simulink model "IPC4M"  (R2015a)
settings: Solver=ode3  SolverMode=SingleTasking  StartTime=0.0  StopTime=10.0  FixedStep=1e-2  RelTol=1e-7
values from neighbouring files (symbols this model uses):
  d1 = 70    [IPC4Minit.m]
  d2 = 70    [IPC4Minit.m]
  d3 = 70    [IPC4Minit.m]
  d4 = 70    [IPC4Minit.m]
  delta1 = 9    [IPC4Minit.m]
  delta2 = 9    [IPC4Minit.m]
  delta3 = 9    [IPC4Minit.m]
  delta4 = 9    [IPC4Minit.m]
  g = [0;0;-9.81]    [IPC4Minit.m]
  j0 = 10    [IPC4Minit.m]
  j1 = 10    [IPC4Minit.m]
  j1d = 1.00*j1    (= 10)    [IPC4Minit.m]
  j2 = 10    [IPC4Minit.m]
  j2d = 1.00*j2    (= 10)    [IPC4Minit.m]
  j3 = 10    [IPC4Minit.m]
  j3d = 1.00*j3    (= 10)    [IPC4Minit.m]
  j4 = 10    [IPC4Minit.m]
  j4d = 1.00*j4    (= 10)    [IPC4Minit.m]
  k1 = 2000    [IPC4Minit.m]
  k2 = 2000    [IPC4Minit.m]
  k3 = 2000    [IPC4Minit.m]
  k4 = 2000    [IPC4Minit.m]
  kappa1 = 10    [IPC4Minit.m]
  kappa2 = 10    [IPC4Minit.m]
  kappa3 = 10    [IPC4Minit.m]
  kappa4 = 10    [IPC4Minit.m]
  Kc = 150    [IPC4Minit.m]
  l = [1 1 1 1]    [IPC4Minit.m]
  m0 = 10    [IPC4Minit.m]
  m1 = 10    [IPC4Minit.m]
  m1d = 0.00*m1    (= 0)    [IPC4Minit.m]
  m2 = 10    [IPC4Minit.m]
  m2d = 0.00*m2    (= 0)    [IPC4Minit.m]
  m3 = 10    [IPC4Minit.m]
  m3d = 0.00*m3    (= 0)    [IPC4Minit.m]
  m4 = 10    [IPC4Minit.m]
  m4d = 0.00*m4    (= 0)    [IPC4Minit.m]
libraries: aerolibutil x11, dspinverses x3
(part 2 of 3)

== matlab function IPC4M/Inverse Dynamics/Weighted Generalized Inverse2 ==
  data: x input; Ginv output; r parameter
function Ginv = GraspInverse(x,r)
r1 = quatrot(x(4:7),r(1:3));
r2 = quatrot(x(4:7),r(4:6));
r3 = quatrot(x(4:7),r(7:9));
r4 = quatrot(x(4:7),r(10:12));
x1 = r1(1);
y1 = r1(2);
z1 = r1(3);
x2 = r2(1);
y2 = r2(2);
z2 = r2(3);
x3 = r3(1);
y3 = r3(2);
z3 = r3(3);
x4 = r4(1);
y4 = r4(2);
z4 = r4(3);

J4inv = [(4*(2*x1^2*x2^2 + 2*x1^2*x3^2 + 2*x1^2*x4^2 + 2*x2^2*x3^2 + 2*x2^2*x4^2 + 2*x3^2*x4^2 + x1^2*y1^2 + x1^2*y2^2 + x2^2*y1^2 + x1^2*y3^2 + x2^2*y2^2 + x3^2*y1^2 + x1^2*y4^2 + x2^2*y3^2 + x3^2*y2^2 + x4^2*y1^2 + x2^2*y4^2 + x3^2*y3^2 + x4^2*y2^2 + x3^2*y4^2 + x4^2*y3^2 + x4^2*y4^2 + x1^2*z1^2 + x1^2*z2^2 + x2^2*z1^2 + x1^2*z3^2 + x2^2*z2^2 + x3^2*z1^2 + x1^2*z4^2 + x2^2*z3^2 + x3^2*z2^2 + x4^2*z1^2 + x2^2*z4^2 + x3^2*z3^2 + x4^2*z2^2 + x3^2*z4^2 + x4^2*z3^2 + x4^2*z4^2 + y1^2*z2^2 + y2^2*z1^2 + y1^2*z3^2 + y3^2*z1^2 + y1^2*z4^2 + y2^2*z3^2 + y3^2*z2^2 + y4^2*z1^2 + y2^2*z4^2 + y4^2*z2^2 + y3^2*z4^2 + y4^2*z3^2 + 8*x1^2 + 8*x2^2 + x1^4 + 8*x3^2 + x2^4 + 8*x4^2 + x3^4 + x4^4 + 4*y1^2 + 4*y2^2 + 4*y3^2 + 4*y4^2 + 4*z1^2 + 4*z2^2 + 4*z3^2 + 4*z4^2 - 2*y1*y2*z1*z2 - 2*y1*y3*z1*z3 - 2*y1*y4*z1*z4 - 2*y2*y3*z2*z3 - 2*y2*y4*z2*z4 - 2*y3*y4*z3*z4 + 16))/(8*x1^2*x2^2 + 8*x1^2*x3^2 + 8*x1^2*x4^2 + 8*x2^2*x3^2 + 8*x2^2*x4^2 + 8*x3^2*x4^2 + 8*x1^2*y1^2 + 12*x1^2*y2^2 + 12*x2^2*y1^2 + 12*x1^2*y3^2 + 8*x2^2*y2^2 + 12*x3^2*y1^2 + x1^2*y2^4 + 12*x1^2*y4^2 + x2^2*y1^4 + 12*x2^2*y3^2 + x1^4*y2^2 + 12*x3^2*y2^2 + x2^4*y1^2 + 12*x4^2*y1^2 + x1^2*y3^4 + 12*x2^2*y4^2 + x1^4*y3^2 + x3^2*y1^4 + 8*x3^2*y3^2 + 12*x4^2*y2^2 + x3^4*y1^2 + x1^2*y4^4 + x2^2*y3^4 + x1^4*y4^2 + x3^2*y2^4 + 12*x3^2*y4^2 + x2^4*y3^2 + x4^2*y1^4 + 12*x4^2*y3^2 + x3^4*y2^2 + x4^4*y1^2 + x2^2*y4^4 + x2^4*y4^2 + x4^2*y2^4 + 8*x4^2*y4^2 + x4^4*y2^2 + x3^2*y4^4 + x4^2*y3^4 + x3^4*y4^2 + x4^4*y3^2 + 8*x1^2*z1^2 + 12*x1^2*z2^2 + 12*x2^2*z1^2 + 8*y1^2*y2^2 + 12*x1^2*z3^2 + 8*x2^2*z2^2 + 12*x3^2*z1^2 + 8*y1^2*y3^2 + x1^2*z2^4 + 12*x1^2*z4^2 + x2^2*z1^4 + 12*x2^2*z3^2 + x1^4*z2^2 + 12*x3^2*z2^2 + x2^4*z1^2 + 12*x4^2*z1^2 + 8*y1^2*y4^2 + 8*y2^2*y3^2 + x1^2*z3^4 + 12*x2^2*z4^2 + x1^4*z3^2 + x3^2*z1^4 + 8*x3^2*z3^2 + 12*x4^2*z2^2 + x3^4*z1^2 + 8*y2^2*y4^2 + x1^2*z4^4 + x2^2*z3^4 + x1^4*z4^2 + x3^2*z2^4 + 12*x3^2*z4^2 + x2^4*z3^2 + x4^2*z1^4 + 12*x4^2*z3^2 + x3^4*z2^2 + x4^4*z1^2 + 8*y3^2*y4^2 + x2^2*z4^4 + x2^4*z4^2 + x4^2*z2^4 + 8*x4^2*z4^2 + x4^4*z2^2 + x3^2*z4^4 + x4^2*z3^4 + x3^4*z4^2 + x4^4*z3^2 + 8*y1^2*z1^2 + 12*y1^2*z2^2 + 12*y2^2*z1^2 + 12*y1^2*z3^2 + 8*y2^2*z2^2 + 12*y3^2*z1^2 + y1^2*z2^4 + 12*y1^2*z4^2 + y2^2*z1^4 + 12*y2^2*z3^2 + y1^4*z2^2 + 12*y3^2*z2^2 + y2^4*z1^2 + 12*y4^2*z1^2 + y1^2*z3^4 + 12*y2^2*z4^2 + y1^4*z3^2 + y3^2*z1^4 + 8*y3^2*z3^2 + 12*y4^2*z2^2 + y3^4*z1^2 + y1^2*z4^4 + y2^2*z3^4 + y1^4*z4^2 + y3^2*z2^4 + 12*y3^2*z4^2 + y2^4*z3^2 + y4^2*z1^4 + 12*y4^2*z3^2 + y3^4*z2^2 + y4^4*z1^2 + y2^2*z4^4 + y2^4*z4^2 + y4^2*z2^4 + 8*y4^2*z4^2 + y4^4*z2^2 + y3^2*z4^4 + y4^2*z3^4 + y3^4*z4^2 + y4^4*z3^2 + 8*z1^2*z2^2 + 8*z1^2*z3^2 + 8*z1^2*z4^2 + 8*z2^2*z3^2 + 8*z2^2*z4^2 + 8*z3^2*z4^2 + 32*x1^2 + 32*x2^2 + 4*x1^4 + 32*x3^2 + 4*x2^4 + 32*x4^2 + 4*x3^4 + 4*x4^4 + 32*y1^2 + 32*y2^2 + 4*y1^4 + 32*y3^2 + 4*y2^4 + 32*y4^2 + 4*y3^4 + 4*y4^4 + 32*z1^2 + 32*z2^2 + 4*z1^4 + 32*z3^2 + 4*z2^4 + 32*z4^2 + 4*z3^4 + 4*z4^4 + x1^2*x2^2*y1^2 + x1^2*x2^2*y2^2 + x1^2*x3^2*y1^2 + 2*x1^2*x2^2*y3^2 + 2*x1^2*x3^2*y2^2 + x1^2*x4^2*y1^2 + 2*x2^2*x3^2*y1^2 + 2*x1^2*x2^2*y4^2 + x1^2*x3^2*y3^2 + 2*x1^2*x4^2*y2^2 + x2^2*x3^2*y2^2 + 2*x2^2*x4^2*y1^2 + 2*x1^2*x3^2*y4^2 + 2*x1^2*x4^2*y3^2 + x2^2*x3^2*y3^2 + x2^2*x4^2*y2^2 + 2*x3^2*x4^2*y1^2 + x1^2*x4^2*y4^2 + 2*x2^2*x3^2*y4^2 + 2*x2^2*x4^2*y3^2 + 2*x3^2*x4^2*y2^2 + x2^2*x4^2*y4^2 + x3^2*x4^2*y3^2 + x3^2*x4^2*y4^2 + x1^2*x2^2*z1^2 + x1^2*y1^2*y2^2 + x1^2*x2^2*z2^2 + x1^2*x3^2*z1^2 + x1^2*y1^2*y3^2 + x2^2*y1^2*y2^2 + 2*x1^2*x2^2*z3^2 + 2*x1^2*x3^2*z2^2 + x1^2*x4^2*z1^2 + x1^2*y1^2*y4^2 + 2*x1^2*y2^2*y3^2 + 2*x2^2*x3^2*z1^2 + 2*x2^2*y1^2*y3^2 + 2*x3^2*y1^2*y2^2 + 2*x1^2*x2^2*z4^2 + x1^2*x3^2*z3^2 + 2*x1^2*x4^2*z2^2 + 2*x1^2*y2^2*y4^2 + x2^2*x3^2*z2^2 + 2*x2^2*x4^2*z1^2 + 2*x2^2*y1^2*y4^2 + x2^2*y2^2*y3^2 + x3^2*y1^2*y3^2 + 2*x4^2*y1^2*y2^2 + 2*x1^2*x3^2*z4^2 + 2*x1^2*x4^2*z3^2 + 2*x1^2*y3^2*y4^2 + x2^2*x3^2*z3^2 + x2^2*x4^2*z2^2 + x2^2*y2^2*y4^2 + 2*x3^2*x4^2*z1^2 + 2*x3^2*y1^2*y4^2 + x3^2*y2^2*y3^2 + 2*x4^2*y1^2*y3^2 + x1^2*x4^2*z4^2 + 2*x2^2*x3^2*z4^2 + 2*x2^2*x4^2*z3^2 + 2*x2^2*y3^2*y4^2 + 2*x3^2*x4^2*z2^2 + 2*x3^2*y2^2*y4^2 + x4^2*y1^2*y4^2 + 2*x4^2*y2^2*y3^2 + x2^2*x4^2*z4^2 + x3^2*x4^2*z3^2 + x3^2*y3^2*y4^2 + x4^2*y2^2*y4^2 + x3^2*x4^2*z4^2 + x4^2*y3^2*y4^2 + 2*x1^2*y1^2*z2^2 + 2*x1^2*y2^2*z1^2 + 2*x2^2*y1^2*z1^2 + 2*x1^2*y1^2*z3^2 + 2*x1^2*y2^2*z2^2 + 2*x1^2*y3^2*z1^2 + 2*x2^2*y1^2*z2^2 + 2*x2^2*y2^2*z1^2 + 2*x3^2*y1^2*z1^2 + 2*x1^2*y1^2*z4^2 + 2*x1^2*y2^2*z3^2 + 2*x1^2*y3^2*z2^2 + 2*x1^2*y4^2*z1^2 + 2*x2^2*y1^2*z3^2 + 2*x2^2*y3^2*z1^2 + 2*x3^2*y1^2*z2^2 + 2*x3^2*y2^2*z1^2 + 2*x4^2*y1^2*z1^2 + 2*x1^2*y2^2*z4^2 + 2*x1^2*y3^2*z3^2 + 2*x1^2*y4^2*z2^2 + 2*x2^2*y1^2*z4^2 + 2*x2^2*y2^2*z3^2 + 2*x2^2*y3^2*z2^2 + 2*x2^2*y4^2*z1^2 + 2*x3^2*y1^2*z3^2 + 2*x3^2*y2^2*z2^2 + 2*x3^2*y3^2*z1^2 + 2*x4^2*y1^2*z2^2 + 2*x4^2*y2^2*z1^2 + 2*x1^2*y3^2*z4^2 + 2*x1^2*y4^2*z3^2 + 2*x2^2*y2^2*z4^2 + 2*x2^2*y3^2*z3^2 + 2*x2^2*y4^2*z2^2 + 2*x3^2*y1^2*z4^2 + 2*x3^2*y2^2*z3^2 + 2*x3^2*y3^2*z2^2 + 2*x3^2*y4^2*z1^2 + 2*x4^2*y1^2*z3^2 + 2*x4^2*y2^2*z2^2 + 2*x4^2*y3^2*z1^2 + 2*x1^2*y4^2*z4^2 + 2*x2^2*y3^2*z4^2 + 2*x2^2*y4^2*z3^2 + 2*x3^2*y2^2*z4^2 + 2*x3^2*y4^2*z2^2 + 2*x4^2*y1^2*z4^2 + 2*x4^2*y2^2*z3^2 + 2*x4^2*y3^2*z2^2 + 2*x4^2*y4^2*z1^2 + 2*x2^2*y4^2*z4^2 + 2*x3^2*y3^2*z4^2 + 2*x3^2*y4^2*z3^2 + 2*x4^2*y2^2*z4^2 + 2*x4^2*y3^2*z3^2 + 2*x4^2*y4^2*z2^2 + 2*x3^2*y4^2*z4^2 + 2*x4^2*y3^2*z4^2 + 2*x4^2*y4^2*z3^2 + x1^2*z1^2*z2^2 + y1^2*y2^2*z1^2 + x1^2*z1^2*z3^2 + x2^2*z1^2*z2^2 + y1^2*y2^2*z2^2 + y1^2*y3^2*z1^2 + x1^2*z1^2*z4^2 + 2*x1^2*z2^2*z3^2 + 2*x2^2*z1^2*z3^2 + 2*x3^2*z1^2*z2^2 + 2*y1^2*y2^2*z3^2 + 2*y1^2*y3^2*z2^2 + y1^2*y4^2*z1^2 + 2*y2^2*y3^2*z1^2 + 2*x1^2*z2^2*z4^2 + 2*x2^2*z1^2*z4^2 + x2^2*z2^2*z3^2 + x3^2*z1^2*z3^2 + 2*x4^2*z1^2*z2^2 + 2*y1^2*y2^2*z4^2 + y1^2*y3^2*z3^2 + 2*y1^2*y4^2*z2^2 + y2^2*y3^2*z2^2 + 2*y2^2*y4^2*z1^2 + 2*x1^2*z3^2*z4^2 + x2^2*z2^2*z4^2 + 2*x3^2*z1^2*z4^2 + x3^2*z2^2*z3^2 + 2*x4^2*z1^2*z3^2 + 2*y1^2*y3^2*z4^2 + 2*y1^2*y4^2*z3^2 + y2^2*y3^2*z3^2 + y2^2*y4^2*z2^2 + 2*y3^2*y4^2*z1^2 + 2*x2^2*z3^2*z4^2 + 2*x3^2*z2^2*z4^2 + x4^2*z1^2*z4^2 + 2*x4^2*z2^2*z3^2 + y1^2*y4^2*z4^2 + 2*y2^2*y3^2*z4^2 + 2*y2^2*y4^2*z3^2 + 2*y3^2*y4^2*z2^2 + x3^2*z3^2*z4^2 + x4^2*z2^2*z4^2 + y2^2*y4^2*z4^2 + y3^2*y4^2*z3^2 + x4^2*z3^2*z4^2 + y3^2*y4^2*z4^2 + y1^2*z1^2*z2^2 + y1^2*z1^2*z3^2 + y2^2*z1^2*z2^2 + y1^2*z1^2*z4^2 + 2*y1^2*z2^2*z3^2 + 2*y2^2*z1^2*z3^2 + 2*y3^2*z1^2*z2^2 + 2*y1^2*z2^2*z4^2 + 2*y2^2*z1^2*z4^2 + y2^2*z2^2*z3^2 + y3^2*z1^2*z3^2 + 2*y4^2*z1^2*z2^2 + 2*y1^2*z3^2*z4^2 + y2^2*z2^2*z4^2 + 2*y3^2*z1^2*z4^2 + y3^2*z2^2*z3^2 + 2*y4^2*z1^2*z3^2 + 2*y2^2*z3^2*z4^2 + 2*y3^2*z2^2*z4^2 + y4^2*z1^2*z4^2 + 2*y4^2*z2^2*z3^2 + y3^2*z3^2*z4^2 + y4^2*z2^2*z4^2 + y4^2*z3^2*z4^2 - 8*x1*x2*y1*y2 - 8*x1*x3*y1*y3 - 8*x1*x4*y1*y4 - 8*x2*x3*y2*y3 - 8*x2*x4*y2*y4 - 8*x3*x4*y3*y4 - 8*x1*x2*z1*z2 - 8*x1*x3*z1*z3 - 8*x1*x4*z1*z4 - 8*x2*x3*z2*z3 - 8*x2*x4*z2*z4 - 8*x3*x4*z3*z4 - 8*y1*y2*z1*z2 - 8*y1*y3*z1*z3 - 8*y1*y4*z1*z4 - 8*y2*y3*z2*z3 - 8*y2*y4*z2*z4 - 8*y3*y4*z3*z4 - 2*x1*x2*y1*y2^3 - 2*x1*x2*y1^3*y2 - 2*x1*x2^3*y1*y2 - 2*x1^3*x2*y1*y2 - 2*x1*x3*y1*y3^3 - 2*x1*x3*y1^3*y3 - 2*x1*x3^3*y1*y3 - 2*x1^3*x3*y1*y3 - 2*x1*x4*y1*y4^3 - 2*x1*x4*y1^3*y4 - 2*x1*x4^3*y1*y4 - 2*x2*x3*y2*y3^3 - 2*x2*x3*y2^3*y3 - 2*x2*x3^3*y2*y3 - 2*x1^3*x4*y1*y4 - 2*x2^3*x3*y2*y3 - 2*x2*x4*y2*y4^3 - 2*x2*x4*y2^3*y4 - 2*x2*x4^3*y2*y4 - 2*x2^3*x4*y2*y4 - 2*x3*x4*y3*y4^3 - 2*x3*x4*y3^3*y4 - 2*x3*x4^3*y3*y4 - 2*x3^3*x4*y3*y4 - 2*x1*x2*z1*z2^3 - 2*x1*x2*z1^3*z2 - 2*x1*x2^3*z1*z2 - 2*x1^3*x2*z1*z2 - 2*x1*x3*z1*z3^3 - 2*x1*x3*z1^3*z3 - 2*x1*x3^3*z1*z3 - 2*x1^3*x3*z1*z3 - 2*x1*x4*z1*z4^3 - 2*x1*x4*z1^3*z4 - 2*x1*x4^3*z1*z4 - 2*x2*x3*z2*z3^3 - 2*x2*x3*z2^3*z3 - 2*x2*x3^3*z2*z3 - 2*x1^3*x4*z1*z4 - 2*x2^3*x3*z2*z3 - 2*x2*x4*z2*z4^3 - 2*x2*x4*z2^3*z4 - 2*x2*x4^3*z2*z4 - 2*x2^3*x4*z2*z4 - 2*x3*x4*z3*z4^3 - 2*x3*x4*z3^3*z4 - 2*x3*x4^3*z3*z4 - 2*x3^3*x4*z3*z4 - 2*y1*y2*z1*z2^3 - 2*y1*y2*z1^3*z2 - 2*y1*y2^3*z1*z2 - 2*y1^3*y2*z1*z2 - 2*y1*y3*z1*z3^3 - 2*y1*y3*z1^3*z3 - 2*y1*y3^3*z1*z3 - 2*y1^3*y3*z1*z3 - 2*y1*y4*z1*z4^3 - 2*y1*y4*z1^3*z4 - 2*y1*y4^3*z1*z4 - 2*y2*y3*z2*z3^3 - 2*y2*y3*z2^3*z3 - 2*y2*y3^3*z2*z3 - 2*y1^3*y4*z1*z4 - 2*y2^3*y3*z2*z3 - 2*y2*y4*z2*z4^3 - 2*y2*y4*z2^3*z4 - 2*y2*y4^3*z2*z4 - 2*y2^3*y4*z2*z4 - 2*y3*y4*z3*z4^3 - 2*y3*y4*z3^3*z4 - 2*y3*y4^3*z3*z4 - 2*y3^3*y4*z3*z4 - 2*x1*x2*x3^2*y1*y2 - 2*x1*x2*x4^2*y1*y2 - 2*x1*x2^2*x3*y1*y3 - 2*x1^2*x2*x3*y2*y3 - 2*x1*x3*x4^2*y1*y3 - 2*x1*x2^2*x4*y1*y4 - 2*x1*x3^2*x4*y1*y4 - 2*x1^2*x2*x4*y2*y4 - 2*x2*x3*x4^2*y2*y3 - 2*x2*x3^2*x4*y2*y4 - 2*x1^2*x3*x4*y3*y4 - 2*x2^2*x3*x4*y3*y4 - 2*x1*x2*y1*y2*y3^2 - 2*x1*x2*y1*y2*y4^2 - 2*x1*x3*y1*y2^2*y3 - 2*x2*x3*y1^2*y2*y3 - 2*x1*x3*y1*y3*y4^2 - 2*x1*x4*y1*y2^2*y4 - 2*x1*x4*y1*y3^2*y4 - 2*x2*x4*y1^2*y2*y4 - 2*x2*x3*y2*y3*y4^2 - 2*x2*x4*y2*y3^2*y4 - 2*x3*x4*y1^2*y3*y4 - 2*x3*x4*y2^2*y3*y4 - 2*x1*x2*y1*y2*z1^2 - 2*x1*x2*y1*y2*z2^2 - 2*x1*x2*x3^2*z1*z2 - 2*x1*x3*y1*y3*z1^2 - 2*x1*x2*x4^2*z1*z2 - 2*x1*x2^2*x3*z1*z3 - 2*x1*x3*y1*y3*z3^2 - 2*x1*x4*y1*y4*z1^2 - 2*x1^2*x2*x3*z2*z3 - 2*x1*x3*x4^2*z1*z3 - 2*x1*x2^2*x4*z1*z4 - 2*x2*x3*y2*y3*z2^2 - 2*x1*x3^2*x4*z1*z4 - 2*x2*x3*y2*y3*z3^2 - 2*x1^2*x2*x4*z2*z4 - 2*x1*x4*y1*y4*z4^2 - 2*x2*x3*x4^2*z2*z3 - 2*x2*x4*y2*y4*z2^2 - 2*x2*x3^2*x4*z2*z4 - 2*x1^2*x3*x4*z3*z4 - 2*x2*x4*y2*y4*z4^2 - 2*x2^2*x3*x4*z3*z4 - 2*x3*x4*y3*y4*z3^2 - 2*x3*x4*y3*y4*z4^2 - 2*x1*x2*y1^2*z1*z2 - 2*x1*x2*y2^2*z1*z2 - 2*x1*x3*y1^2*z1*z3 - 2*x1*x3*y3^2*z1*z3 - 2*x1*x4*y1^2*z1*z4 - 2*x2*x3*y2^2*z2*z3 - 2*x2*x3*y3^2*z2*z3 - 2*x1*x4*y4^2*z1*z4 - 2*x2*x4*y2^2*z2*z4 - 2*x2*x4*y4^2*z2*z4 - 2*x3*x4*y3^2*z3*z4 - 2*x3*x4*y4^2*z3*z4 - 2*x1^2*y1*y2*z1*z2 - 2*x2^2*y1*y2*z1*z2 - 2*x1*x2*z1*z2*z3^2 - 2*x1^2*y1*y3*z1*z3 - 2*x1*x2*z1*z2*z4^2 - 2*x1*x3*z1*z2^2*z3 - 2*x2*x3*z1^2*z2*z3 - 2*x1^2*y1*y4*z1*z4 - 2*x3^2*y1*y3*z1*z3 - 2*x1*x3*z1*z3*z4^2 - 2*x1*x4*z1*z2^2*z4 - 2*x2^2*y2*y3*z2*z3 - 2*x1*x4*z1*z3^2*z4 - 2*x2*x4*z1^2*z2*z4 - 2*x3^2*y2*y3*z2*z3 - 2*x2*x3*z2*z3*z4^2 - 2*x2^2*y2*y4*z2*z4 - 2*x4^2*y1*y4*z1*z4 - 2*x2*x4*z2*z3^2*z4 - 2*x3*x4*z1^2*z3*z4 - 2*x3*x4*z2^2*z3*z4 - 2*x4^2*y2*y4*z2*z4 - 2*x3^2*y3*y4*z3*z4 - 2*x4^2*y3*y4*z3*z4 - 2*y1*y2*y3^2*z1*z2 - 2*y1*y2*y4^2*z1*z2 - 2*y1*y2^2*y3*z1*z3 - 2*y1^2*y2*y3*z2*z3 - 2*y1*y3*y4^2*z1*z3 - 2*y1*y2^2*y4*z1*z4 - 2*y1*y3^2*y4*z1*z4 - 2*y1^2*y2*y4*z2*z4 - 2*y2*y3*y4^2*z2*z3 - 2*y2*y3^2*y4*z2*z4 - 2*y1^2*y3*y4*z3*z4 - 2*y2^2*y3*y4*z3*z4 - 2*y1*y2*z1*z2*z3^2 - 2*y1*y2*z1*z2*z4^2 - 2*y1*y3*z1*z2^2*z3 - 2*y2*y3*z1^2*z2*z3 - 2*y1*y3*z1*z3*z4^2 - 2*y1*y4*z1*z2^2*z4 - 2*y1*y4*z1*z3^2*z4 - 2*y2*y4*z1^2*z2*z4 - 2*y2*y3*z2*z3*z4^2 - 2*y2*y4*z2*z3^2*z4 - 2*y3*y4*z1^2*z3*z4 - 2*y3*y4*z2^2*z3*z4 - 2*x1*x2*y1*y3*z2*z3 - 2*x1*x2*y2*y3*z1*z3 - 2*x1*x3*y1*y2*z2*z3 - 2*x1*x3*y2*y3*z1*z2 - 2*x2*x3*y1*y2*z1*z3 - 2*x2*x3*y1*y3*z1*z2 - 2*x1*x2*y1*y4*z2*z4 - 2*x1*x2*y2*y4*z1*z4 - 2*x1*x4*y1*y2*z2*z4 - 2*x1*x4*y2*y4*z1*z2 - 2*x2*x4*y1*y2*z1*z4 - 2*x2*x4*y1*y4*z1*z2 - 2*x1*x3*y1*y4*z3*z4 - 2*x1*x3*y3*y4*z1*z4 - 2*x1*x4*y1*y3*z3*z4 - 2*x1*x4*y3*y4*z1*z3 - 2*x3*x4*y1*y3*z1*z4 - 2*x3*x4*y1*y4*z1*z3 - 2*x2*x3*y2*y4*z3*z4 - 2*x2*x3*y3*y4*z2*z4 - 2*x2*x4*y2*y3*z3*z4 - 2*x2*x4*y3*y4*z2*z3 - 2*x3*x4*y2*y3*z2*z4 - 2*x3*x4*y2*y4*z2*z3 + 64),...
        (4*(4*x1*y1 + 4*x2*y2 + 4*x3*y3 + 4*x4*y4 + x1*y1^3 + x1^3*y1 + x2*y2^3 + x2^3*y2 + x3*y3^3 + x3^3*y3 + x4*y4^3 + x4^3*y4 + x1*x2^2*y1 + x1*x3^2*y1 + x1^2*x2*y2 + x1*x4^2*y1 + x2*x3^2*y2 + x1^2*x3*y3 + x2*x4^2*y2 + x2^2*x3*y3 + x1^2*x4*y4 + x3*x4^2*y3 + x2^2*x4*y4 + x3^2*x4*y4 + x1*y1*y2^2 + x1*y1*y3^2 + x2*y1^2*y2 + x1*y1*y4^2 + x2*y2*y3^2 + x3*y1^2*y3 + x2*y2*y4^2 + x3*y2^2*y3 + x4*y1^2*y4 + x3*y3*y4^2 + x4*y2^2*y4 + x4*y3^2*y4 + x1*y1*z1^2 + x2*y2*z2^2 + x3*y3*z3^2 + x4*y4*z4^2 + x1*y2*z1*z2 + x2*y1*z1*z2 + x1*y3*z1*z3 + x3*y1*z1*z3 + x1*y4*z1*z4 + x2*y3*z2*z3 + x3*y2*z2*z3 + x4*y1*z1*z4 + x2*y4*z2*z4 + x4*y2*z2*z4 + x3*y4*z3*z4 + x4*y3*z3*z4))/(8*x1^2*x2^2 + 8*x1^2*x3^2 + 8*x1^2*x4^2 + 8*x2^2*x3^2 + 8*x2^2*x4^2 + 8*x3^2*x4^2 + 8*x1^2*y1^2 + 12*x1^2*y2^2 + 12*x2^2*y1^2 + 12*x1^2*y3^2 + 8*x2^2*y2^2 + 12*x3^2*y1^2 + x1^2*y2^4 + 12*x1^2*y4^2 + x2^2*y1^4 + 12*x2^2*y3^2 + x1^4*y2^2 + 12*x3^2*y2^2 + x2^4*y1^2 + 12*x4^2*y1^2 + x1^2*y3^4 + 12*x2^2*y4^2 + x1^4*y3^2 + x3^2*y1^4 + 8*x3^2*y3^2 + 12*x4^2*y2^2 + x3^4*y1^2 + x1^2*y4^4 + x2^2*y3^4 + x1^4*y4^2 + x3^2*y2^4 + 12*x3^2*y4^2 + x2^4*y3^2 + x4^2*y1^4 + 12*x4^2*y3^2 + x3^4*y2^2 + x4^4*y1^2 + x2^2*y4^4 + x2^4*y4^2 + x4^2*y2^4 + 8*x4^2*y4^2 + x4^4*y2^2 + x3^2*y4^4 + x4^2*y3^4 + x3^4*y4^2 + x4^4*y3^2 + 8*x1^2*z1^2 + 12*x1^2*z2^2 + 12*x2^2*z1^2 + 8*y1^2*y2^2 + 12*x1^2*z3^2 + 8*x2^2*z2^2 + 12*x3^2*z1^2 + 8*y1^2*y3^2 + x1^2*z2^4 + 12*x1^2*z4^2 + x2^2*z1^4 + 12*x2^2*z3^2 + x1^4*z2^2 + 12*x3^2*z2^2 + x2^4*z1^2 + 12*x4^2*z1^2 + 8*y1^2*y4^2 + 8*y2^2*y3^2 + x1^2*z3^4 + 12*x2^2*z4^2 + x1^4*z3^2 + x3^2*z1^4 + 8*x3^2*z3^2 + 12*x4^2*z2^2 + x3^4*z1^2 + 8*y2^2*y4^2 + x1^2*z4^4 + x2^2*z3^4 + x1^4*z4^2 + x3^2*z2^4 + 12*x3^2*z4^2 + x2^4*z3^2 + x4^2*z1^4 + 12*x4^2*z3^2 + x3^4*z2^2 + x4^4*z1^2 + 8*y3^2*y4^2 + x2^2*z4^4 + x2^4*z4^2 + x4^2*z2^4 + 8*x4^2*z4^2 + x4^4*z2^2 + x3^2*z4^4 + x4^2*z3^4 + x3^4*z4^2 + x4^4*z3^2 + 8*y1^2*z1^2 + 12*y1^2*z2^2 + 12*y2^2*z1^2 + 12*y1^2*z3^2 + 8*y2^2*z2^2 + 12*y3^2*z1^2 + y1^2*z2^4 + 12*y1^2*z4^2 + y2^2*z1^4 + 12*y2^2*z3^2 + y1^4*z2^2 + 12*y3^2*z2^2 + y2^4*z1^2 + 12*y4^2*z1^2 + y1^2*z3^4 + 12*y2^2*z4^2 + y1^4*z3^2 + y3^2*z1^4 + 8*y3^2*z3^2 + 12*y4^2*z2^2 + y3^4*z1^2 + y1^2*z4^4 + y2^2*z3^4 + y1^4*z4^2 + y3^2*z2^4 + 12*y3^2*z4^2 + y2^4*z3^2 + y4^2*z1^4 + 12*y4^2*z3^2 + y3^4*z2^2 + y4^4*z1^2 + y2^2*z4^4 + y2^4*z4^2 + y4^2*z2^4 + 8*y4^2*z4^2 + y4^4*z2^2 + y3^2*z4^4 + y4^2*z3^4 + y3^4*z4^2 + y4^4*z3^2 + 8*z1^2*z2^2 + 8*z1^2*z3^2 + 8*z1^2*z4^2 + 8*z2^2*z3^2 + 8*z2^2*z4^2 + 8*z3^2*z4^2 + 32*x1^2 + 32*x2^2 + 4*x1^4 + 32*x3^2 + 4*x2^4 + 32*x4^2 + 4*x3^4 + 4*x4^4 + 32*y1^2 + 32*y2^2 + 4*y1^4 + 32*y3^2 + 4*y2^4 + 32*y4^2 + 4*y3^4 + 4*y4^4 + 32*z1^2 + 32*z2^2 + 4*z1^4 + 32*z3^2 + 4*z2^4 + 32*z4^2 + 4*z3^4 + 4*z4^4 + x1^2*x2^2*y1^2 + x1^2*x2^2*y2^2 + x1^2*x3^2*y1^2 + 2*x1^2*x2^2*y3^2 + 2*x1^2*x3^2*y2^2 + x1^2*x4^2*y1^2 + 2*x2^2*x3^2*y1^2 + 2*x1^2*x2^2*y4^2 + x1^2*x3^2*y3^2 + 2*x1^2*x4^2*y2^2 + x2^2*x3^2*y2^2 + 2*x2^2*x4^2*y1^2 + 2*x1^2*x3^2*y4^2 + 2*x1^2*x4^2*y3^2 + x2^2*x3^2*y3^2 + x2^2*x4^2*y2^2 + 2*x3^2*x4^2*y1^2 + x1^2*x4^2*y4^2 + 2*x2^2*x3^2*y4^2 + 2*x2^2*x4^2*y3^2 + 2*x3^2*x4^2*y2^2 + x2^2*x4^2*y4^2 + x3^2*x4^2*y3^2 + x3^2*x4^2*y4^2 + x1^2*x2^2*z1^2 + x1^2*y1^2*y2^2 + x1^2*x2^2*z2^2 + x1^2*x3^2*z1^2 + x1^2*y1^2*y3^2 + x2^2*y1^2*y2^2 + 2*x1^2*x2^2*z3^2 + 2*x1^2*x3^2*z2^2 + x1^2*x4^2*z1^2 + x1^2*y1^2*y4^2 + 2*x1^2*y2^2*y3^2 + 2*x2^2*x3^2*z1^2 + 2*x2^2*y1^2*y3^2 + 2*x3^2*y1^2*y2^2 + 2*x1^2*x2^2*z4^2 + x1^2*x3^2*z3^2 + 2*x1^2*x4^2*z2^2 + 2*x1^2*y2^2*y4^2 + x2^2*x3^2*z2^2 + 2*x2^2*x4^2*z1^2 + 2*x2^2*y1^2*y4^2 + x2^2*y2^2*y3^2 + x3^2*y1^2*y3^2 + 2*x4^2*y1^2*y2^2 + 2*x1^2*x3^2*z4^2 + 2*x1^2*x4^2*z3^2 + 2*x1^2*y3^2*y4^2 + x2^2*x3^2*z3^2 + x2^2*x4^2*z2^2 + x2^2*y2^2*y4^2 + 2*x3^2*x4^2*z1^2 + 2*x3^2*y1^2*y4^2 + x3^2*y2^2*y3^2 + 2*x4^2*y1^2*y3^2 + x1^2*x4^2*z4^2 + 2*x2^2*x3^2*z4^2 + 2*x2^2*x4^2*z3^2 + 2*x2^2*y3^2*y4^2 + 2*x3^2*x4^2*z2^2 + 2*x3^2*y2^2*y4^2 + x4^2*y1^2*y4^2 + 2*x4^2*y2^2*y3^2 + x2^2*x4^2*z4^2 + x3^2*x4^2*z3^2 + x3^2*y3^2*y4^2 + x4^2*y2^2*y4^2 + x3^2*x4^2*z4^2 + x4^2*y3^2*y4^2 + 2*x1^2*y1^2*z2^2 + 2*x1^2*y2^2*z1^2 + 2*x2^2*y1^2*z1^2 + 2*x1^2*y1^2*z3^2 + 2*x1^2*y2^2*z2^2 + 2*x1^2*y3^2*z1^2 + 2*x2^2*y1^2*z2^2 + 2*x2^2*y2^2*z1^2 + 2*x3^2*y1^2*z1^2 + 2*x1^2*y1^2*z4^2 + 2*x1^2*y2^2*z3^2 + 2*x1^2*y3^2*z2^2 + 2*x1^2*y4^2*z1^2 + 2*x2^2*y1^2*z3^2 + 2*x2^2*y3^2*z1^2 + 2*x3^2*y1^2*z2^2 + 2*x3^2*y2^2*z1^2 + 2*x4^2*y1^2*z1^2 + 2*x1^2*y2^2*z4^2 + 2*x1^2*y3^2*z3^2 + 2*x1^2*y4^2*z2^2 + 2*x2^2*y1^2*z4^2 + 2*x2^2*y2^2*z3^2 + 2*x2^2*y3^2*z2^2 + 2*x2^2*y4^2*z1^2 + 2*x3^2*y1^2*z3^2 + 2*x3^2*y2^2*z2^2 + 2*x3^2*y3^2*z1^2 + 2*x4^2*y1^2*z2^2 + 2*x4^2*y2^2*z1^2 + 2*x1^2*y3^2*z4^2 + 2*x1^2*y4^2*z3^2 + 2*x2^2*y2^2*z4^2 + 2*x2^2*y3^2*z3^2 + 2*x2^2*y4^2*z2^2 + 2*x3^2*y1^2*z4^2 + 2*x3^2*y2^2*z3^2 + 2*x3^2*y3^2*z2^2 + 2*x3^2*y4^2*z1^2 + 2*x4^2*y1^2*z3^2 + 2*x4^2*y2^2*z2^2 + 2*x4^2*y3^2*z1^2 + 2*x1^2*y4^2*z4^2 + 2*x2^2*y3^2*z4^2 + 2*x2^2*y4^2*z3^2 + 2*x3^2*y2^2*z4^2 + 2*x3^2*y4^2*z2^2 + 2*x4^2*y1^2*z4^2 + 2*x4^2*y2^2*z3^2 + 2*x4^2*y3^2*z2^2 + 2*x4^2*y4^2*z1^2 + 2*x2^2*y4^2*z4^2 + 2*x3^2*y3^2*z4^2 + 2*x3^2*y4^2*z3^2 + 2*x4^2*y2^2*z4^2 + 2*x4^2*y3^2*z3^2 + 2*x4^2*y4^2*z2^2 + 2*x3^2*y4^2*z4^2 + 2*x4^2*y3^2*z4^2 + 2*x4^2*y4^2*z3^2 + x1^2*z1^2*z2^2 + y1^2*y2^2*z1^2 + x1^2*z1^2*z3^2 + x2^2*z1^2*z2^2 + y1^2*y2^2*z2^2 + y1^2*y3^2*z1^2 + x1^2*z1^2*z4^2 + 2*x1^2*z2^2*z3^2 + 2*x2^2*z1^2*z3^2 + 2*x3^2*z1^2*z2^2 + 2*y1^2*y2^2*z3^2 + 2*y1^2*y3^2*z2^2 + y1^2*y4^2*z1^2 + 2*y2^2*y3^2*z1^2 + 2*x1^2*z2^2*z4^2 + 2*x2^2*z1^2*z4^2 + x2^2*z2^2*z3^2 + x3^2*z1^2*z3^2 + 2*x4^2*z1^2*z2^2 + 2*y1^2*y2^2*z4^2 + y1^2*y3^2*z3^2 + 2*y1^2*y4^2*z2^2 + y2^2*y3^2*z2^2 + 2*y2^2*y4^2*z1^2 + 2*x1^2*z3^2*z4^2 + x2^2*z2^2*z4^2 + 2*x3^2*z1^2*z4^2 + x3^2*z2^2*z3^2 + 2*x4^2*z1^2*z3^2 + 2*y1^2*y3^2*z4^2 + 2*y1^2*y4^2*z3^2 + y2^2*y3^2*z3^2 + y2^2*y4^2*z2^2 + 2*y3^2*y4^2*z1^2 + 2*x2^2*z3^2*z4^2 + 2*x3^2*z2^2*z4^2 + x4^2*z1^2*z4^2 + 2*x4^2*z2^2*z3^2 + y1^2*y4^2*z4^2 + 2*y2^2*y3^2*z4^2 + 2*y2^2*y4^2*z3^2 + 2*y3^2*y4^2*z2^2 + x3^2*z3^2*z4^2 + x4^2*z2^2*z4^2 + y2^2*y4^2*z4^2 + y3^2*y4^2*z3^2 + x4^2*z3^2*z4^2 + y3^2*y4^2*z4^2 + y1^2*z1^2*z2^2 + y1^2*z1^2*z3^2 + y2^2*z1^2*z2^2 + y1^2*z1^2*z4^2 + 2*y1^2*z2^2*z3^2 + 2*y2^2*z1^2*z3^2 + 2*y3^2*z1^2*z2^2 + 2*y1^2*z2^2*z4^2 + 2*y2^2*z1^2*z4^2 + y2^2*z2^2*z3^2 + y3^2*z1^2*z3^2 + 2*y4^2*z1^2*z2^2 + 2*y1^2*z3^2*z4^2 + y2^2*z2^2*z4^2 + 2*y3^2*z1^2*z4^2 + y3^2*z2^2*z3^2 + 2*y4^2*z1^2*z3^2 + 2*y2^2*z3^2*z4^2 + 2*y3^2*z2^2*z4^2 + y4^2*z1^2*z4^2 + 2*y4^2*z2^2*z3^2 + y3^2*z3^2*z4^2 + y4^2*z2^2*z4^2 + y4^2*z3^2*z4^2 - 8*x1*x2*y1*y2 - 8*x1*x3*y1*y3 - 8*x1*x4*y1*y4 - 8*x2*x3*y2*y3 - 8*x2*x4*y2*y4 - 8*x3*x4*y3*y4 - 8*x1*x2*z1*z2 - 8*x1*x3*z1*z3 - 8*x1*x4*z1*z4 - 8*x2*x3*z2*z3 - 8*x2*x4*z2*z4 - 8*x3*x4*z3*z4 - 8*y1*y2*z1*z2 - 8*y1*y3*z1*z3 - 8*y1*y4*z1*z4 - 8*y2*y3*z2*z3 - 8*y2*y4*z2*z4 - 8*y3*y4*z3*z4 - 2*x1*x2*y1*y2^3 - 2*x1*x2*y1^3*y2 - 2*x1*x2^3*y1*y2 - 2*x1^3*x2*y1*y2 - 2*x1*x3*y1*y3^3 - 2*x1*x3*y1^3*y3 - 2*x1*x3^3*y1*y3 - 2*x1^3*x3*y1*y3 - 2*x1*x4*y1*y4^3 - 2*x1*x4*y1^3*y4 - 2*x1*x4^3*y1*y4 - 2*x2*x3*y2*y3^3 - 2*x2*x3*y2^3*y3 - 2*x2*x3^3*y2*y3 - 2*x1^3*x4*y1*y4 - 2*x2^3*x3*y2*y3 - 2*x2*x4*y2*y4^3 - 2*x2*x4*y2^3*y4 - 2*x2*x4^3*y2*y4 - 2*x2^3*x4*y2*y4 - 2*x3*x4*y3*y4^3 - 2*x3*x4*y3^3*y4 - 2*x3*x4^3*y3*y4 - 2*x3^3*x4*y3*y4 - 2*x1*x2*z1*z2^3 - 2*x1*x2*z1^3*z2 - 2*x1*x2^3*z1*z2 - 2*x1^3*x2*z1*z2 - 2*x1*x3*z1*z3^3 - 2*x1*x3*z1^3*z3 - 2*x1*x3^3*z1*z3 - 2*x1^3*x3*z1*z3 - 2*x1*x4*z1*z4^3 - 2*x1*x4*z1^3*z4 - 2*x1*x4^3*z1*z4 - 2*x2*x3*z2*z3^3 - 2*x2*x3*z2^3*z3 - 2*x2*x3^3*z2*z3 - 2*x1^3*x4*z1*z4 - 2*x2^3*x3*z2*z3 - 2*x2*x4*z2*z4^3 - 2*x2*x4*z2^3*z4 - 2*x2*x4^3*z2*z4 - 2*x2^3*x4*z2*z4 - 2*x3*x4*z3*z4^3 - 2*x3*x4*z3^3*z4 - 2*x3*x4^3*z3*z4 - 2*x3^3*x4*z3*z4 - 2*y1*y2*z1*z2^3 - 2*y1*y2*z1^3*z2 - 2*y1*y2^3*z1*z2 - 2*y1^3*y2*z1*z2 - 2*y1*y3*z1*z3^3 - 2*y1*y3*z1^3*z3 - 2*y1*y3^3*z1*z3 - 2*y1^3*y3*z1*z3 - 2*y1*y4*z1*z4^3 - 2*y1*y4*z1^3*z4 - 2*y1*y4^3*z1*z4 - 2*y2*y3*z2*z3^3 - 2*y2*y3*z2^3*z3 - 2*y2*y3^3*z2*z3 - 2*y1^3*y4*z1*z4 - 2*y2^3*y3*z2*z3 - 2*y2*y4*z2*z4^3 - 2*y2*y4*z2^3*z4 - 2*y2*y4^3*z2*z4 - 2*y2^3*y4*z2*z4 - 2*y3*y4*z3*z4^3 - 2*y3*y4*z3^3*z4 - 2*y3*y4^3*z3*z4 - 2*y3^3*y4*z3*z4 - 2*x1*x2*x3^2*y1*y2 - 2*x1*x2*x4^2*y1*y2 - 2*x1*x2^2*x3*y1*y3 - 2*x1^2*x2*x3*y2*y3 - 2*x1*x3*x4^2*y1*y3 - 2*x1*x2^2*x4*y1*y4 - 2*x1*x3^2*x4*y1*y4 - 2*x1^2*x2*x4*y2*y4 - 2*x2*x3*x4^2*y2*y3 - 2*x2*x3^2*x4*y2*y4 - 2*x1^2*x3*x4*y3*y4 - 2*x2^2*x3*x4*y3*y4 - 2*x1*x2*y1*y2*y3^2 - 2*x1*x2*y1*y2*y4^2 - 2*x1*x3*y1*y2^2*y3 - 2*x2*x3*y1^2*y2*y3 - 2*x1*x3*y1*y3*y4^2 - 2*x1*x4*y1*y2^2*y4 - 2*x1*x4*y1*y3^2*y4 - 2*x2*x4*y1^2*y2*y4 - 2*x2*x3*y2*y3*y4^2 - 2*x2*x4*y2*y3^2*y4 - 2*x3*x4*y1^2*y3*y4 - 2*x3*x4*y2^2*y3*y4 - 2*x1*x2*y1*y2*z1^2 - 2*x1*x2*y1*y2*z2^2 - 2*x1*x2*x3^2*z1*z2 - 2*x1*x3*y1*y3*z1^2 - 2*x1*x2*x4^2*z1*z2 - 2*x1*x2^2*x3*z1*z3 - 2*x1*x3*y1*y3*z3^2 - 2*x1*x4*y1*y4*z1^2 - 2*x1^2*x2*x3*z2*z3 - 2*x1*x3*x4^2*z1*z3 - 2*x1*x2^2*x4*z1*z4 - 2*x2*x3*y2*y3*z2^2 - 2*x1*x3^2*x4*z1*z4 - 2*x2*x3*y2*y3*z3^2 - 2*x1^2*x2*x4*z2*z4 - 2*x1*x4*y1*y4*z4^2 - 2*x2*x3*x4^2*z2*z3 - 2*x2*x4*y2*y4*z2^2 - 2*x2*x3^2*x4*z2*z4 - 2*x1^2*x3*x4*z3*z4 - 2*x2*x4*y2*y4*z4^2 - 2*x2^2*x3*x4*z3*z4 - 2*x3*x4*y3*y4*z3^2 - 2*x3*x4*y3*y4*z4^2 - 2*x1*x2*y1^2*z1*z2 - 2*x1*x2*y2^2*z1*z2 - 2*x1*x3*y1^2*z1*z3 - 2*x1*x3*y3^2*z1*z3 - 2*x1*x4*y1^2*z1*z4 - 2*x2*x3*y2^2*z2*z3 - 2*x2*x3*y3^2*z2*z3 - 2*x1*x4*y4^2*z1*z4 - 2*x2*x4*y2^2*z2*z4 - 2*x2*x4*y4^2*z2*z4 - 2*x3*x4*y3^2*z3*z4 - 2*x3*x4*y4^2*z3*z4 - 2*x1^2*y1*y2*z1*z2 - 2*x2^2*y1*y2*z1*z2 - 2*x1*x2*z1*z2*z3^2 - 2*x1^2*y1*y3*z1*z3 - 2*x1*x2*z1*z2*z4^2 - 2*x1*x3*z1*z2^2*z3 - 2*x2*x3*z1^2*z2*z3 - 2*x1^2*y1*y4*z1*z4 - 2*x3^2*y1*y3*z1*z3 - 2*x1*x3*z1*z3*z4^2 - 2*x1*x4*z1*z2^2*z4 - 2*x2^2*y2*y3*z2*z3 - 2*x1*x4*z1*z3^2*z4 - 2*x2*x4*z1^2*z2*z4 - 2*x3^2*y2*y3*z2*z3 - 2*x2*x3*z2*z3*z4^2 - 2*x2^2*y2*y4*z2*z4 - 2*x4^2*y1*y4*z1*z4 - 2*x2*x4*z2*z3^2*z4 - 2*x3*x4*z1^2*z3*z4 - 2*x3*x4*z2^2*z3*z4 - 2*x4^2*y2*y4*z2*z4 - 2*x3^2*y3*y4*z3*z4 - 2*x4^2*y3*y4*z3*z4 - 2*y1*y2*y3^2*z1*z2 - 2*y1*y2*y4^2*z1*z2 - 2*y1*y2^2*y3*z1*z3 - 2*y1^2*y2*y3*z2*z3 - 2*y1*y3*y4^2*z1*z3 - 2*y1*y2^2*y4*z1*z4 - 2*y1*y3^2*y4*z1*z4 - 2*y1^2*y2*y4*z2*z4 - 2*y2*y3*y4^2*z2*z3 - 2*y2*y3^2*y4*z2*z4 - 2*y1^2*y3*y4*z3*z4 - 2*y2^2*y3*y4*z3*z4 - 2*y1*y2*z1*z2*z3^2 - 2*y1*y2*z1*z2*z4^2 - 2*y1*y3*z1*z2^2*z3 - 2*y2*y3*z1^2*z2*z3 - 2*y1*y3*z1*z3*z4^2 - 2*y1*y4*z1*z2^2*z4 - 2*y1*y4*z1*z3^2*z4 - 2*y2*y4*z1^2*z2*z4 - 2*y2*y3*z2*z3*z4^2 - 2*y2*y4*z2*z3^2*z4 - 2*y3*y4*z1^2*z3*z4 - 2*y3*y4*z2^2*z3*z4 - 2*x1*x2*y1*y3*z2*z3 - 2*x1*x2*y2*y3*z1*z3 - 2*x1*x3*y1*y2*z2*z3 - 2*x1*x3*y2*y3*z1*z2 - 2*x2*x3*y1*y2*z1*z3 - 2*x2*x3*y1*y3*z1*z2 - 2*x1*x2*y1*y4*z2*z4 - 2*x1*x2*y2*y4*z1*z4 - 2*x1*x4*y1*y2*z2*z4 - 2*x1*x4*y2*y4*z1*z2 - 2*x2*x4*y1*y2*z1*z4 - 2*x2*x4*y1*y4*z1*z2 - 2*x1*x3*y1*y4*z3*z4 - 2*x1*x3*y3*y4*z1*z4 - 2*x1*x4*y1*y3*z3*z4 - 2*x1*x4*y3*y4*z1*z3 - 2*x3*x4*y1*y3*z1*z4 - 2*x3*x4*y1*y4*z1*z3 - 2*x2*x3*y2*y4*z3*z4 - 2*x2*x3*y3*y4*z2*z4 - 2*x2*x4*y2*y3*z3*z4 - 2*x2*x4*y3*y4*z2*z3 - 2*x3*x4*y2*y3*z2*z4 - 2*x3*x4*y2*y4*z2*z3 + 64),...
        (4*(4*x1*z1 + 4*x2*z2 + 4*x3*z3 + 4*x4*z4 + x1*z1^3 + x1^3*z1 + x2*z2^3 + x2^3*z2 + x3*z3^3 + x3^3*z3 + x4*z4^3 + x4^3*z4 + x1*x2^2*z1 + x1*x3^2*z1 + x1^2*x2*z2 + x1*x4^2*z1 + x2*x3^2*z2 + x1^2*x3*z3 + x2*x4^2*z2 + x2^2*x3*z3 + x1^2*x4*z4 + x3*x4^2*z3 + x2^2*x4*z4 + x3^2*x4*z4 + x1*y1^2*z1 + x2*y2^2*z2 + x3*y3^2*z3 + x4*y4^2*z4 + x1*z1*z2^2 + x1*z1*z3^2 + x2*z1^2*z2 + x1*z1*z4^2 + x2*z2*z3^2 + x3*z1^2*z3 + x2*z2*z4^2 + x3*z2^2*z3 + x4*z1^2*z4 + x3*z3*z4^2 + x4*z2^2*z4 + x4*z3^2*z4 + x1*y1*y2*z2 + x2*y1*y2*z1 + x1*y1*y3*z3 + x3*y1*y3*z1 + x1*y1*y4*z4 + x2*y2*y3*z3 + x3*y2*y3*z2 + x4*y1*y4*z1 + x2*y2*y4*z4 + x4*y2*y4*z2 + x3*y3*y4*z4 + x4*y3*y4*z3))/(8*x1^2*x2^2 + 8*x1^2*x3^2 + 8*x1^2*x4^2 + 8*x2^2*x3^2 + 8*x2^2*x4^2 + 8*x3^2*x4^2 + 8*x1^2*y1^2 + 12*x1^2*y2^2 + 12*x2^2*y1^2 + 12*x1^2*y3^2 + 8*x2^2*y2^2 + 12*x3^2*y1^2 + x1^2*y2^4 + 12*x1^2*y4^2 + x2^2*y1^4 + 12*x2^2*y3^2 + x1^4*y2^2 + 12*x3^2*y2^2 + x2^4*y1^2 + 12*x4^2*y1^2 + x1^2*y3^4 + 12*x2^2*y4^2 + x1^4*y3^2 + x3^2*y1^4 + 8*x3^2*y3^2 + 12*x4^2*y2^2 + x3^4*y1^2 + x1^2*y4^4 + x2^2*y3^4 + x1^4*y4^2 + x3^2*y2^4 + 12*x3^2*y4^2 + x2^4*y3^2 + x4^2*y1^4 + 12*x4^2*y3^2 + x3^4*y2^2 + x4^4*y1^2 + x2^2*y4^4 + x2^4*y4^2 + x4^2*y2^4 + 8*x4^2*y4^2 + x4^4*y2^2 + x3^2*y4^4 + x4^2*y3^4 + x3^4*y4^2 + x4^4*y3^2 + 8*x1^2*z1^2 + 12*x1^2*z2^2 + 12*x2^2*z1^2 + 8*y1^2*y2^2 + 12*x1^2*z3^2 + 8*x2^2*z2^2 + 12*x3^2*z1^2 + 8*y1^2*y3^2 + x1^2*z2^4 + 12*x1^2*z4^2 + x2^2*z1^4 + 12*x2^2*z3^2 + x1^4*z2^2 + 12*x3^2*z2^2 + x2^4*z1^2 + 12*x4^2*z1^2 + 8*y1^2*y4^2 + 8*y2^2*y3^2 + x1^2*z3^4 + 12*x2^2*z4^2 + x1^4*z3^2 + x3^2*z1^4 + 8*x3^2*z3^2 + 12*x4^2*z2^2 + x3^4*z1^2 + 8*y2^2*y4^2 + x1^2*z4^4 + x2^2*z3^4 + x1^4*z4^2 + x3^2*z2^4 + 12*x3^2*z4^2 + x2^4*z3^2 + x4^2*z1^4 + 12*x4^2*z3^2 + x3^4*z2^2 + x4^4*z1^2 + 8*y3^2*y4^2 + x2^2*z4^4 + x2^4*z4^2 + x4^2*z2^4 + 8*x4^2*z4^2 + x4^4*z2^2 + x3^2*z4^4 + x4^2*z3^4 + x3^4*z4^2 + x4^4*z3^2 + 8*y1^2*z1^2 + 12*y1^2*z2^2 + 12*y2^2*z1^2 + 12*y1^2*z3^2 + 8*y2^2*z2^2 + 12*y3^2*z1^2 + y1^2*z2^4 + 12*y1^2*z4^2 + y2^2*z1^4 + 12*y2^2*z3^2 + y1^4*z2^2 + 12*y3^2*z2^2 + y2^4*z1^2 + 12*y4^2*z1^2 + y1^2*z3^4 + 12*y2^2*z4^2 + y1^4*z3^2 + y3^2*z1^4 + 8*y3^2*z3^2 + 12*y4^2*z2^2 + y3^4*z1^2 + y1^2*z4^4 + y2^2*z3^4 + y1^4*z4^2 + y3^2*z2^4 + 12*y3^2*z4^2 + y2^4*z3^2 + y4^2*z1^4 + 12*y4^2*z3^2 + y3^4*z2^2 + y4^4*z1^2 + y2^2*z4^4 + y2^4*z4^2 + y4^2*z2^4 + 8*y4^2*z4^2 + y4^4*z2^2 + y3^2*z4^4 + y4^2*z3^4 + y3^4*z4^2 + y4^4*z3^2 + 8*z1^2*z2^2 + 8*z1^2*z3^2 + 8*z1^2*z4^2 + 8*z2^2*z3^2 + 8*z2^2*z4^2 + 8*z3^2*z4^2 + 32*x1^2 + 32*x2^2 + 4*x1^4 + 32*x3^2 + 4*x2^4 + 32*x4^2 + 4*x3^4 + 4*x4^4 + 32*y1^2 + 32*y2^2 + 4*y1^4 + 32*y3^2 + 4*y2^4 + 32*y4^2 + 4*y3^4 + 4*y4^4 + 32*z1^2 + 32*z2^2 + 4*z1^4 + 32*z3^2 + 4*z2^4 + 32*z4^2 + 4*z3^4 + 4*z4^4 + x1^2*x2^2*y1^2 + x1^2*x2^2*y2^2 + x1^2*x3^2*y1^2 + 2*x1^2*x2^2*y3^2 + 2*x1^2*x3^2*y2^2 + x1^2*x4^2*y1^2 + 2*x2^2*x3^2*y1^2 + 2*x1^2*x2^2*y4^2 + x1^2*x3^2*y3^2 + 2*x1^2*x4^2*y2^2 + x2^2*x3^2*y2^2 + 2*x2^2*x4^2*y1^2 + 2*x1^2*x3^2*y4^2 + 2*x1^2*x4^2*y3^2 + x2^2*x3^2*y3^2 + x2^2*x4^2*y2^2 + 2*x3^2*x4^2*y1^2 + x1^2*x4^2*y4^2 + 2*x2^2*x3^2*y4^2 + 2*x2^2*x4^2*y3^2 + 2*x3^2*x4^2*y2^2 + x2^2*x4^2*y4^2 + x3^2*x4^2*y3^2 + x3^2*x4^2*y4^2 + x1^2*x2^2*z1^2 + x1^2*y1^2*y2^2 + x1^2*x2^2*z2^2 + x1^2*x3^2*z1^2 + x1^2*y1^2*y3^2 + x2^2*y1^2*y2^2 + 2*x1^2*x2^2*z3^2 + 2*x1^2*x3^2*z2^2 + x1^2*x4^2*z1^2 + x1^2*y1^2*y4^2 + 2*x1^2*y2^2*y3^2 + 2*x2^2*x3^2*z1^2 + 2*x2^2*y1^2*y3^2 + 2*x3^2*y1^2*y2^2 + 2*x1^2*x2^2*z4^2 + x1^2*x3^2*z3^2 + 2*x1^2*x4^2*z2^2 + 2*x1^2*y2^2*y4^2 + x2^2*x3^2*z2^2 + 2*x2^2*x4^2*z1^2 + 2*x2^2*y1^2*y4^2 + x2^2*y2^2*y3^2 + x3^2*y1^2*y3^2 + 2*x4^2*y1^2*y2^2 + 2*x1^2*x3^2*z4^2 + 2*x1^2*x4^2*z3^2 + 2*x1^2*y3^2*y4^2 + x2^2*x3^2*z3^2 + x2^2*x4^2*z2^2 + x2^2*y2^2*y4^2 + 2*x3^2*x4^2*z1^2 + 2*x3^2*y1^2*y4^2 + x3^2*y2^2*y3^2 + 2*x4^2*y1^2*y3^2 + x1^2*x4^2*z4^2 + 2*x2^2*x3^2*z4^2 + 2*x2^2*x4^2*z3^2 + 2*x2^2*y3^2*y4^2 + 2*x3^2*x4^2*z2^2 + 2*x3^2*y2^2*y4^2 + x4^2*y1^2*y4^2 + 2*x4^2*y2^2*y3^2 + x2^2*x4^2*z4^2 + x3^2*x4^2*z3^2 + x3^2*y3^2*y4^2 + x4^2*y2^2*y4^2 + x3^2*x4^2*z4^2 + x4^2*y3^2*y4^2 + 2*x1^2*y1^2*z2^2 + 2*x1^2*y2^2*z1^2 + 2*x2^2*y1^2*z1^2 + 2*x1^2*y1^2*z3^2 + 2*x1^2*y2^2*z2^2 + 2*x1^2*y3^2*z1^2 + 2*x2^2*y1^2*z2^2 + 2*x2^2*y2^2*z1^2 + 2*x3^2*y1^2*z1^2 + 2*x1^2*y1^2*z4^2 + 2*x1^2*y2^2*z3^2 + 2*x1^2*y3^2*z2^2 + 2*x1^2*y4^2*z1^2 + 2*x2^2*y1^2*z3^2 + 2*x2^2*y3^2*z1^2 + 2*x3^2*y1^2*z2^2 + 2*x3^2*y2^2*z1^2 + 2*x4^2*y1^2*z1^2 + 2*x1^2*y2^2*z4^2 + 2*x1^2*y3^2*z3^2 + 2*x1^2*y4^2*z2^2 + 2*x2^2*y1^2*z4^2 + 2*x2^2*y2^2*z3^2 + 2*x2^2*y3^2*z2^2 + 2*x2^2*y4^2*z1^2 + 2*x3^2*y1^2*z3^2 + 2*x3^2*y2^2*z2^2 + 2*x3^2*y3^2*z1^2 + 2*x4^2*y1^2*z2^2 + 2*x4^2*y2^2*z1^2 + 2*x1^2*y3^2*z4^2 + 2*x1^2*y4^2*z3^2 + 2*x2^2*y2^2*z4^2 + 2*x2^2*y3^2*z3^2 + 2*x2^2*y4^2*z2^2 + 2*x3^2*y1^2*z4^2 + 2*x3^2*y2^2*z3^2 + 2*x3^2*y3^2*z2^2 + 2*x3^2*y4^2*z1^2 + 2*x4^2*y1^2*z3^2 + 2*x4^2*y2^2*z2^2 + 2*x4^2*y3^2*z1^2 + 2*x1^2*y4^2*z4^2 + 2*x2^2*y3^2*z4^2 + 2*x2^2*y4^2*z3^2 + 2*x3^2*y2^2*z4^2 + 2*x3^2*y4^2*z2^2 + 2*x4^2*y1^2*z4^2 + 2*x4^2*y2^2*z3^2 + 2*x4^2*y3^2*z2^2 + 2*x4^2*y4^2*z1^2 + 2*x2^2*y4^2*z4^2 + 2*x3^2*y3^2*z4^2 + 2*x3^2*y4^2*z3^2 + 2*x4^2*y2^2*z4^2 + 2*x4^2*y3^2*z3^2 + 2*x4^2*y4^2*z2^2 + 2*x3^2*y4^2*z4^2 + 2*x4^2*y3^2*z4^2 + 2*x4^2*y4^2*z3^2 + x1^2*z1^2*z2^2 + y1^2*y2^2*z1^2 + x1^2*z1^2*z3^2 + x2^2*z1^2*z2^2 + y1^2*y2^2*z2^2 + y1^2*y3^2*z1^2 + x1^2*z1^2*z4^2 + 2*x1^2*z2^2*z3^2 + 2*x2^2*z1^2*z3^2 + 2*x3^2*z1^2*z2^2 + 2*y1^2*y2^2*z3^2 + 2*y1^2*y3^2*z2^2 + y1^2*y4^2*z1^2 + 2*y2^2*y3^2*z1^2 + 2*x1^2*z2^2*z4^2 + 2*x2^2*z1^2*z4^2 + x2^2*z2^2*z3^2 + x3^2*z1^2*z3^2 + 2*x4^2*z1^2*z2^2 + 2*y1^2*y2^2*z4^2 + y1^2*y3^2*z3^2 + 2*y1^2*y4^2*z2^2 + y2^2*y3^2*z2^2 + 2*y2^2*y4^2*z1^2 + 2*x1^2*z3^2*z4^2 + x2^2*z2^2*z4^2 + 2*x3^2*z1^2*z4^2 + x3^2*z2^2*z3^2 + 2*x4^2*z1^2*z3^2 + 2*y1^2*y3^2*z4^2 + 2*y1^2*y4^2*z3^2 + y2^2*y3^2*z3^2 + y2^2*y4^2*z2^2 + 2*y3^2*y4^2*z1^2 + 2*x2^2*z3^2*z4^2 + 2*x3^2*z2^2*z4^2 + x4^2*z1^2*z4^2 + 2*x4^2*z2^2*z3^2 + y1^2*y4^2*z4^2 + 2*y2^2*y3^2*z4^2 + 2*y2^2*y4^2*z3^2 + 2*y3^2*y4^2*z2^2 + x3^2*z3^2*z4^2 + x4^2*z2^2*z4^2 + y2^2*y4^2*z4^2 + y3^2*y4^2*z3^2 + x4^2*z3^2*z4^2 + y3^2*y4^2*z4^2 + y1^2*z1^2*z2^2 + y1^2*z1^2*z3^2 + y2^2*z1^2*z2^2 + y1^2*z1^2*z4^2 + 2*y1^2*z2^2*z3^2 + 2*y2^2*z1^2*z3^2 + 2*y3^2*z1^2*z2^2 + 2*y1^2*z2^2*z4^2 + 2*y2^2*z1^2*z4^2 + y2^2*z2^2*z3^2 + y3^2*z1^2*z3^2 + 2*y4^2*z1^2*z2^2 + 2*y1^2*z3^2*z4^2 + y2^2*z2^2*z4^2 + 2*y3^2*z1^2*z4^2 + y3^2*z2^2*z3^2 + 2*y4^2*z1^2*z3^2 + 2*y2^2*z3^2*z4^2 + 2*y3^2*z2^2*z4^2 + y4^2*z1^2*z4^2 + 2*y4^2*z2^2*z3^2 + y3^2*z3^2*z4^2 + y4^2*z2^2*z4^2 + y4^2*z3^2*z4^2 - 8*x1*x2*y1*y2 - 8*x1*x3*y1*y3 - 8*x1*x4*y1*y4 - 8*x2*x3*y2*y3 - 8*x2*x4*y2*y4 - 8*x3*x4*y3*y4 - 8*x1*x2*z1*z2 - 8*x1*x3*z1*z3 - 8*x1*x4*z1*z4 - 8*x2*x3*z2*z3 - 8*x2*x4*z2*z4 - 8*x3*x4*z3*z4 - 8*y1*y2*z1*z2 - 8*y1*y3*z1*z3 - 8*y1*y4*z1*z4 - 8*y2*y3*z2*z3 - 8*y2*y4*z2*z4 - 8*y3*y4*z3*z4 - 2*x1*x2*y1*y2^3 - 2*x1*x2*y1^3*y2 - 2*x1*x2^3*y1*y2 - 2*x1^3*x2*y1*y2 - 2*x1*x3*y1*y3^3 - 2*x1*x3*y1^3*y3 - 2*x1*x3^3*y1*y3 - 2*x1^3*x3*y1*y3 - 2*x1*x4*y1*y4^3 - 2*x1*x4*y1^3*y4 - 2*x1*x4^3*y1*y4 - 2*x2*x3*y2*y3^3 - 2*x2*x3*y2^3*y3 - 2*x2*x3^3*y2*y3 - 2*x1^3*x4*y1*y4 - 2*x2^3*x3*y2*y3 - 2*x2*x4*y2*y4^3 - 2*x2*x4*y2^3*y4 - 2*x2*x4^3*y2*y4 - 2*x2^3*x4*y2*y4 - 2*x3*x4*y3*y4^3 - 2*x3*x4*y3^3*y4 - 2*x3*x4^3*y3*y4 - 2*x3^3*x4*y3*y4 - 2*x1*x2*z1*z2^3 - 2*x1*x2*z1^3*z2 - 2*x1*x2^3*z1*z2 - 2*x1^3*x2*z1*z2 - 2*x1*x3*z1*z3^3 - 2*x1*x3*z1^3*z3 - 2*x1*x3^3*z1*z3 - 2*x1^3*x3*z1*z3 - 2*x1*x4*z1*z4^3 - 2*x1*x4*z1^3*z4 - 2*x1*x4^3*z1*z4 - 2*x2*x3*z2*z3^3 - 2*x2*x3*z2^3*z3 - 2*x2*x3^3*z2*z3 - 2*x1^3*x4*z1*z4 - 2*x2^3*x3*z2*z3 - 2*x2*x4*z2*z4^3 - 2*x2*x4*z2^3*z4 - 2*x2*x4^3*z2*z4 - 2*x2^3*x4*z2*z4 - 2*x3*x4*z3*z4^3 - 2*x3*x4*z3^3*z4 - 2*x3*x4^3*z3*z4 - 2*x3^3*x4*z3*z4 - 2*y1*y2*z1*z2^3 - 2*y1*y2*z1^3*z2 - 2*y1*y2^3*z1*z2 - 2*y1^3*y2*z1*z2 - 2*y1*y3*z1*z3^3 - 2*y1*y3*z1^3*z3 - 2*y1*y3^3*z1*z3 - 2*y1^3*y3*z1*z3 - 2*y1*y4*z1*z4^3 - 2*y1*y4*z1^3*z4 - 2*y1*y4^3*z1*z4 - 2*y2*y3*z2*z3^3 - 2*y2*y3*z2^3*z3 - 2*y2*y3^3*z2*z3 - 2*y1^3*y4*z1*z4 - 2*y2^3*y3*z2*z3 - 2*y2*y4*z2*z4^3 - 2*y2*y4*z2^3*z4 - 2*y2*y4^3*z2*z4 - 2*y2^3*y4*z2*z4 - 2*y3*y4*z3*z4^3 - 2*y3*y4*z3^3*z4 - 2*y3*y4^3*z3*z4 - 2*y3^3*y4*z3*z4 - 2*x1*x2*x3^2*y1*y2 - 2*x1*x2*x4^2*y1*y2 - 2*x1*x2^2*x3*y1*y3 - 2*x1^2*x2*x3*y2*y3 - 2*x1*x3*x4^2*y1*y3 - 2*x1*x2^2*x4*y1*y4 - 2*x1*x3^2*x4*y1*y4 - 2*x1^2*x2*x4*y2*y4 - 2*x2*x3*x4^2*y2*y3 - 2*x2*x3^2*x4*y2*y4 - 2*x1^2*x3*x4*y3*y4 - 2*x2^2*x3*x4*y3*y4 - 2*x1*x2*y1*y2*y3^2 - 2*x1*x2*y1*y2*y4^2 - 2*x1*x3*y1*y2^2*y3 - 2*x2*x3*y1^2*y2*y3 - 2*x1*x3*y1*y3*y4^2 - 2*x1*x4*y1*y2^2*y4 - 2*x1*x4*y1*y3^2*y4 - 2*x2*x4*y1^2*y2*y4 - 2*x2*x3*y2*y3*y4^2 - 2*x2*x4*y2*y3^2*y4 - 2*x3*x4*y1^2*y3*y4 - 2*x3*x4*y2^2*y3*y4 - 2*x1*x2*y1*y2*z1^2 - 2*x1*x2*y1*y2*z2^2 - 2*x1*x2*x3^2*z1*z2 - 2*x1*x3*y1*y3*z1^2 - 2*x1*x2*x4^2*z1*z2 - 2*x1*x2^2*x3*z1*z3 - 2*x1*x3*y1*y3*z3^2 - 2*x1*x4*y1*y4*z1^2 - 2*x1^2*x2*x3*z2*z3 - 2*x1*x3*x4^2*z1*z3 - 2*x1*x2^2*x4*z1*z4 - 2*x2*x3*y2*y3*z2^2 - 2*x1*x3^2*x4*z1*z4 - 2*x2*x3*y2*y3*z3^2 - 2*x1^2*x2*x4*z2*z4 - 2*x1*x4*y1*y4*z4^2 - 2*x2*x3*x4^2*z2*z3 - 2*x2*x4*y2*y4*z2^2 - 2*x2*x3^2*x4*z2*z4 - 2*x1^2*x3*x4*z3*z4 - 2*x2*x4*y2*y4*z4^2 - 2*x2^2*x3*x4*z3*z4 - 2*x3*x4*y3*y4*z3^2 - 2*x3*x4*y3*y4*z4^2 - 2*x1*x2*y1^2*z1*z2 - 2*x1*x2*y2^2*z1*z2 - 2*x1*x3*y1^2*z1*z3 - 2*x1*x3*y3^2*z1*z3 - 2*x1*x4*y1^2*z1*z4 - 2*x2*x3*y2^2*z2*z3 - 2*x2*x3*y3^2*z2*z3 - 2*x1*x4*y4^2*z1*z4 - 2*x2*x4*y2^2*z2*z4 - 2*x2*x4*y4^2*z2*z4 - 2*x3*x4*y3^2*z3*z4 - 2*x3*x4*y4^2*z3*z4 - 2*x1^2*y1*y2*z1*z2 - 2*x2^2*y1*y2*z1*z2 - 2*x1*x2*z1*z2*z3^2 - 2*x1^2*y1*y3*z1*z3 - 2*x1*x2*z1*z2*z4^2 - 2*x1*x3*z1*z2^2*z3 - 2*x2*x3*z1^2*z2*z3 - 2*x1^2*y1*y4*z1*z4 - 2*x3^2*y1*y3*z1*z3 - 2*x1*x3*z1*z3*z4^2 - 2*x1*x4*z1*z2^2*z4 - 2*x2^2*y2*y3*z2*z3 - 2*x1*x4*z1*z3^2*z4 - 2*x2*x4*z1^2*z2*z4 - 2*x3^2*y2*y3*z2*z3 - 2*x2*x3*z2*z3*z4^2 - 2*x2^2*y2*y4*z2*z4 - 2*x4^2*y1*y4*z1*z4 - 2*x2*x4*z2*z3^2*z4 - 2*x3*x4*z1^2*z3*z4 - 2*x3*x4*z2^2*z3*z4 - 2*x4^2*y2*y4*z2*z4 - 2*x3^2*y3*y4*z3*z4 - 2*x4^2*y3*y4*z3*z4 - 2*y1*y2*y3^2*z1*z2 - 2*y1*y2*y4^2*z1*z2 - 2*y1*y2^2*y3*z1*z3 - 2*y1^2*y2*y3*z2*z3 - 2*y1*y3*y4^2*z1*z3 - 2*y1*y2^2*y4*z1*z4 - 2*y1*y3^2*y4*z1*z4 - 2*y1^2*y2*y4*z2*z4 - 2*y2*y3*y4^2*z2*z3 - 2*y2*y3^2*y4*z2*z4 - 2*y1^2*y3*y4*z3*z4 - 2*y2^2*y3*y4*z3*z4 - 2*y1*y2*z1*z2*z3^2 - 2*y1*y2*z1*z2*z4^2 - 2*y1*y3*z1*z2^2*z3 - 2*y2*y3*z1^2*z2*z3 - 2*y1*y3*z1*z3*z4^2 - 2*y1*y4*z1*z2^2*z4 - 2*y1*y4*z1*z3^2*z4 - 2*y2*y4*z1^2*z2*z4 - 2*y2*y3*z2*z3*z4^2 - 2*y2*y4*z2*z3^2*z4 - 2*y3*y4*z1^2*z3*z4 - 2*y3*y4*z2^2*z3*z4 - 2*x1*x2*y1*y3*z2*z3 - 2*x1*x2*y2*y3*z1*z3 - 2*x1*x3*y1*y2*z2*z3 - 2*x1*x3*y2*y3*z1*z2 - 2*x2*x3*y1*y2*z1*z3 - 2*x2*x3*y1*y3*z1*z2 - 2*x1*x2*y1*y4*z2*z4 - 2*x1*x2*y2*y4*z1*z4 - 2*x1*x4*y1*y2*z2*z4 - 2*x1*x4*y2*y4*z1*z2 - 2*x2*x4*y1*y2*z1*z4 - 2*x2*x4*y1*y4*z1*z2 - 2*x1*x3*y1*y4*z3*z4 - 2*x1*x3*y3*y4*z1*z4 - 2*x1*x4*y1*y3*z3*z4 - 2*x1*x4*y3*y4*z1*z3 - 2*x3*x4*y1*y3*z1*z4 - 2*x3*x4*y1*y4*z1*z3 - 2*x2*x3*y2*y4*z3*z4 - 2*x2*x3*y3*y4*z2*z4 - 2*x2*x4*y2*y3*z3*z4 - 2*x2*x4*y3*y4*z2*z3 - 2*x3*x4*y2*y3*z2*z4 - 2*x3*x4*y2*y4*z2*z3 + 64);
        (4*(4*x1*y1 + 4*x2*y2 + 4*x3*y3 + 4*x4*y4 + x1*y1^3 + x1^3*y1 + x2*y2^3 + x2^3*y2 + x3*y3^3 + x3^3*y3 + x4*y4^3 + x4^3*y4 + x1*x2^2*y1 + x1*x3^2*y1 + x1^2*x2*y2 + x1*x4^2*y1 + x2*x3^2*y2 + x1^2*x3*y3 + x2*x4^2*y2 + x2^2*x3*y3 + x1^2*x4*y4 + x3*x4^2*y3 + x2^2*x4*y4 + x3^2*x4*y4 + x1*y1*y2^2 + x1*y1*y3^2 + x2*y1^2*y2 + x1*y1*y4^2 + x2*y2*y3^2 + x3*y1^2*y3 + x2*y2*y4^2 + x3*y2^2*y3 + x4*y1^2*y4 + x3*y3*y4^2 + x4*y2^2*y4 + x4*y3^2*y4 + x1*y1*z1^2 + x2*y2*z2^2 + x3*y3*z3^2 + x4*y4*z4^2 + x1*y2*z1*z2 + x2*y1*z1*z2 + x1*y3*z1*z3 + x3*y1*z1*z3 + x1*y4*z1*z4 + x2*y3*z2*z3 + x3*y2*z2*z3 + x4*y1*z1*z4 + x2*y4*z2*z4 + x4*y2*z2*z4 + x3*y4*z3*z4 + x4*y3*z3*z4))/(8*x1^2*x2^2 + 8*x1^2*x3^2 + 8*x1^2*x4^2 + 8*x2^2*x3^2 + 8*x2^2*x4^2 + 8*x3^2*x4^2 + 8*x1^2*y1^2 + 12*x1^2*y2^2 + 12*x2^2*y1^2 + 12*x1^2*y3^2 + 8*x2^2*y2^2 + 12*x3^2*y1^2 + x1^2*y2^4 + 12*x1^2*y4^2 + x2^2*y1^4 + 12*x2^2*y3^2 + x1^4*y2^2 + 12*x3^2*y2^2 + x2^4*y1^2 + 12*x4^2*y1^2 + x1^2*y3^4 + 12*x2^2*y4^2 + x1^4*y3^2 + x3^2*y1^4 + 8*x3^2*y3^2 + 12*x4^2*y2^2 + x3^4*y1^2 + x1^2*y4^4 + x2^2*y3^4 + x1^4*y4^2 + x3^2*y2^4 + 12*x3^2*y4^2 + x2^4*y3^2 + x4^2*y1^4 + 12*x4^2*y3^2 + x3^4*y2^2 + x4^4*y1^2 + x2^2*y4^4 + x2^4*y4^2 + x4^2*y2^4 + 8*x4^2*y4^2 + x4^4*y2^2 + x3^2*y4^4 + x4^2*y3^4 + x3^4*y4^2 + x4^4*y3^2 + 8*x1^2*z1^2 + 12*x1^2*z2^2 + 12*x2^2*z1^2 + 8*y1^2*y2^2 + 12*x1^2*z3^2 + 8*x2^2*z2^2 + 12*x3^2*z1^2 + 8*y1^2*y3^2 + x1^2*z2^4 + 12*x1^2*z4^2 + x2^2*z1^4 + 12*x2^2*z3^2 + x1^4*z2^2 + 12*x3^2*z2^2 + x2^4*z1^2 + 12*x4^2*z1^2 + 8*y1^2*y4^2 + 8*y2^2*y3^2 + x1^2*z3^4 + 12*x2^2*z4^2 + x1^4*z3^2 + x3^2*z1^4 + 8*x3^2*z3^2 + 12*x4^2*z2^2 + x3^4*z1^2 + 8*y2^2*y4^2 + x1^2*z4^4 + x2^2*z3^4 + x1^4*z4^2 + x3^2*z2^4 + 12*x3^2*z4^2 + x2^4*z3^2 + x4^2*z1^4 + 12*x4^2*z3^2 + x3^4*z2^2 + x4^4*z1^2 + 8*y3^2*y4^2 + x2^2*z4^4 + x2^4*z4^2 + x4^2*z2^4 + 8*x4^2*z4^2 + x4^4*z2^2 + x3^2*z4^4 + x4^2*z3^4 + x3^4*z4^2 + x4^4*z3^2 + 8*y1^2*z1^2 + 12*y1^2*z2^2 + 12*y2^2*z1^2 + 12*y1^2*z3^2 + 8*y2^2*z2^2 + 12*y3^2*z1^2 + y1^2*z2^4 + 12*y1^2*z4^2 + y2^2*z1^4 + 12*y2^2*z3^2 + y1^4*z2^2 + 12*y3^2*z2^2 + y2^4*z1^2 + 12*y4^2*z1^2 + y1^2*z3^4 + 12*y2^2*z4^2 + y1^4*z3^2 + y3^2*z1^4 + 8*y3^2*z3^2 + 12*y4^2*z2^2 + y3^4*z1^2 + y1^2*z4^4 + y2^2*z3^4 + y1^4*z4^2 + y3^2*z2^4 + 12*y3^2*z4^2 + y2^4*z3^2 + y4^2*z1^4 + 12*y4^2*z3^2 + y3^4*z2^2 + y4^4*z1^2 + y2^2*z4^4 + y2^4*z4^2 + y4^2*z2^4 + 8*y4^2*z4^2 + y4^4*z2^2 + y3^2*z4^4 + y4^2*z3^4 + y3^4*z4^2 + y4^4*z3^2 + 8*z1^2*z2^2 + 8*z1^2*z3^2 + 8*z1^2*z4^2 + 8*z2^2*z3^2 + 8*z2^2*z4^2 + 8*z3^2*z4^2 + 32*x1^2 + 32*x2^2 + 4*x1^4 + 32*x3^2 + 4*x2^4 + 32*x4^2 + 4*x3^4 + 4*x4^4 + 32*y1^2 + 32*y2^2 + 4*y1^4 + 32*y3^2 + 4*y2^4 + 32*y4^2 + 4*y3^4 + 4*y4^4 + 32*z1^2 + 32*z2^2 + 4*z1^4 + 32*z3^2 + 4*z2^4 + 32*z4^2 + 4*z3^4 + 4*z4^4 + x1^2*x2^2*y1^2 + x1^2*x2^2*y2^2 + x1^2*x3^2*y1^2 + 2*x1^2*x2^2*y3^2 + 2*x1^2*x3^2*y2^2 + x1^2*x4^2*y1^2 + 2*x2^2*x3^2*y1^2 + 2*x1^2*x2^2*y4^2 + x1^2*x3^2*y3^2 + 2*x1^2*x4^2*y2^2 + x2^2*x3^2*y2^2 + 2*x2^2*x4^2*y1^2 + 2*x1^2*x3^2*y4^2 + 2*x1^2*x4^2*y3^2 + x2^2*x3^2*y3^2 + x2^2*x4^2*y2^2 + 2*x3^2*x4^2*y1^2 + x1^2*x4^2*y4^2 + 2*x2^2*x3^2*y4^2 + 2*x2^2*x4^2*y3^2 + 2*x3^2*x4^2*y2^2 + x2^2*x4^2*y4^2 + x3^2*x4^2*y3^2 + x3^2*x4^2*y4^2 + x1^2*x2^2*z1^2 + x1^2*y1^2*y2^2 + x1^2*x2^2*z2^2 + x1^2*x3^2*z1^2 + x1^2*y1^2*y3^2 + x2^2*y1^2*y2^2 + 2*x1^2*x2^2*z3^2 + 2*x1^2*x3^2*z2^2 + x1^2*x4^2*z1^2 + x1^2*y1^2*y4^2 + 2*x1^2*y2^2*y3^2 + 2*x2^2*x3^2*z1^2 + 2*x2^2*y1^2*y3^2 + 2*x3^2*y1^2*y2^2 + 2*x1^2*x2^2*z4^2 + x1^2*x3^2*z3^2 + 2*x1^2*x4^2*z2^2 + 2*x1^2*y2^2*y4^2 + x2^2*x3^2*z2^2 + 2*x2^2*x4^2*z1^2 + 2*x2^2*y1^2*y4^2 + x2^2*y2^2*y3^2 + x3^2*y1^2*y3^2 + 2*x4^2*y1^2*y2^2 + 2*x1^2*x3^2*z4^2 + 2*x1^2*x4^2*z3^2 + 2*x1^2*y3^2*y4^2 + x2^2*x3^2*z3^2 + x2^2*x4^2*z2^2 + x2^2*y2^2*y4^2 + 2*x3^2*x4^2*z1^2 + 2*x3^2*y1^2*y4^2 + x3^2*y2^2*y3^2 + 2*x4^2*y1^2*y3^2 + x1^2*x4^2*z4^2 + 2*x2^2*x3^2*z4^2 + 2*x2^2*x4^2*z3^2 + 2*x2^2*y3^2*y4^2 + 2*x3^2*x4^2*z2^2 + 2*x3^2*y2^2*y4^2 + x4^2*y1^2*y4^2 + 2*x4^2*y2^2*y3^2 + x2^2*x4^2*z4^2 + x3^2*x4^2*z3^2 + x3^2*y3^2*y4^2 + x4^2*y2^2*y4^2 + x3^2*x4^2*z4^2 + x4^2*y3^2*y4^2 + 2*x1^2*y1^2*z2^2 + 2*x1^2*y2^2*z1^2 + 2*x2^2*y1^2*z1^2 + 2*x1^2*y1^2*z3^2 + 2*x1^2*y2^2*z2^2 + 2*x1^2*y3^2*z1^2 + 2*x2^2*y1^2*z2^2 + 2*x2^2*y2^2*z1^2 + 2*x3^2*y1^2*z1^2 + 2*x1^2*y1^2*z4^2 + 2*x1^2*y2^2*z3^2 + 2*x1^2*y3^2*z2^2 + 2*x1^2*y4^2*z1^2 + 2*x2^2*y1^2*z3^2 + 2*x2^2*y3^2*z1^2 + 2*x3^2*y1^2*z2^2 + 2*x3^2*y2^2*z1^2 + 2*x4^2*y1^2*z1^2 + 2*x1^2*y2^2*z4^2 + 2*x1^2*y3^2*z3^2 + 2*x1^2*y4^2*z2^2 + 2*x2^2*y1^2*z4^2 + 2*x2^2*y2^2*z3^2 + 2*x2^2*y3^2*z2^2 + 2*x2^2*y4^2*z1^2 + 2*x3^2*y1^2*z3^2 + 2*x3^2*y2^2*z2^2 + 2*x3^2*y3^2*z1^2 + 2*x4^2*y1^2*z2^2 + 2*x4^2*y2^2*z1^2 + 2*x1^2*y3^2*z4^2 + 2*x1^2*y4^2*z3^2 + 2*x2^2*y2^2*z4^2 + 2*x2^2*y3^2*z3^2 + 2*x2^2*y4^2*z2^2 + 2*x3^2*y1^2*z4^2 + 2*x3^2*y2^2*z3^2 + 2*x3^2*y3^2*z2^2 + 2*x3^2*y4^2*z1^2 + 2*x4^2*y1^2*z3^2 + 2*x4^2*y2^2*z2^2 + 2*x4^2*y3^2*z1^2 + 2*x1^2*y4^2*z4^2 + 2*x2^2*y3^2*z4^2 + 2*x2^2*y4^2*z3^2 + 2*x3^2*y2^2*z4^2 + 2*x3^2*y4^2*z2^2 + 2*x4^2*y1^2*z4^2 + 2*x4^2*y2^2*z3^2 + 2*x4^2*y3^2*z2^2 + 2*x4^2*y4^2*z1^2 + 2*x2^2*y4^2*z4^2 + 2*x3^2*y3^2*z4^2 + 2*x3^2*y4^2*z3^2 + 2*x4^2*y2^2*z4^2 + 2*x4^2*y3^2*z3^2 + 2*x4^2*y4^2*z2^2 + 2*x3^2*y4^2*z4^2 + 2*x4^2*y3^2*z4^2 + 2*x4^2*y4^2*z3^2 + x1^2*z1^2*z2^2 + y1^2*y2^2*z1^2 + x1^2*z1^2*z3^2 + x2^2*z1^2*z2^2 + y1^2*y2^2*z2^2 + y1^2*y3^2*z1^2 + x1^2*z1^2*z4^2 + 2*x1^2*z2^2*z3^2 + 2*x2^2*z1^2*z3^2 + 2*x3^2*z1^2*z2^2 + 2*y1^2*y2^2*z3^2 + 2*y1^2*y3^2*z2^2 + y1^2*y4^2*z1^2 + 2*y2^2*y3^2*z1^2 + 2*x1^2*z2^2*z4^2 + 2*x2^2*z1^2*z4^2 + x2^2*z2^2*z3^2 + x3^2*z1^2*z3^2 + 2*x4^2*z1^2*z2^2 + 2*y1^2*y2^2*z4^2 + y1^2*y3^2*z3^2 + 2*y1^2*y4^2*z2^2 + y2^2*y3^2*z2^2 + 2*y2^2*y4^2*z1^2 + 2*x1^2*z3^2*z4^2 + x2^2*z2^2*z4^2 + 2*x3^2*z1^2*z4^2 + x3^2*z2^2*z3^2 + 2*x4^2*z1^2*z3^2 + 2*y1^2*y3^2*z4^2 + 2*y1^2*y4^2*z3^2 + y2^2*y3^2*z3^2 + y2^2*y4^2*z2^2 + 2*y3^2*y4^2*z1^2 + 2*x2^2*z3^2*z4^2 + 2*x3^2*z2^2*z4^2 + x4^2*z1^2*z4^2 + 2*x4^2*z2^2*z3^2 + y1^2*y4^2*z4^2 + 2*y2^2*y3^2*z4^2 + 2*y2^2*y4^2*z3^2 + 2*y3^2*y4^2*z2^2 + x3^2*z3^2*z4^2 + x4^2*z2^2*z4^2 + y2^2*y4^2*z4^2 + y3^2*y4^2*z3^2 + x4^2*z3^2*z4^2 + y3^2*y4^2*z4^2 + y1^2*z1^2*z2^2 + y1^2*z1^2*z3^2 + y2^2*z1^2*z2^2 + y1^2*z1^2*z4^2 + 2*y1^2*z2^2*z3^2 + 2*y2^2*z1^2*z3^2 + 2*y3^2*z1^2*z2^2 + 2*y1^2*z2^2*z4^2 + 2*y2^2*z1^2*z4^2 + y2^2*z2^2*z3^2 + y3^2*z1^2*z3^2 + 2*y4^2*z1^2*z2^2 + 2*y1^2*z3^2*z4^2 + y2^2*z2^2*z4^2 + 2*y3^2*z1^2*z4^2 + y3^2*z2^2*z3^2 + 2*y4^2*z1^2*z3^2 + 2*y2^2*z3^2*z4^2 + 2*y3^2*z2^2*z4^2 + y4^2*z1^2*z4^2 + 2*y4^2*z2^2*z3^2 + y3^2*z3^2*z4^2 + y4^2*z2^2*z4^2 + y4^2*z3^2*z4^2 - 8*x1*x2*y1*y2 - 8*x1*x3*y1*y3 - 8*x1*x4*y1*y4 - 8*x2*x3*y2*y3 - 8*x2*x4*y2*y4 - 8*x3*x4*y3*y4 - 8*x1*x2*z1*z2 - 8*x1*x3*z1*z3 - 8*x1*x4*z1*z4 - 8*x2*x3*z2*z3 - 8*x2*x4*z2*z4 - 8*x3*x4*z3*z4 - 8*y1*y2*z1*z2 - 8*y1*y3*z1*z3 - 8*y1*y4*z1*z4 - 8*y2*y3*z2*z3 - 8*y2*y4*z2*z4 - 8*y3*y4*z3*z4 - 2*x1*x2*y1*y2^3 - 2*x1*x2*y1^3*y2 - 2*x1*x2^3*y1*y2 - 2*x1^3*x2*y1*y2 - 2*x1*x3*y1*y3^3 - 2*x1*x3*y1^3*y3 - 2*x1*x3^3*y1*y3 - 2*x1^3*x3*y1*y3 - 2*x1*x4*y1*y4^3 - 2*x1*x4*y1^3*y4 - 2*x1*x4^3*y1*y4 - 2*x2*x3*y2*y3^3 - 2*x2*x3*y2^3*y3 - 2*x2*x3^3*y2*y3 - 2*x1^3*x4*y1*y4 - 2*x2^3*x3*y2*y3 - 2*x2*x4*y2*y4^3 - 2*x2*x4*y2^3*y4 - 2*x2*x4^3*y2*y4 - 2*x2^3*x4*y2*y4 - 2*x3*x4*y3*y4^3 - 2*x3*x4*y3^3*y4 - 2*x3*x4^3*y3*y4 - 2*x3^3*x4*y3*y4 - 2*x1*x2*z1*z2^3 - 2*x1*x2*z1^3*z2 - 2*x1*x2^3*z1*z2 - 2*x1^3*x2*z1*z2 - 2*x1*x3*z1*z3^3 - 2*x1*x3*z1^3*z3 - 2*x1*x3^3*z1*z3 - 2*x1^3*x3*z1*z3 - 2*x1*x4*z1*z4^3 - 2*x1*x4*z1^3*z4 - 2*x1*x4^3*z1*z4 - 2*x2*x3*z2*z3^3 - 2*x2*x3*z2^3*z3 - 2*x2*x3^3*z2*z3 - 2*x1^3*x4*z1*z4 - 2*x2^3*x3*z2*z3 - 2*x2*x4*z2*z4^3 - 2*x2*x4*z2^3*z4 - 2*x2*x4^3*z2*z4 - 2*x2^3*x4*z2*z4 - 2*x3*x4*z3*z4^3 - 2*x3*x4*z3^3*z4 - 2*x3*x4^3*z3*z4 - 2*x3^3*x4*z3*z4 - 2*y1*y2*z1*z2^3 - 2*y1*y2*z1^3*z2 - 2*y1*y2^3*z1*z2 - 2*y1^3*y2*z1*z2 - 2*y1*y3*z1*z3^3 - 2*y1*y3*z1^3*z3 - 2*y1*y3^3*z1*z3 - 2*y1^3*y3*z1*z3 - 2*y1*y4*z1*z4^3 - 2*y1*y4*z1^3*z4 - 2*y1*y4^3*z1*z4 - 2*y2*y3*z2*z3^3 - 2*y2*y3*z2^3*z3 - 2*y2*y3^3*z2*z3 - 2*y1^3*y4*z1*z4 - 2*y2^3*y3*z2*z3 - 2*y2*y4*z2*z4^3 - 2*y2*y4*z2^3*z4 - 2*y2*y4^3*z2*z4 - 2*y2^3*y4*z2*z4 - 2*y3*y4*z3*z4^3 - 2*y3*y4*z3^3*z4 - 2*y3*y4^3*z3*z4 - 2*y3^3*y4*z3*z4 - 2*x1*x2*x3^2*y1*y2 - 2*x1*x2*x4^2*y1*y2 - 2*x1*x2^2*x3*y1*y3 - 2*x1^2*x2*x3*y2*y3 - 2*x1*x3*x4^2*y1*y3 - 2*x1*x2^2*x4*y1*y4 - 2*x1*x3^2*x4*y1*y4 - 2*x1^2*x2*x4*y2*y4 - 2*x2*x3*x4^2*y2*y3 - 2*x2*x3^2*x4*y2*y4 - 2*x1^2*x3*x4*y3*y4 - 2*x2^2*x3*x4*y3*y4 - 2*x1*x2*y1*y2*y3^2 - 2*x1*x2*y1*y2*y4^2 - 2*x1*x3*y1*y2^2*y3 - 2*x2*x3*y1^2*y2*y3 - 2*x1*x3*y1*y3*y4^2 - 2*x1*x4*y1*y2^2*y4 - 2*x1*x4*y1*y3^2*y4 - 2*x2*x4*y1^2*y2*y4 - 2*x2*x3*y2*y3*y4^2 - 2*x2*x4*y2*y3^2*y4 - 2*x3*x4*y1^2*y3*y4 - 2*x3*x4*y2^2*y3*y4 - 2*x1*x2*y1*y2*z1^2 - 2*x1*x2*y1*y2*z2^2 - 2*x1*x2*x3^2*z1*z2 - 2*x1*x3*y1*y3*z1^2 - 2*x1*x2*x4^2*z1*z2 - 2*x1*x2^2*x3*z1*z3 - 2*x1*x3*y1*y3*z3^2 - 2*x1*x4*y1*y4*z1^2 - 2*x1^2*x2*x3*z2*z3 - 2*x1*x3*x4^2*z1*z3 - 2*x1*x2^2*x4*z1*z4 - 2*x2*x3*y2*y3*z2^2 - 2*x1*x3^2*x4*z1*z4 - 2*x2*x3*y2*y3*z3^2 - 2*x1^2*x2*x4*z2*z4 - 2*x1*x4*y1*y4*z4^2 - 2*x2*x3*x4^2*z2*z3 - 2*x2*x4*y2*y4*z2^2 - 2*x2*x3^2*x4*z2*z4 - 2*x1^2*x3*x4*z3*z4 - 2*x2*x4*y2*y4*z4^2 - 2*x2^2*x3*x4*z3*z4 - 2*x3*x4*y3*y4*z3^2 - 2*x3*x4*y3*y4*z4^2 - 2*x1*x2*y1^2*z1*z2 - 2*x1*x2*y2^2*z1*z2 - 2*x1*x3*y1^2*z1*z3 - 2*x1*x3*y3^2*z1*z3 - 2*x1*x4*y1^2*z1*z4 - 2*x2*x3*y2^2*z2*z3 - 2*x2*x3*y3^2*z2*z3 - 2*x1*x4*y4^2*z1*z4 - 2*x2*x4*y2^2*z2*z4 - 2*x2*x4*y4^2*z2*z4 - 2*x3*x4*y3^2*z3*z4 - 2*x3*x4*y4^2*z3*z4 - 2*x1^2*y1*y2*z1*z2 - 2*x2^2*y1*y2*z1*z2 - 2*x1*x2*z1*z2*z3^2 - 2*x1^2*y1*y3*z1*z3 - 2*x1*x2*z1*z2*z4^2 - 2*x1*x3*z1*z2^2*z3 - 2*x2*x3*z1^2*z2*z3 - 2*x1^2*y1*y4*z1*z4 - 2*x3^2*y1*y3*z1*z3 - 2*x1*x3*z1*z3*z4^2 - 2*x1*x4*z1*z2^2*z4 - 2*x2^2*y2*y3*z2*z3 - 2*x1*x4*z1*z3^2*z4 - 2*x2*x4*z1^2*z2*z4 - 2*x3^2*y2*y3*z2*z3 - 2*x2*x3*z2*z3*z4^2 - 2*x2^2*y2*y4*z2*z4 - 2*x4^2*y1*y4*z1*z4 - 2*x2*x4*z2*z3^2*z4 - 2*x3*x4*z1^2*z3*z4 - 2*x3*x4*z2^2*z3*z4 - 2*x4^2*y2*y4*z2*z4 - 2*x3^2*y3*y4*z3*z4 - 2*x4^2*y3*y4*z3*z4 - 2*y1*y2*y3^2*z1*z2 - 2*y1*y2*y4^2*z1*z2 - 2*y1*y2^2*y3*z1*z3 - 2*y1^2*y2*y3*z2*z3 - 2*y1*y3*y4^2*z1*z3 - 2*y1*y2^2*y4*z1*z4 - 2*y1*y3^2*y4*z1*z4 - 2*y1^2*y2*y4*z2*z4 - 2*y2*y3*y4^2*z2*z3 - 2*y2*y3^2*y4*z2*z4 - 2*y1^2*y3*y4*z3*z4 - 2*y2^2*y3*y4*z3*z4 - 2*y1*y2*z1*z2*z3^2 - 2*y1*y2*z1*z2*z4^2 - 2*y1*y3*z1*z2^2*z3 - 2*y2*y3*z1^2*z2*z3 - 2*y1*y3*z1*z3*z4^2 - 2*y1*y4*z1*z2^2*z4 - 2*y1*y4*z1*z3^2*z4 - 2*y2*y4*z1^2*z2*z4 - 2*y2*y3*z2*z3*z4^2 - 2*y2*y4*z2*z3^2*z4 - 2*y3*y4*z1^2*z3*z4 - 2*y3*y4*z2^2*z3*z4 - 2*x1*x2*y1*y3*z2*z3 - 2*x1*x2*y2*y3*z1*z3 - 2*x1*x3*y1*y2*z2*z3 - 2*x1*x3*y2*y3*z1*z2 - 2*x2*x3*y1*y2*z1*z3 - 2*x2*x3*y1*y3*z1*z2 - 2*x1*x2*y1*y4*z2*z4 - 2*x1*x2*y2*y4*z1*z4 - 2*x1*x4*y1*y2*z2*z4 - 2*x1*x4*y2*y4*z1*z2 - 2*x2*x4*y1*y2*z1*z4 - 2*x2*x4*y1*y4*z1*z2 - 2*x1*x3*y1*y4*z3*z4 - 2*x1*x3*y3*y4*z1*z4 - 2*x1*x4*y1*y3*z3*z4 - 2*x1*x4*y3*y4*z1*z3 - 2*x3*x4*y1*y3*z1*z4 - 2*x3*x4*y1*y4*z1*z3 - 2*x2*x3*y2*y4*z3*z4 - 2*x2*x3*y3*y4*z2*z4 - 2*x2*x4*y2*y3*z3*z4 - 2*x2*x4*y3*y4*z2*z3 - 2*x3*x4*y2*y3*z2*z4 - 2*x3*x4*y2*y4*z2*z3 + 64),...
        (4*(x1^2*y1^2 + x1^2*y2^2 + x2^2*y1^2 + x1^2*y3^2 + x2^2*y2^2 + x3^2*y1^2 + x1^2*y4^2 + x2^2*y3^2 + x3^2*y2^2 + x4^2*y1^2 + x2^2*y4^2 + x3^2*y3^2 + x4^2*y2^2 + x3^2*y4^2 + x4^2*y3^2 + x4^2*y4^2 + x1^2*z2^2 + x2^2*z1^2 + 2*y1^2*y2^2 + x1^2*z3^2 + x3^2*z1^2 + 2*y1^2*y3^2 + x1^2*z4^2 + x2^2*z3^2 + x3^2*z2^2 + x4^2*z1^2 + 2*y1^2*y4^2 + 2*y2^2*y3^2 + x2^2*z4^2 + x4^2*z2^2 + 2*y2^2*y4^2 + x3^2*z4^2 + x4^2*z3^2 + 2*y3^2*y4^2 + y1^2*z1^2 + y1^2*z2^2 + y2^2*z1^2 + y1^2*z3^2 + y2^2*z2^2 + y3^2*z1^2 + y1^2*z4^2 + y2^2*z3^2 + y3^2*z2^2 + y4^2*z1^2 + y2^2*z4^2 + y3^2*z3^2 + y4^2*z2^2 + y3^2*z4^2 + y4^2*z3^2 + y4^2*z4^2 + 4*x1^2 + 4*x2^2 + 4*x3^2 + 4*x4^2 + 8*y1^2 + 8*y2^2 + y1^4 + 8*y3^2 + y2^4 + 8*y4^2 + y3^4 + y4^4 + 4*z1^2 + 4*z2^2 + 4*z3^2 + 4*z4^2 - 2*x1*x2*z1*z2 - 2*x1*x3*z1*z3 - 2*x1*x4*z1*z4 - 2*x2*x3*z2*z3 - 2*x2*x4*z2*z4 - 2*x3*x4*z3*z4 + 16))/(8*x1^2*x2^2 + 8*x1^2*x3^2 + 8*x1^2*x4^2 + 8*x2^2*x3^2 + 8*x2^2*x4^2 + 8*x3^2*x4^2 + 8*x1^2*y1^2 + 12*x1^2*y2^2 + 12*x2^2*y1^2 + 12*x1^2*y3^2 + 8*x2^2*y2^2 + 12*x3^2*y1^2 + x1^2*y2^4 + 12*x1^2*y4^2 + x2^2*y1^4 + 12*x2^2*y3^2 + x1^4*y2^2 + 12*x3^2*y2^2 + x2^4*y1^2 + 12*x4^2*y1^2 + x1^2*y3^4 + 12*x2^2*y4^2 + x1^4*y3^2 + x3^2*y1^4 + 8*x3^2*y3^2 + 12*x4^2*y2^2 + x3^4*y1^2 + x1^2*y4^4 + x2^2*y3^4 + x1^4*y4^2 + x3^2*y2^4 + 12*x3^2*y4^2 + x2^4*y3^2 + x4^2*y1^4 + 12*x4^2*y3^2 + x3^4*y2^2 + x4^4*y1^2 + x2^2*y4^4 + x2^4*y4^2 + x4^2*y2^4 + 8*x4^2*y4^2 + x4^4*y2^2 + x3^2*y4^4 + x4^2*y3^4 + x3^4*y4^2 + x4^4*y3^2 + 8*x1^2*z1^2 + 12*x1^2*z2^2 + 12*x2^2*z1^2 + 8*y1^2*y2^2 + 12*x1^2*z3^2 + 8*x2^2*z2^2 + 12*x3^2*z1^2 + 8*y1^2*y3^2 + x1^2*z2^4 + 12*x1^2*z4^2 + x2^2*z1^4 + 12*x2^2*z3^2 + x1^4*z2^2 + 12*x3^2*z2^2 + x2^4*z1^2 + 12*x4^2*z1^2 + 8*y1^2*y4^2 + 8*y2^2*y3^2 + x1^2*z3^4 + 12*x2^2*z4^2 + x1^4*z3^2 + x3^2*z1^4 + 8*x3^2*z3^2 + 12*x4^2*z2^2 + x3^4*z1^2 + 8*y2^2*y4^2 + x1^2*z4^4 + x2^2*z3^4 + x1^4*z4^2 + x3^2*z2^4 + 12*x3^2*z4^2 + x2^4*z3^2 + x4^2*z1^4 + 12*x4^2*z3^2 + x3^4*z2^2 + x4^4*z1^2 + 8*y3^2*y4^2 + x2^2*z4^4 + x2^4*z4^2 + x4^2*z2^4 + 8*x4^2*z4^2 + x4^4*z2^2 + x3^2*z4^4 + x4^2*z3^4 + x3^4*z4^2 + x4^4*z3^2 + 8*y1^2*z1^2 + 12*y1^2*z2^2 + 12*y2^2*z1^2 + 12*y1^2*z3^2 + 8*y2^2*z2^2 + 12*y3^2*z1^2 + y1^2*z2^4 + 12*y1^2*z4^2 + y2^2*z1^4 + 12*y2^2*z3^2 + y1^4*z2^2 + 12*y3^2*z2^2 + y2^4*z1^2 + 12*y4^2*z1^2 + y1^2*z3^4 + 12*y2^2*z4^2 + y1^4*z3^2 + y3^2*z1^4 + 8*y3^2*z3^2 + 12*y4^2*z2^2 + y3^4*z1^2 + y1^2*z4^4 + y2^2*z3^4 + y1^4*z4^2 + y3^2*z2^4 + 12*y3^2*z4^2 + y2^4*z3^2 + y4^2*z1^4 + 12*y4^2*z3^2 + y3^4*z2^2 + y4^4*z1^2 + y2^2*z4^4 + y2^4*z4^2 + y4^2*z2^4 + 8*y4^2*z4^2 + y4^4*z2^2 + y3^2*z4^4 + y4^2*z3^4 + y3^4*z4^2 + y4^4*z3^2 + 8*z1^2*z2^2 + 8*z1^2*z3^2 + 8*z1^2*z4^2 + 8*z2^2*z3^2 + 8*z2^2*z4^2 + 8*z3^2*z4^2 + 32*x1^2 + 32*x2^2 + 4*x1^4 + 32*x3^2 + 4*x2^4 + 32*x4^2 + 4*x3^4 + 4*x4^4 + 32*y1^2 + 32*y2^2 + 4*y1^4 + 32*y3^2 + 4*y2^4 + 32*y4^2 + 4*y3^4 + 4*y4^4 + 32*z1^2 + 32*z2^2 + 4*z1^4 + 32*z3^2 + 4*z2^4 + 32*z4^2 + 4*z3^4 + 4*z4^4 + x1^2*x2^2*y1^2 + x1^2*x2^2*y2^2 + x1^2*x3^2*y1^2 + 2*x1^2*x2^2*y3^2 + 2*x1^2*x3^2*y2^2 + x1^2*x4^2*y1^2 + 2*x2^2*x3^2*y1^2 + 2*x1^2*x2^2*y4^2 + x1^2*x3^2*y3^2 + 2*x1^2*x4^2*y2^2 + x2^2*x3^2*y2^2 + 2*x2^2*x4^2*y1^2 + 2*x1^2*x3^2*y4^2 + 2*x1^2*x4^2*y3^2 + x2^2*x3^2*y3^2 + x2^2*x4^2*y2^2 + 2*x3^2*x4^2*y1^2 + x1^2*x4^2*y4^2 + 2*x2^2*x3^2*y4^2 + 2*x2^2*x4^2*y3^2 + 2*x3^2*x4^2*y2^2 + x2^2*x4^2*y4^2 + x3^2*x4^2*y3^2 + x3^2*x4^2*y4^2 + x1^2*x2^2*z1^2 + x1^2*y1^2*y2^2 + x1^2*x2^2*z2^2 + x1^2*x3^2*z1^2 + x1^2*y1^2*y3^2 + x2^2*y1^2*y2^2 + 2*x1^2*x2^2*z3^2 + 2*x1^2*x3^2*z2^2 + x1^2*x4^2*z1^2 + x1^2*y1^2*y4^2 + 2*x1^2*y2^2*y3^2 + 2*x2^2*x3^2*z1^2 + 2*x2^2*y1^2*y3^2 + 2*x3^2*y1^2*y2^2 + 2*x1^2*x2^2*z4^2 + x1^2*x3^2*z3^2 + 2*x1^2*x4^2*z2^2 + 2*x1^2*y2^2*y4^2 + x2^2*x3^2*z2^2 + 2*x2^2*x4^2*z1^2 + 2*x2^2*y1^2*y4^2 + x2^2*y2^2*y3^2 + x3^2*y1^2*y3^2 + 2*x4^2*y1^2*y2^2 + 2*x1^2*x3^2*z4^2 + 2*x1^2*x4^2*z3^2 + 2*x1^2*y3^2*y4^2 + x2^2*x3^2*z3^2 + x2^2*x4^2*z2^2 + x2^2*y2^2*y4^2 + 2*x3^2*x4^2*z1^2 + 2*x3^2*y1^2*y4^2 + x3^2*y2^2*y3^2 + 2*x4^2*y1^2*y3^2 + x1^2*x4^2*z4^2 + 2*x2^2*x3^2*z4^2 + 2*x2^2*x4^2*z3^2 + 2*x2^2*y3^2*y4^2 + 2*x3^2*x4^2*z2^2 + 2*x3^2*y2^2*y4^2 + x4^2*y1^2*y4^2 + 2*x4^2*y2^2*y3^2 + x2^2*x4^2*z4^2 + x3^2*x4^2*z3^2 + x3^2*y3^2*y4^2 + x4^2*y2^2*y4^2 + x3^2*x4^2*z4^2 + x4^2*y3^2*y4^2 + 2*x1^2*y1^2*z2^2 + 2*x1^2*y2^2*z1^2 + 2*x2^2*y1^2*z1^2 + 2*x1^2*y1^2*z3^2 + 2*x1^2*y2^2*z2^2 + 2*x1^2*y3^2*z1^2 + 2*x2^2*y1^2*z2^2 + 2*x2^2*y2^2*z1^2 + 2*x3^2*y1^2*z1^2 + 2*x1^2*y1^2*z4^2 + 2*x1^2*y2^2*z3^2 + 2*x1^2*y3^2*z2^2 + 2*x1^2*y4^2*z1^2 + 2*x2^2*y1^2*z3^2 + 2*x2^2*y3^2*z1^2 + 2*x3^2*y1^2*z2^2 + 2*x3^2*y2^2*z1^2 + 2*x4^2*y1^2*z1^2 + 2*x1^2*y2^2*z4^2 + 2*x1^2*y3^2*z3^2 + 2*x1^2*y4^2*z2^2 + 2*x2^2*y1^2*z4^2 + 2*x2^2*y2^2*z3^2 + 2*x2^2*y3^2*z2^2 + 2*x2^2*y4^2*z1^2 + 2*x3^2*y1^2*z3^2 + 2*x3^2*y2^2*z2^2 + 2*x3^2*y3^2*z1^2 + 2*x4^2*y1^2*z2^2 + 2*x4^2*y2^2*z1^2 + 2*x1^2*y3^2*z4^2 + 2*x1^2*y4^2*z3^2 + 2*x2^2*y2^2*z4^2 + 2*x2^2*y3^2*z3^2 + 2*x2^2*y4^2*z2^2 + 2*x3^2*y1^2*z4^2 + 2*x3^2*y2^2*z3^2 + 2*x3^2*y3^2*z2^2 + 2*x3^2*y4^2*z1^2 + 2*x4^2*y1^2*z3^2 + 2*x4^2*y2^2*z2^2 + 2*x4^2*y3^2*z1^2 + 2*x1^2*y4^2*z4^2 + 2*x2^2*y3^2*z4^2 + 2*x2^2*y4^2*z3^2 + 2*x3^2*y2^2*z4^2 + 2*x3^2*y4^2*z2^2 + 2*x4^2*y1^2*z4^2 + 2*x4^2*y2^2*z3^2 + 2*x4^2*y3^2*z2^2 + 2*x4^2*y4^2*z1^2 + 2*x2^2*y4^2*z4^2 + 2*x3^2*y3^2*z4^2 + 2*x3^2*y4^2*z3^2 + 2*x4^2*y2^2*z4^2 + 2*x4^2*y3^2*z3^2 + 2*x4^2*y4^2*z2^2 + 2*x3^2*y4^2*z4^2 + 2*x4^2*y3^2*z4^2 + 2*x4^2*y4^2*z3^2 + x1^2*z1^2*z2^2 + y1^2*y2^2*z1^2 + x1^2*z1^2*z3^2 + x2^2*z1^2*z2^2 + y1^2*y2^2*z2^2 + y1^2*y3^2*z1^2 + x1^2*z1^2*z4^2 + 2*x1^2*z2^2*z3^2 + 2*x2^2*z1^2*z3^2 + 2*x3^2*z1^2*z2^2 + 2*y1^2*y2^2*z3^2 + 2*y1^2*y3^2*z2^2 + y1^2*y4^2*z1^2 + 2*y2^2*y3^2*z1^2 + 2*x1^2*z2^2*z4^2 + 2*x2^2*z1^2*z4^2 + x2^2*z2^2*z3^2 + x3^2*z1^2*z3^2 + 2*x4^2*z1^2*z2^2 + 2*y1^2*y2^2*z4^2 + y1^2*y3^2*z3^2 + 2*y1^2*y4^2*z2^2 + y2^2*y3^2*z2^2 + 2*y2^2*y4^2*z1^2 + 2*x1^2*z3^2*z4^2 + x2^2*z2^2*z4^2 + 2*x3^2*z1^2*z4^2 + x3^2*z2^2*z3^2 + 2*x4^2*z1^2*z3^2 + 2*y1^2*y3^2*z4^2 + 2*y1^2*y4^2*z3^2 + y2^2*y3^2*z3^2 + y2^2*y4^2*z2^2 + 2*y3^2*y4^2*z1^2 + 2*x2^2*z3^2*z4^2 + 2*x3^2*z2^2*z4^2 + x4^2*z1^2*z4^2 + 2*x4^2*z2^2*z3^2 + y1^2*y4^2*z4^2 + 2*y2^2*y3^2*z4^2 + 2*y2^2*y4^2*z3^2 + 2*y3^2*y4^2*z2^2 + x3^2*z3^2*z4^2 + x4^2*z2^2*z4^2 + y2^2*y4^2*z4^2 + y3^2*y4^2*z3^2 + x4^2*z3^2*z4^2 + y3^2*y4^2*z4^2 + y1^2*z1^2*z2^2 + y1^2*z1^2*z3^2 + y2^2*z1^2*z2^2 + y1^2*z1^2*z4^2 + 2*y1^2*z2^2*z3^2 + 2*y2^2*z1^2*z3^2 + 2*y3^2*z1^2*z2^2 + 2*y1^2*z2^2*z4^2 + 2*y2^2*z1^2*z4^2 + y2^2*z2^2*z3^2 + y3^2*z1^2*z3^2 + 2*y4^2*z1^2*z2^2 + 2*y1^2*z3^2*z4^2 + y2^2*z2^2*z4^2 + 2*y3^2*z1^2*z4^2 + y3^2*z2^2*z3^2 + 2*y4^2*z1^2*z3^2 + 2*y2^2*z3^2*z4^2 + 2*y3^2*z2^2*z4^2 + y4^2*z1^2*z4^2 + 2*y4^2*z2^2*z3^2 + y3^2*z3^2*z4^2 + y4^2*z2^2*z4^2 + y4^2*z3^2*z4^2 - 8*x1*x2*y1*y2 - 8*x1*x3*y1*y3 - 8*x1*x4*y1*y4 - 8*x2*x3*y2*y3 - 8*x2*x4*y2*y4 - 8*x3*x4*y3*y4 - 8*x1*x2*z1*z2 - 8*x1*x3*z1*z3 - 8*x1*x4*z1*z4 - 8*x2*x3*z2*z3 - 8*x2*x4*z2*z4 - 8*x3*x4*z3*z4 - 8*y1*y2*z1*z2 - 8*y1*y3*z1*z3 - 8*y1*y4*z1*z4 - 8*y2*y3*z2*z3 - 8*y2*y4*z2*z4 - 8*y3*y4*z3*z4 - 2*x1*x2*y1*y2^3 - 2*x1*x2*y1^3*y2 - 2*x1*x2^3*y1*y2 - 2*x1^3*x2*y1*y2 - 2*x1*x3*y1*y3^3 - 2*x1*x3*y1^3*y3 - 2*x1*x3^3*y1*y3 - 2*x1^3*x3*y1*y3 - 2*x1*x4*y1*y4^3 - 2*x1*x4*y1^3*y4 - 2*x1*x4^3*y1*y4 - 2*x2*x3*y2*y3^3 - 2*x2*x3*y2^3*y3 - 2*x2*x3^3*y2*y3 - 2*x1^3*x4*y1*y4 - 2*x2^3*x3*y2*y3 - 2*x2*x4*y2*y4^3 - 2*x2*x4*y2^3*y4 - 2*x2*x4^3*y2*y4 - 2*x2^3*x4*y2*y4 - 2*x3*x4*y3*y4^3 - 2*x3*x4*y3^3*y4 - 2*x3*x4^3*y3*y4 - 2*x3^3*x4*y3*y4 - 2*x1*x2*z1*z2^3 - 2*x1*x2*z1^3*z2 - 2*x1*x2^3*z1*z2 - 2*x1^3*x2*z1*z2 - 2*x1*x3*z1*z3^3 - 2*x1*x3*z1^3*z3 - 2*x1*x3^3*z1*z3 - 2*x1^3*x3*z1*z3 - 2*x1*x4*z1*z4^3 - 2*x1*x4*z1^3*z4 - 2*x1*x4^3*z1*z4 - 2*x2*x3*z2*z3^3 - 2*x2*x3*z2^3*z3 - 2*x2*x3^3*z2*z3 - 2*x1^3*x4*z1*z4 - 2*x2^3*x3*z2*z3 - 2*x2*x4*z2*z4^3 - 2*x2*x4*z2^3*z4 - 2*x2*x4^3*z2*z4 - 2*x2^3*x4*z2*z4 - 2*x3*x4*z3*z4^3 - 2*x3*x4*z3^3*z4 - 2*x3*x4^3*z3*z4 - 2*x3^3*x4*z3*z4 - 2*y1*y2*z1*z2^3 - 2*y1*y2*z1^3*z2 - 2*y1*y2^3*z1*z2 - 2*y1^3*y2*z1*z2 - 2*y1*y3*z1*z3^3 - 2*y1*y3*z1^3*z3 - 2*y1*y3^3*z1*z3 - 2*y1^3*y3*z1*z3 - 2*y1*y4*z1*z4^3 - 2*y1*y4*z1^3*z4 - 2*y1*y4^3*z1*z4 - 2*y2*y3*z2*z3^3 - 2*y2*y3*z2^3*z3 - 2*y2*y3^3*z2*z3 - 2*y1^3*y4*z1*z4 - 2*y2^3*y3*z2*z3 - 2*y2*y4*z2*z4^3 - 2*y2*y4*z2^3*z4 - 2*y2*y4^3*z2*z4 - 2*y2^3*y4*z2*z4 - 2*y3*y4*z3*z4^3 - 2*y3*y4*z3^3*z4 - 2*y3*y4^3*z3*z4 - 2*y3^3*y4*z3*z4 - 2*x1*x2*x3^2*y1*y2 - 2*x1*x2*x4^2*y1*y2 - 2*x1*x2^2*x3*y1*y3 - 2*x1^2*x2*x3*y2*y3 - 2*x1*x3*x4^2*y1*y3 - 2*x1*x2^2*x4*y1*y4 - 2*x1*x3^2*x4*y1*y4 - 2*x1^2*x2*x4*y2*y4 - 2*x2*x3*x4^2*y2*y3 - 2*x2*x3^2*x4*y2*y4 - 2*x1^2*x3*x4*y3*y4 - 2*x2^2*x3*x4*y3*y4 - 2*x1*x2*y1*y2*y3^2 - 2*x1*x2*y1*y2*y4^2 - 2*x1*x3*y1*y2^2*y3 - 2*x2*x3*y1^2*y2*y3 - 2*x1*x3*y1*y3*y4^2 - 2*x1*x4*y1*y2^2*y4 - 2*x1*x4*y1*y3^2*y4 - 2*x2*x4*y1^2*y2*y4 - 2*x2*x3*y2*y3*y4^2 - 2*x2*x4*y2*y3^2*y4 - 2*x3*x4*y1^2*y3*y4 - 2*x3*x4*y2^2*y3*y4 - 2*x1*x2*y1*y2*z1^2 - 2*x1*x2*y1*y2*z2^2 - 2*x1*x2*x3^2*z1*z2 - 2*x1*x3*y1*y3*z1^2 - 2*x1*x2*x4^2*z1*z2 - 2*x1*x2^2*x3*z1*z3 - 2*x1*x3*y1*y3*z3^2 - 2*x1*x4*y1*y4*z1^2 - 2*x1^2*x2*x3*z2*z3 - 2*x1*x3*x4^2*z1*z3 - 2*x1*x2^2*x4*z1*z4 - 2*x2*x3*y2*y3*z2^2 - 2*x1*x3^2*x4*z1*z4 - 2*x2*x3*y2*y3*z3^2 - 2*x1^2*x2*x4*z2*z4 - 2*x1*x4*y1*y4*z4^2 - 2*x2*x3*x4^2*z2*z3 - 2*x2*x4*y2*y4*z2^2 - 2*x2*x3^2*x4*z2*z4 - 2*x1^2*x3*x4*z3*z4 - 2*x2*x4*y2*y4*z4^2 - 2*x2^2*x3*x4*z3*z4 - 2*x3*x4*y3*y4*z3^2 - 2*x3*x4*y3*y4*z4^2 - 2*x1*x2*y1^2*z1*z2 - 2*x1*x2*y2^2*z1*z2 - 2*x1*x3*y1^2*z1*z3 - 2*x1*x3*y3^2*z1*z3 - 2*x1*x4*y1^2*z1*z4 - 2*x2*x3*y2^2*z2*z3 - 2*x2*x3*y3^2*z2*z3 - 2*x1*x4*y4^2*z1*z4 - 2*x2*x4*y2^2*z2*z4 - 2*x2*x4*y4^2*z2*z4 - 2*x3*x4*y3^2*z3*z4 - 2*x3*x4*y4^2*z3*z4 - 2*x1^2*y1*y2*z1*z2 - 2*x2^2*y1*y2*z1*z2 - 2*x1*x2*z1*z2*z3^2 - 2*x1^2*y1*y3*z1*z3 - 2*x1*x2*z1*z2*z4^2 - 2*x1*x3*z1*z2^2*z3 - 2*x2*x3*z1^2*z2*z3 - 2*x1^2*y1*y4*z1*z4 - 2*x3^2*y1*y3*z1*z3 - 2*x1*x3*z1*z3*z4^2 - 2*x1*x4*z1*z2^2*z4 - 2*x2^2*y2*y3*z2*z3 - 2*x1*x4*z1*z3^2*z4 - 2*x2*x4*z1^2*z2*z4 - 2*x3^2*y2*y3*z2*z3 - 2*x2*x3*z2*z3*z4^2 - 2*x2^2*y2*y4*z2*z4 - 2*x4^2*y1*y4*z1*z4 - 2*x2*x4*z2*z3^2*z4 - 2*x3*x4*z1^2*z3*z4 - 2*x3*x4*z2^2*z3*z4 - 2*x4^2*y2*y4*z2*z4 - 2*x3^2*y3*y4*z3*z4 - 2*x4^2*y3*y4*z3*z4 - 2*y1*y2*y3^2*z1*z2 - 2*y1*y2*y4^2*z1*z2 - 2*y1*y2^2*y3*z1*z3 - 2*y1^2*y2*y3*z2*z3 - 2*y1*y3*y4^2*z1*z3 - 2*y1*y2^2*y4*z1*z4 - 2*y1*y3^2*y4*z1*z4 - 2*y1^2*y2*y4*z2*z4 - 2*y2*y3*y4^2*z2*z3 - 2*y2*y3^2*y4*z2*z4 - 2*y1^2*y3*y4*z3*z4 - 2*y2^2*y3*y4*z3*z4 - 2*y1*y2*z1*z2*z3^2 - 2*y1*y2*z1*z2*z4^2 - 2*y1*y3*z1*z2^2*z3 - 2*y2*y3*z1^2*z2*z3 - 2*y1*y3*z1*z3*z4^2 - 2*y1*y4*z1*z2^2*z4 - 2*y1*y4*z1*z3^2*z4 - 2*y2*y4*z1^2*z2*z4 - 2*y2*y3*z2*z3*z4^2 - 2*y2*y4*z2*z3^2*z4 - 2*y3*y4*z1^2*z3*z4 - 2*y3*y4*z2^2*z3*z4 - 2*x1*x2*y1*y3*z2*z3 - 2*x1*x2*y2*y3*z1*z3 - 2*x1*x3*y1*y2*z2*z3 - 2*x1*x3*y2*y3*z1*z2 - 2*x2*x3*y1*y2*z1*z3 - 2*x2*x3*y1*y3*z1*z2 - 2*x1*x2*y1*y4*z2*z4 - 2*x1*x2*y2*y4*z1*z4 - 2*x1*x4*y1*y2*z2*z4 - 2*x1*x4*y2*y4*z1*z2 - 2*x2*x4*y1*y2*z1*z4 - 2*x2*x4*y1*y4*z1*z2 - 2*x1*x3*y1*y4*z3*z4 - 2*x1*x3*y3*y4*z1*z4 - 2*x1*x4*y1*y3*z3*z4 - 2*x1*x4*y3*y4*z1*z3 - 2*x3*x4*y1*y3*z1*z4 - 2*x3*x4*y1*y4*z1*z3 - 2*x2*x3*y2*y4*z3*z4 - 2*x2*x3*y3*y4*z2*z4 - 2*x2*x4*y2*y3*z3*z4 - 2*x2*x4*y3*y4*z2*z3 - 2*x3*x4*y2*y3*z2*z4 - 2*x3*x4*y2*y4*z2*z3 + 64),...
        (4*(4*y1*z1 + 4*y2*z2 + 4*y3*z3 + 4*y4*z4 + y1*z1^3 + y1^3*z1 + y2*z2^3 + y2^3*z2 + y3*z3^3 + y3^3*z3 + y4*z4^3 + y4^3*z4 + x1^2*y1*z1 + x2^2*y2*z2 + x3^2*y3*z3 + x4^2*y4*z4 + y1*y2^2*z1 + y1*y3^2*z1 + y1^2*y2*z2 + y1*y4^2*z1 + y2*y3^2*z2 + y1^2*y3*z3 + y2*y4^2*z2 + y2^2*y3*z3 + y1^2*y4*z4 + y3*y4^2*z3 + y2^2*y4*z4 + y3^2*y4*z4 + y1*z1*z2^2 + y1*z1*z3^2 + y2*z1^2*z2 + y1*z1*z4^2 + y2*z2*z3^2 + y3*z1^2*z3 + y2*z2*z4^2 + y3*z2^2*z3 + y4*z1^2*z4 + y3*z3*z4^2 + y4*z2^2*z4 + y4*z3^2*z4 + x1*x2*y1*z2 + x1*x2*y2*z1 + x1*x3*y1*z3 + x1*x3*y3*z1 + x1*x4*y1*z4 + x1*x4*y4*z1 + x2*x3*y2*z3 + x2*x3*y3*z2 + x2*x4*y2*z4 + x2*x4*y4*z2 + x3*x4*y3*z4 + x3*x4*y4*z3))/(8*x1^2*x2^2 + 8*x1^2*x3^2 + 8*x1^2*x4^2 + 8*x2^2*x3^2 + 8*x2^2*x4^2 + 8*x3^2*x4^2 + 8*x1^2*y1^2 + 12*x1^2*y2^2 + 12*x2^2*y1^2 + 12*x1^2*y3^2 + 8*x2^2*y2^2 + 12*x3^2*y1^2 + x1^2*y2^4 + 12*x1^2*y4^2 + x2^2*y1^4 + 12*x2^2*y3^2 + x1^4*y2^2 + 12*x3^2*y2^2 + x2^4*y1^2 + 12*x4^2*y1^2 + x1^2*y3^4 + 12*x2^2*y4^2 + x1^4*y3^2 + x3^2*y1^4 + 8*x3^2*y3^2 + 12*x4^2*y2^2 + x3^4*y1^2 + x1^2*y4^4 + x2^2*y3^4 + x1^4*y4^2 + x3^2*y2^4 + 12*x3^2*y4^2 + x2^4*y3^2 + x4^2*y1^4 + 12*x4^2*y3^2 + x3^4*y2^2 + x4^4*y1^2 + x2^2*y4^4 + x2^4*y4^2 + x4^2*y2^4 + 8*x4^2*y4^2 + x4^4*y2^2 + x3^2*y4^4 + x4^2*y3^4 + x3^4*y4^2 + x4^4*y3^2 + 8*x1^2*z1^2 + 12*x1^2*z2^2 + 12*x2^2*z1^2 + 8*y1^2*y2^2 + 12*x1^2*z3^2 + 8*x2^2*z2^2 + 12*x3^2*z1^2 + 8*y1^2*y3^2 + x1^2*z2^4 + 12*x1^2*z4^2 + x2^2*z1^4 + 12*x2^2*z3^2 + x1^4*z2^2 + 12*x3^2*z2^2 + x2^4*z1^2 + 12*x4^2*z1^2 + 8*y1^2*y4^2 + 8*y2^2*y3^2 + x1^2*z3^4 + 12*x2^2*z4^2 + x1^4*z3^2 + x3^2*z1^4 + 8*x3^2*z3^2 + 12*x4^2*z2^2 + x3^4*z1^2 + 8*y2^2*y4^2 + x1^2*z4^4 + x2^2*z3^4 + x1^4*z4^2 + x3^2*z2^4 + 12*x3^2*z4^2 + x2^4*z3^2 + x4^2*z1^4 + 12*x4^2*z3^2 + x3^4*z2^2 + x4^4*z1^2 + 8*y3^2*y4^2 + x2^2*z4^4 + x2^4*z4^2 + x4^2*z2^4 + 8*x4^2*z4^2 + x4^4*z2^2 + x3^2*z4^4 + x4^2*z3^4 + x3^4*z4^2 + x4^4*z3^2 + 8*y1^2*z1^2 + 12*y1^2*z2^2 + 12*y2^2*z1^2 + 12*y1^2*z3^2 + 8*y2^2*z2^2 + 12*y3^2*z1^2 + y1^2*z2^4 + 12*y1^2*z4^2 + y2^2*z1^4 + 12*y2^2*z3^2 + y1^4*z2^2 + 12*y3^2*z2^2 + y2^4*z1^2 + 12*y4^2*z1^2 + y1^2*z3^4 + 12*y2^2*z4^2 + y1^4*z3^2 + y3^2*z1^4 + 8*y3^2*z3^2 + 12*y4^2*z2^2 + y3^4*z1^2 + y1^2*z4^4 + y2^2*z3^4 + y1^4*z4^2 + y3^2*z2^4 + 12*y3^2*z4^2 + y2^4*z3^2 + y4^2*z1^4 + 12*y4^2*z3^2 + y3^4*z2^2 + y4^4*z1^2 + y2^2*z4^4 + y2^4*z4^2 + y4^2*z2^4 + 8*y4^2*z4^2 + y4^4*z2^2 + y3^2*z4^4 + y4^2*z3^4 + y3^4*z4^2 + y4^4*z3^2 + 8*z1^2*z2^2 + 8*z1^2*z3^2 + 8*z1^2*z4^2 + 8*z2^2*z3^2 + 8*z2^2*z4^2 + 8*z3^2*z4^2 + 32*x1^2 + 32*x2^2 + 4*x1^4 + 32*x3^2 + 4*x2^4 + 32*x4^2 + 4*x3^4 + 4*x4^4 + 32*y1^2 + 32*y2^2 + 4*y1^4 + 32*y3^2 + 4*y2^4 + 32*y4^2 + 4*y3^4 + 4*y4^4 + 32*z1^2 + 32*z2^2 + 4*z1^4 + 32*z3^2 + 4*z2^4 + 32*z4^2 + 4*z3^4 + 4*z4^4 + x1^2*x2^2*y1^2 + x1^2*x2^2*y2^2 + x1^2*x3^2*y1^2 + 2*x1^2*x2^2*y3^2 + 2*x1^2*x3^2*y2^2 + x1^2*x4^2*y1^2 + 2*x2^2*x3^2*y1^2 + 2*x1^2*x2^2*y4^2 + x1^2*x3^2*y3^2 + 2*x1^2*x4^2*y2^2 + x2^2*x3^2*y2^2 + 2*x2^2*x4^2*y1^2 + 2*x1^2*x3^2*y4^2 + 2*x1^2*x4^2*y3^2 + x2^2*x3^2*y3^2 + x2^2*x4^2*y2^2 + 2*x3^2*x4^2*y1^2 + x1^2*x4^2*y4^2 + 2*x2^2*x3^2*y4^2 + 2*x2^2*x4^2*y3^2 + 2*x3^2*x4^2*y2^2 + x2^2*x4^2*y4^2 + x3^2*x4^2*y3^2 + x3^2*x4^2*y4^2 + x1^2*x2^2*z1^2 + x1^2*y1^2*y2^2 + x1^2*x2^2*z2^2 + x1^2*x3^2*z1^2 + x1^2*y1^2*y3^2 + x2^2*y1^2*y2^2 + 2*x1^2*x2^2*z3^2 + 2*x1^2*x3^2*z2^2 + x1^2*x4^2*z1^2 + x1^2*y1^2*y4^2 + 2*x1^2*y2^2*y3^2 + 2*x2^2*x3^2*z1^2 + 2*x2^2*y1^2*y3^2 + 2*x3^2*y1^2*y2^2 + 2*x1^2*x2^2*z4^2 + x1^2*x3^2*z3^2 + 2*x1^2*x4^2*z2^2 + 2*x1^2*y2^2*y4^2 + x2^2*x3^2*z2^2 + 2*x2^2*x4^2*z1^2 + 2*x2^2*y1^2*y4^2 + x2^2*y2^2*y3^2 + x3^2*y1^2*y3^2 + 2*x4^2*y1^2*y2^2 + 2*x1^2*x3^2*z4^2 + 2*x1^2*x4^2*z3^2 + 2*x1^2*y3^2*y4^2 + x2^2*x3^2*z3^2 + x2^2*x4^2*z2^2 + x2^2*y2^2*y4^2 + 2*x3^2*x4^2*z1^2 + 2*x3^2*y1^2*y4^2 + x3^2*y2^2*y3^2 + 2*x4^2*y1^2*y3^2 + x1^2*x4^2*z4^2 + 2*x2^2*x3^2*z4^2 + 2*x2^2*x4^2*z3^2 + 2*x2^2*y3^2*y4^2 + 2*x3^2*x4^2*z2^2 + 2*x3^2*y2^2*y4^2 + x4^2*y1^2*y4^2 + 2*x4^2*y2^2*y3^2 + x2^2*x4^2*z4^2 + x3^2*x4^2*z3^2 + x3^2*y3^2*y4^2 + x4^2*y2^2*y4^2 + x3^2*x4^2*z4^2 + x4^2*y3^2*y4^2 + 2*x1^2*y1^2*z2^2 + 2*x1^2*y2^2*z1^2 + 2*x2^2*y1^2*z1^2 + 2*x1^2*y1^2*z3^2 + 2*x1^2*y2^2*z2^2 + 2*x1^2*y3^2*z1^2 + 2*x2^2*y1^2*z2^2 + 2*x2^2*y2^2*z1^2 + 2*x3^2*y1^2*z1^2 + 2*x1^2*y1^2*z4^2 + 2*x1^2*y2^2*z3^2 + 2*x1^2*y3^2*z2^2 + 2*x1^2*y4^2*z1^2 + 2*x2^2*y1^2*z3^2 + 2*x2^2*y3^2*z1^2 + 2*x3^2*y1^2*z2^2 + 2*x3^2*y2^2*z1^2 + 2*x4^2*y1^2*z1^2 + 2*x1^2*y2^2*z4^2 + 2*x1^2*y3^2*z3^2 + 2*x1^2*y4^2*z2^2 + 2*x2^2*y1^2*z4^2 + 2*x2^2*y2^2*z3^2 + 2*x2^2*y3^2*z2^2 + 2*x2^2*y4^2*z1^2 + 2*x3^2*y1^2*z3^2 + 2*x3^2*y2^2*z2^2 + 2*x3^2*y3^2*z1^2 + 2*x4^2*y1^2*z2^2 + 2*x4^2*y2^2*z1^2 + 2*x1^2*y3^2*z4^2 + 2*x1^2*y4^2*z3^2 + 2*x2^2*y2^2*z4^2 + 2*x2^2*y3^2*z3^2 + 2*x2^2*y4^2*z2^2 + 2*x3^2*y1^2*z4^2 + 2*x3^2*y2^2*z3^2 + 2*x3^2*y3^2*z2^2 + 2*x3^2*y4^2*z1^2 + 2*x4^2*y1^2*z3^2 + 2*x4^2*y2^2*z2^2 + 2*x4^2*y3^2*z1^2 + 2*x1^2*y4^2*z4^2 + 2*x2^2*y3^2*z4^2 + 2*x2^2*y4^2*z3^2 + 2*x3^2*y2^2*z4^2 + 2*x3^2*y4^2*z2^2 + 2*x4^2*y1^2*z4^2 + 2*x4^2*y2^2*z3^2 + 2*x4^2*y3^2*z2^2 + 2*x4^2*y4^2*z1^2 + 2*x2^2*y4^2*z4^2 + 2*x3^2*y3^2*z4^2 + 2*x3^2*y4^2*z3^2 + 2*x4^2*y2^2*z4^2 + 2*x4^2*y3^2*z3^2 + 2*x4^2*y4^2*z2^2 + 2*x3^2*y4^2*z4^2 + 2*x4^2*y3^2*z4^2 + 2*x4^2*y4^2*z3^2 + x1^2*z1^2*z2^2 + y1^2*y2^2*z1^2 + x1^2*z1^2*z3^2 + x2^2*z1^2*z2^2 + y1^2*y2^2*z2^2 + y1^2*y3^2*z1^2 + x1^2*z1^2*z4^2 + 2*x1^2*z2^2*z3^2 + 2*x2^2*z1^2*z3^2 + 2*x3^2*z1^2*z2^2 + 2*y1^2*y2^2*z3^2 + 2*y1^2*y3^2*z2^2 + y1^2*y4^2*z1^2 + 2*y2^2*y3^2*z1^2 + 2*x1^2*z2^2*z4^2 + 2*x2^2*z1^2*z4^2 + x2^2*z2^2*z3^2 + x3^2*z1^2*z3^2 + 2*x4^2*z1^2*z2^2 + 2*y1^2*y2^2*z4^2 + y1^2*y3^2*z3^2 + 2*y1^2*y4^2*z2^2 + y2^2*y3^2*z2^2 + 2*y2^2*y4^2*z1^2 + 2*x1^2*z3^2*z4^2 + x2^2*z2^2*z4^2 + 2*x3^2*z1^2*z4^2 + x3^2*z2^2*z3^2 + 2*x4^2*z1^2*z3^2 + 2*y1^2*y3^2*z4^2 + 2*y1^2*y4^2*z3^2 + y2^2*y3^2*z3^2 + y2^2*y4^2*z2^2 + 2*y3^2*y4^2*z1^2 + 2*x2^2*z3^2*z4^2 + 2*x3^2*z2^2*z4^2 + x4^2*z1^2*z4^2 + 2*x4^2*z2^2*z3^2 + y1^2*y4^2*z4^2 + 2*y2^2*y3^2*z4^2 + 2*y2^2*y4^2*z3^2 + 2*y3^2*y4^2*z2^2 + x3^2*z3^2*z4^2 + x4^2*z2^2*z4^2 + y2^2*y4^2*z4^2 + y3^2*y4^2*z3^2 + x4^2*z3^2*z4^2 + y3^2*y4^2*z4^2 + y1^2*z1^2*z2^2 + y1^2*z1^2*z3^2 + y2^2*z1^2*z2^2 + y1^2*z1^2*z4^2 + 2*y1^2*z2^2*z3^2 + 2*y2^2*z1^2*z3^2 + 2*y3^2*z1^2*z2^2 + 2*y1^2*z2^2*z4^2 + 2*y2^2*z1^2*z4^2 + y2^2*z2^2*z3^2 + y3^2*z1^2*z3^2 + 2*y4^2*z1^2*z2^2 + 2*y1^2*z3^2*z4^2 + y2^2*z2^2*z4^2 + 2*y3^2*z1^2*z4^2 + y3^2*z2^2*z3^2 + 2*y4^2*z1^2*z3^2 + 2*y2^2*z3^2*z4^2 + 2*y3^2*z2^2*z4^2 + y4^2*z1^2*z4^2 + 2*y4^2*z2^2*z3^2 + y3^2*z3^2*z4^2 + y4^2*z2^2*z4^2 + y4^2*z3^2*z4^2 - 8*x1*x2*y1*y2 - 8*x1*x3*y1*y3 - 8*x1*x4*y1*y4 - 8*x2*x3*y2*y3 - 8*x2*x4*y2*y4 - 8*x3*x4*y3*y4 - 8*x1*x2*z1*z2 - 8*x1*x3*z1*z3 - 8*x1*x4*z1*z4 - 8*x2*x3*z2*z3 - 8*x2*x4*z2*z4 - 8*x3*x4*z3*z4 - 8*y1*y2*z1*z2 - 8*y1*y3*z1*z3 - 8*y1*y4*z1*z4 - 8*y2*y3*z2*z3 - 8*y2*y4*z2*z4 - 8*y3*y4*z3*z4 - 2*x1*x2*y1*y2^3 - 2*x1*x2*y1^3*y2 - 2*x1*x2^3*y1*y2 - 2*x1^3*x2*y1*y2 - 2*x1*x3*y1*y3^3 - 2*x1*x3*y1^3*y3 - 2*x1*x3^3*y1*y3 - 2*x1^3*x3*y1*y3 - 2*x1*x4*y1*y4^3 - 2*x1*x4*y1^3*y4 - 2*x1*x4^3*y1*y4 - 2*x2*x3*y2*y3^3 - 2*x2*x3*y2^3*y3 - 2*x2*x3^3*y2*y3 - 2*x1^3*x4*y1*y4 - 2*x2^3*x3*y2*y3 - 2*x2*x4*y2*y4^3 - 2*x2*x4*y2^3*y4 - 2*x2*x4^3*y2*y4 - 2*x2^3*x4*y2*y4 - 2*x3*x4*y3*y4^3 - 2*x3*x4*y3^3*y4 - 2*x3*x4^3*y3*y4 - 2*x3^3*x4*y3*y4 - 2*x1*x2*z1*z2^3 - 2*x1*x2*z1^3*z2 - 2*x1*x2^3*z1*z2 - 2*x1^3*x2*z1*z2 - 2*x1*x3*z1*z3^3 - 2*x1*x3*z1^3*z3 - 2*x1*x3^3*z1*z3 - 2*x1^3*x3*z1*z3 - 2*x1*x4*z1*z4^3 - 2*x1*x4*z1^3*z4 - 2*x1*x4^3*z1*z4 - 2*x2*x3*z2*z3^3 - 2*x2*x3*z2^3*z3 - 2*x2*x3^3*z2*z3 - 2*x1^3*x4*z1*z4 - 2*x2^3*x3*z2*z3 - 2*x2*x4*z2*z4^3 - 2*x2*x4*z2^3*z4 - 2*x2*x4^3*z2*z4 - 2*x2^3*x4*z2*z4 - 2*x3*x4*z3*z4^3 - 2*x3*x4*z3^3*z4 - 2*x3*x4^3*z3*z4 - 2*x3^3*x4*z3*z4 - 2*y1*y2*z1*z2^3 - 2*y1*y2*z1^3*z2 - 2*y1*y2^3*z1*z2 - 2*y1^3*y2*z1*z2 - 2*y1*y3*z1*z3^3 - 2*y1*y3*z1^3*z3 - 2*y1*y3^3*z1*z3 - 2*y1^3*y3*z1*z3 - 2*y1*y4*z1*z4^3 - 2*y1*y4*z1^3*z4 - 2*y1*y4^3*z1*z4 - 2*y2*y3*z2*z3^3 - 2*y2*y3*z2^3*z3 - 2*y2*y3^3*z2*z3 - 2*y1^3*y4*z1*z4 - 2*y2^3*y3*z2*z3 - 2*y2*y4*z2*z4^3 - 2*y2*y4*z2^3*z4 - 2*y2*y4^3*z2*z4 - 2*y2^3*y4*z2*z4 - 2*y3*y4*z3*z4^3 - 2*y3*y4*z3^3*z4 - 2*y3*y4^3*z3*z4 - 2*y3^3*y4*z3*z4 - 2*x1*x2*x3^2*y1*y2 - 2*x1*x2*x4^2*y1*y2 - 2*x1*x2^2*x3*y1*y3 - 2*x1^2*x2*x3*y2*y3 - 2*x1*x3*x4^2*y1*y3 - 2*x1*x2^2*x4*y1*y4 - 2*x1*x3^2*x4*y1*y4 - 2*x1^2*x2*x4*y2*y4 - 2*x2*x3*x4^2*y2*y3 - 2*x2*x3^2*x4*y2*y4 - 2*x1^2*x3*x4*y3*y4 - 2*x2^2*x3*x4*y3*y4 - 2*x1*x2*y1*y2*y3^2 - 2*x1*x2*y1*y2*y4^2 - 2*x1*x3*y1*y2^2*y3 - 2*x2*x3*y1^2*y2*y3 - 2*x1*x3*y1*y3*y4^2 - 2*x1*x4*y1*y2^2*y4 - 2*x1*x4*y1*y3^2*y4 - 2*x2*x4*y1^2*y2*y4 - 2*x2*x3*y2*y3*y4^2 - 2*x2*x4*y2*y3^2*y4 - 2*x3*x4*y1^2*y3*y4 - 2*x3*x4*y2^2*y3*y4 - 2*x1*x2*y1*y2*z1^2 - 2*x1*x2*y1*y2*z2^2 - 2*x1*x2*x3^2*z1*z2 - 2*x1*x3*y1*y3*z1^2 - 2*x1*x2*x4^2*z1*z2 - 2*x1*x2^2*x3*z1*z3 - 2*x1*x3*y1*y3*z3^2 - 2*x1*x4*y1*y4*z1^2 - 2*x1^2*x2*x3*z2*z3 - 2*x1*x3*x4^2*z1*z3 - 2*x1*x2^2*x4*z1*z4 - 2*x2*x3*y2*y3*z2^2 - 2*x1*x3^2*x4*z1*z4 - 2*x2*x3*y2*y3*z3^2 - 2*x1^2*x2*x4*z2*z4 - 2*x1*x4*y1*y4*z4^2 - 2*x2*x3*x4^2*z2*z3 - 2*x2*x4*y2*y4*z2^2 - 2*x2*x3^2*x4*z2*z4 - 2*x1^2*x3*x4*z3*z4 - 2*x2*x4*y2*y4*z4^2 - 2*x2^2*x3*x4*z3*z4 - 2*x3*x4*y3*y4*z3^2 - 2*x3*x4*y3*y4*z4^2 - 2*x1*x2*y1^2*z1*z2 - 2*x1*x2*y2^2*z1*z2 - 2*x1*x3*y1^2*z1*z3 - 2*x1*x3*y3^2*z1*z3 - 2*x1*x4*y1^2*z1*z4 - 2*x2*x3*y2^2*z2*z3 - 2*x2*x3*y3^2*z2*z3 - 2*x1*x4*y4^2*z1*z4 - 2*x2*x4*y2^2*z2*z4 - 2*x2*x4*y4^2*z2*z4 - 2*x3*x4*y3^2*z3*z4 - 2*x3*x4*y4^2*z3*z4 - 2*x1^2*y1*y2*z1*z2 - 2*x2^2*y1*y2*z1*z2 - 2*x1*x2*z1*z2*z3^2 - 2*x1^2*y1*y3*z1*z3 - 2*x1*x2*z1*z2*z4^2 - 2*x1*x3*z1*z2^2*z3 - 2*x2*x3*z1^2*z2*z3 - 2*x1^2*y1*y4*z1*z4 - 2*x3^2*y1*y3*z1*z3 - 2*x1*x3*z1*z3*z4^2 - 2*x1*x4*z1*z2^2*z4 - 2*x2^2*y2*y3*z2*z3 - 2*x1*x4*z1*z3^2*z4 - 2*x2*x4*z1^2*z2*z4 - 2*x3^2*y2*y3*z2*z3 - 2*x2*x3*z2*z3*z4^2 - 2*x2^2*y2*y4*z2*z4 - 2*x4^2*y1*y4*z1*z4 - 2*x2*x4*z2*z3^2*z4 - 2*x3*x4*z1^2*z3*z4 - 2*x3*x4*z2^2*z3*z4 - 2*x4^2*y2*y4*z2*z4 - 2*x3^2*y3*y4*z3*z4 - 2*x4^2*y3*y4*z3*z4 - 2*y1*y2*y3^2*z1*z2 - 2*y1*y2*y4^2*z1*z2 - 2*y1*y2^2*y3*z1*z3 - 2*y1^2*y2*y3*z2*z3 - 2*y1*y3*y4^2*z1*z3 - 2*y1*y2^2*y4*z1*z4 - 2*y1*y3^2*y4*z1*z4 - 2*y1^2*y2*y4*z2*z4 - 2*y2*y3*y4^2*z2*z3 - 2*y2*y3^2*y4*z2*z4 - 2*y1^2*y3*y4*z3*z4 - 2*y2^2*y3*y4*z3*z4 - 2*y1*y2*z1*z2*z3^2 - 2*y1*y2*z1*z2*z4^2 - 2*y1*y3*z1*z2^2*z3 - 2*y2*y3*z1^2*z2*z3 - 2*y1*y3*z1*z3*z4^2 - 2*y1*y4*z1*z2^2*z4 - 2*y1*y4*z1*z3^2*z4 - 2*y2*y4*z1^2*z2*z4 - 2*y2*y3*z2*z3*z4^2 - 2*y2*y4*z2*z3^2*z4 - 2*y3*y4*z1^2*z3*z4 - 2*y3*y4*z2^2*z3*z4 - 2*x1*x2*y1*y3*z2*z3 - 2*x1*x2*y2*y3*z1*z3 - 2*x1*x3*y1*y2*z2*z3 - 2*x1*x3*y2*y3*z1*z2 - 2*x2*x3*y1*y2*z1*z3 - 2*x2*x3*y1*y3*z1*z2 - 2*x1*x2*y1*y4*z2*z4 - 2*x1*x2*y2*y4*z1*z4 - 2*x1*x4*y1*y2*z2*z4 - 2*x1*x4*y2*y4*z1*z2 - 2*x2*x4*y1*y2*z1*z4 - 2*x2*x4*y1*y4*z1*z2 - 2*x1*x3*y1*y4*z3*z4 - 2*x1*x3*y3*y4*z1*z4 - 2*x1*x4*y1*y3*z3*z4 - 2*x1*x4*y3*y4*z1*z3 - 2*x3*x4*y1*y3*z1*z4 - 2*x3*x4*y1*y4*z1*z3 - 2*x2*x3*y2*y4*z3*z4 - 2*x2*x3*y3*y4*z2*z4 - 2*x2*x4*y2*y3*z3*z4 - 2*x2*x4*y3*y4*z2*z3 - 2*x3*x4*y2*y3*z2*z4 - 2*x3*x4*y2*y4*z2*z3 + 64);
        (4*(4*x1*z1 + 4*x2*z2 + 4*x3*z3 + 4*x4*z4 + x1*z1^3 + x1^3*z1 + x2*z2^3 + x2^3*z2 + x3*z3^3 + x3^3*z3 + x4*z4^3 + x4^3*z4 + x1*x2^2*z1 + x1*x3^2*z1 + x1^2*x2*z2 + x1*x4^2*z1 + x2*x3^2*z2 + x1^2*x3*z3 + x2*x4^2*z2 + x2^2*x3*z3 + x1^2*x4*z4 + x3*x4^2*z3 + x2^2*x4*z4 + x3^2*x4*z4 + x1*y1^2*z1 + x2*y2^2*z2 + x3*y3^2*z3 + x4*y4^2*z4 + x1*z1*z2^2 + x1*z1*z3^2 + x2*z1^2*z2 + x1*z1*z4^2 + x2*z2*z3^2 + x3*z1^2*z3 + x2*z2*z4^2 + x3*z2^2*z3 + x4*z1^2*z4 + x3*z3*z4^2 + x4*z2^2*z4 + x4*z3^2*z4 + x1*y1*y2*z2 + x2*y1*y2*z1 + x1*y1*y3*z3 + x3*y1*y3*z1 + x1*y1*y4*z4 + x2*y2*y3*z3 + x3*y2*y3*z2 + x4*y1*y4*z1 + x2*y2*y4*z4 + x4*y2*y4*z2 + x3*y3*y4*z4 + x4*y3*y4*z3))/(8*x1^2*x2^2 + 8*x1^2*x3^2 + 8*x1^2*x4^2 + 8*x2^2*x3^2 + 8*x2^2*x4^2 + 8*x3^2*x4^2 + 8*x1^2*y1^2 + 12*x1^2*y2^2 + 12*x2^2*y1^2 + 12*x1^2*y3^2 + 8*x2^2*y2^2 + 12*x3^2*y1^2 + x1^2*y2^4 + 12*x1^2*y4^2 + x2^2*y1^4 + 12*x2^2*y3^2 + x1^4*y2^2 + 12*x3^2*y2^2 + x2^4*y1^2 + 12*x4^2*y1^2 + x1^2*y3^4 + 12*x2^2*y4^2 + x1^4*y3^2 + x3^2*y1^4 + 8*x3^2*y3^2 + 12*x4^2*y2^2 + x3^4*y1^2 + x1^2*y4^4 + x2^2*y3^4 + x1^4*y4^2 + x3^2*y2^4 + 12*x3^2*y4^2 + x2^4*y3^2 + x4^2*y1^4 + 12*x4^2*y3^2 + x3^4*y2^2 + x4^4*y1^2 + x2^2*y4^4 + x2^4*y4^2 + x4^2*y2^4 + 8*x4^2*y4^2 + x4^4*y2^2 + x3^2*y4^4 + x4^2*y3^4 + x3^4*y4^2 + x4^4*y3^2 + 8*x1^2*z1^2 + 12*x1^2*z2^2 + 12*x2^2*z1^2 + 8*y1^2*y2^2 + 12*x1^2*z3^2 + 8*x2^2*z2^2 + 12*x3^2*z1^2 + 8*y1^2*y3^2 + x1^2*z2^4 + 12*x1^2*z4^2 + x2^2*z1^4 + 12*x2^2*z3^2 + x1^4*z2^2 + 12*x3^2*z2^2 + x2^4*z1^2 + 12*x4^2*z1^2 + 8*y1^2*y4^2 + 8*y2^2*y3^2 + x1^2*z3^4 + 12*x2^2*z4^2 + x1^4*z3^2 + x3^2*z1^4 + 8*x3^2*z3^2 + 12*x4^2*z2^2 + x3^4*z1^2 + 8*y2^2*y4^2 + x1^2*z4^4 + x2^2*z3^4 + x1^4*z4^2 + x3^2*z2^4 + 12*x3^2*z4^2 + x2^4*z3^2 + x4^2*z1^4 + 12*x4^2*z3^2 + x3^4*z2^2 + x4^4*z1^2 + 8*y3^2*y4^2 + x2^2*z4^4 + x2^4*z4^2 + x4^2*z2^4 + 8*x4^2*z4^2 + x4^4*z2^2 + x3^2*z4^4 + x4^2*z3^4 + x3^4*z4^2 + x4^4*z3^2 + 8*y1^2*z1^2 + 12*y1^2*z2^2 + 12*y2^2*z1^2 + 12*y1^2*z3^2 + 8*y2^2*z2^2 + 12*y3^2*z1^2 + y1^2*z2^4 + 12*y1^2*z4^2 + y2^2*z1^4 + 12*y2^2*z3^2 + y1^4*z2^2 + 12*y3^2*z2^2 + y2^4*z1^2 + 12*y4^2*z1^2 + y1^2*z3^4 + 12*y2^2*z4^2 + y1^4*z3^2 + y3^2*z1^4 + 8*y3^2*z3^2 + 12*y4^2*z2^2 + y3^4*z1^2 + y1^2*z4^4 + y2^2*z3^4 + y1^4*z4^2 + y3^2*z2^4 + 12*y3^2*z4^2 + y2^4*z3^2 + y4^2*z1^4 + 12*y4^2*z3^2 + y3^4*z2^2 + y4^4*z1^2 + y2^2*z4^4 + y2^4*z4^2 + y4^2*z2^4 + 8*y4^2*z4^2 + y4^4*z2^2 + y3^2*z4^4 + y4^2*z3^4 + y3^4*z4^2 + y4^4*z3^2 + 8*z1^2*z2^2 + 8*z1^2*z3^2 + 8*z1^2*z4^2 + 8*z2^2*z3^2 + 8*z2^2*z4^2 + 8*z3^2*z4^2 + 32*x1^2 + 32*x2^2 + 4*x1^4 + 32*x3^2 + 4*x2^4 + 32*x4^2 + 4*x3^4 + 4*x4^4 + 32*y1^2 + 32*y2^2 + 4*y1^4 + 32*y3^2 + 4*y2^4 + 32*y4^2 + 4*y3^4 + 4*y4^4 + 32*z1^2 + 32*z2^2 + 4*z1^4 + 32*z3^2 + 4*z2^4 + 32*z4^2 + 4*z3^4 + 4*z4^4 + x1^2*x2^2*y1^2 + x1^2*x2^2*y2^2 + x1^2*x3^2*y1^2 + 2*x1^2*x2^2*y3^2 + 2*x1^2*x3^2*y2^2 + x1^2*x4^2*y1^2 + 2*x2^2*x3^2*y1^2 + 2*x1^2*x2^2*y4^2 + x1^2*x3^2*y3^2 + 2*x1^2*x4^2*y2^2 + x2^2*x3^2*y2^2 + 2*x2^2*x4^2*y1^2 + 2*x1^2*x3^2*y4^2 + 2*x1^2*x4^2*y3^2 + x2^2*x3^2*y3^2 + x2^2*x4^2*y2^2 + 2*x3^2*x4^2*y1^2 + x1^2*x4^2*y4^2 + 2*x2^2*x3^2*y4^2 + 2*x2^2*x4^2*y3^2 + 2*x3^2*x4^2*y2^2 + x2^2*x4^2*y4^2 + x3^2*x4^2*y3^2 + x3^2*x4^2*y4^2 + x1^2*x2^2*z1^2 + x1^2*y1^2*y2^2 + x1^2*x2^2*z2^2 + x1^2*x3^2*z1^2 + x1^2*y1^2*y3^2 + x2^2*y1^2*y2^2 + 2*x1^2*x2^2*z3^2 + 2*x1^2*x3^2*z2^2 + x1^2*x4^2*z1^2 + x1^2*y1^2*y4^2 + 2*x1^2*y2^2*y3^2 + 2*x2^2*x3^2*z1^2 + 2*x2^2*y1^2*y3^2 + 2*x3^2*y1^2*y2^2 + 2*x1^2*x2^2*z4^2 + x1^2*x3^2*z3^2 + 2*x1^2*x4^2*z2^2 + 2*x1^2*y2^2*y4^2 + x2^2*x3^2*z2^2 + 2*x2^2*x4^2*z1^2 + 2*x2^2*y1^2*y4^2 + x2^2*y2^2*y3^2 + x3^2*y1^2*y3^2 + 2*x4^2*y1^2*y2^2 + 2*x1^2*x3^2*z4^2 + 2*x1^2*x4^2*z3^2 + 2*x1^2*y3^2*y4^2 + x2^2*x3^2*z3^2 + x2^2*x4^2*z2^2 + x2^2*y2^2*y4^2 + 2*x3^2*x4^2*z1^2 + 2*x3^2*y1^2*y4^2 + x3^2*y2^2*y3^2 + 2*x4^2*y1^2*y3^2 + x1^2*x4^2*z4^2 + 2*x2^2*x3^2*z4^2 + 2*x2^2*x4^2*z3^2 + 2*x2^2*y3^2*y4^2 + 2*x3^2*x4^2*z2^2 + 2*x3^2*y2^2*y4^2 + x4^2*y1^2*y4^2 + 2*x4^2*y2^2*y3^2 + x2^2*x4^2*z4^2 + x3^2*x4^2*z3^2 + x3^2*y3^2*y4^2 + x4^2*y2^2*y4^2 + x3^2*x4^2*z4^2 + x4^2*y3^2*y4^2 + 2*x1^2*y1^2*z2^2 + 2*x1^2*y2^2*z1^2 + 2*x2^2*y1^2*z1^2 + 2*x1^2*y1^2*z3^2 + 2*x1^2*y2^2*z2^2 + 2*x1^2*y3^2*z1^2 + 2*x2^2*y1^2*z2^2 + 2*x2^2*y2^2*z1^2 + 2*x3^2*y1^2*z1^2 + 2*x1^2*y1^2*z4^2 + 2*x1^2*y2^2*z3^2 + 2*x1^2*y3^2*z2^2 + 2*x1^2*y4^2*z1^2 + 2*x2^2*y1^2*z3^2 + 2*x2^2*y3^2*z1^2 + 2*x3^2*y1^2*z2^2 + 2*x3^2*y2^2*z1^2 + 2*x4^2*y1^2*z1^2 + 2*x1^2*y2^2*z4^2 + 2*x1^2*y3^2*z3^2 + 2*x1^2*y4^2*z2^2 + 2*x2^2*y1^2*z4^2 + 2*x2^2*y2^2*z3^2 + 2*x2^2*y3^2*z2^2 + 2*x2^2*y4^2*z1^2 + 2*x3^2*y1^2*z3^2 + 2*x3^2*y2^2*z2^2 + 2*x3^2*y3^2*z1^2 + 2*x4^2*y1^2*z2^2 + 2*x4^2*y2^2*z1^2 + 2*x1^2*y3^2*z4^2 + 2*x1^2*y4^2*z3^2 + 2*x2^2*y2^2*z4^2 + 2*x2^2*y3^2*z3^2 + 2*x2^2*y4^2*z2^2 + 2*x3^2*y1^2*z4^2 + 2*x3^2*y2^2*z3^2 + 2*x3^2*y3^2*z2^2 + 2*x3^2*y4^2*z1^2 + 2*x4^2*y1^2*z3^2 + 2*x4^2*y2^2*z2^2 + 2*x4^2*y3^2*z1^2 + 2*x1^2*y4^2*z4^2 + 2*x2^2*y3^2*z4^2 + 2*x2^2*y4^2*z3^2 + 2*x3^2*y2^2*z4^2 + 2*x3^2*y4^2*z2^2 + 2*x4^2*y1^2*z4^2 + 2*x4^2*y2^2*z3^2 + 2*x4^2*y3^2*z2^2 + 2*x4^2*y4^2*z1^2 + 2*x2^2*y4^2*z4^2 + 2*x3^2*y3^2*z4^2 + 2*x3^2*y4^2*z3^2 + 2*x4^2*y2^2*z4^2 + 2*x4^2*y3^2*z3^2 + 2*x4^2*y4^2*z2^2 + 2*x3^2*y4^2*z4^2 + 2*x4^2*y3^2*z4^2 + 2*x4^2*y4^2*z3^2 + x1^2*z1^2*z2^2 + y1^2*y2^2*z1^2 + x1^2*z1^2*z3^2 + x2^2*z1^2*z2^2 + y1^2*y2^2*z2^2 + y1^2*y3^2*z1^2 + x1^2*z1^2*z4^2 + 2*x1^2*z2^2*z3^2 + 2*x2^2*z1^2*z3^2 + 2*x3^2*z1^2*z2^2 + 2*y1^2*y2^2*z3^2 + 2*y1^2*y3^2*z2^2 + y1^2*y4^2*z1^2 + 2*y2^2*y3^2*z1^2 + 2*x1^2*z2^2*z4^2 + 2*x2^2*z1^2*z4^2 + x2^2*z2^2*z3^2 + x3^2*z1^2*z3^2 + 2*x4^2*z1^2*z2^2 + 2*y1^2*y2^2*z4^2 + y1^2*y3^2*z3^2 + 2*y1^2*y4^2*z2^2 + y2^2*y3^2*z2^2 + 2*y2^2*y4^2*z1^2 + 2*x1^2*z3^2*z4^2 + x2^2*z2^2*z4^2 + 2*x3^2*z1^2*z4^2 + x3^2*z2^2*z3^2 + 2*x4^2*z1^2*z3^2 + 2*y1^2*y3^2*z4^2 + 2*y1^2*y4^2*z3^2 + y2^2*y3^2*z3^2 + y2^2*y4^2*z2^2 + 2*y3^2*y4^2*z1^2 + 2*x2^2*z3^2*z4^2 + 2*x3^2*z2^2*z4^2 + x4^2*z1^2*z4^2 + 2*x4^2*z2^2*z3^2 + y1^2*y4^2*z4^2 + 2*y2^2*y3^2*z4^2 + 2*y2^2*y4^2*z3^2 + 2*y3^2*y4^2*z2^2 + x3^2*z3^2*z4^2 + x4^2*z2^2*z4^2 + y2^2*y4^2*z4^2 + y3^2*y4^2*z3^2 + x4^2*z3^2*z4^2 + y3^2*y4^2*z4^2 + y1^2*z1^2*z2^2 + y1^2*z1^2*z3^2 + y2^2*z1^2*z2^2 + y1^2*z1^2*z4^2 + 2*y1^2*z2^2*z3^2 + 2*y2^2*z1^2*z3^2 + 2*y3^2*z1^2*z2^2 + 2*y1^2*z2^2*z4^2 + 2*y2^2*z1^2*z4^2 + y2^2*z2^2*z3^2 + y3^2*z1^2*z3^2 + 2*y4^2*z1^2*z2^2 + 2*y1^2*z3^2*z4^2 + y2^2*z2^2*z4^2 + 2*y3^2*z1^2*z4^2 + y3^2*z2^2*z3^2 + 2*y4^2*z1^2*z3^2 + 2*y2^2*z3^2*z4^2 + 2*y3^2*z2^2*z4^2 + y4^2*z1^2*z4^2 + 2*y4^2*z2^2*z3^2 + y3^2*z3^2*z4^2 + y4^2*z2^2*z4^2 + y4^2*z3^2*z4^2 - 8*x1*x2*y1*y2 - 8*x1*x3*y1*y3 - 8*x1*x4*y1*y4 - 8*x2*x3*y2*y3 - 8*x2*x4*y2*y4 - 8*x3*x4*y3*y4 - 8*x1*x2*z1*z2 - 8*x1*x3*z1*z3 - 8*x1*x4*z1*z4 - 8*x2*x3*z2*z3 - 8*x2*x4*z2*z4 - 8*x3*x4*z3*z4 - 8*y1*y2*z1*z2 - 8*y1*y3*z1*z3 - 8*y1*y4*z1*z4 - 8*y2*y3*z2*z3 - 8*y2*y4*z2*z4 - 8*y3*y4*z3*z4 - 2*x1*x2*y1*y2^3 - 2*x1*x2*y1^3*y2 - 2*x1*x2^3*y1*y2 - 2*x1^3*x2*y1*y2 - 2*x1*x3*y1*y3^3 - 2*x1*x3*y1^3*y3 - 2*x1*x3^3*y1*y3 - 2*x1^3*x3*y1*y3 - 2*x1*x4*y1*y4^3 - 2*x1*x4*y1^3*y4 - 2*x1*x4^3*y1*y4 - 2*x2*x3*y2*y3^3 - 2*x2*x3*y2^3*y3 - 2*x2*x3^3*y2*y3 - 2*x1^3*x4*y1*y4 - 2*x2^3*x3*y2*y3 - 2*x2*x4*y2*y4^3 - 2*x2*x4*y2^3*y4 - 2*x2*x4^3*y2*y4 - 2*x2^3*x4*y2*y4 - 2*x3*x4*y3*y4^3 - 2*x3*x4*y3^3*y4 - 2*x3*x4^3*y3*y4 - 2*x3^3*x4*y3*y4 - 2*x1*x2*z1*z2^3 - 2*x1*x2*z1^3*z2 - 2*x1*x2^3*z1*z2 - 2*x1^3*x2*z1*z2 - 2*x1*x3*z1*z3^3 - 2*x1*x3*z1^3*z3 - 2*x1*x3^3*z1*z3 - 2*x1^3*x3*z1*z3 - 2*x1*x4*z1*z4^3 - 2*x1*x4*z1^3*z4 - 2*x1*x4^3*z1*z4 - 2*x2*x3*z2*z3^3 - 2*x2*x3*z2^3*z3 - 2*x2*x3^3*z2*z3 - 2*x1^3*x4*z1*z4 - 2*x2^3*x3*z2*z3 - 2*x2*x4*z2*z4^3 - 2*x2*x4*z2^3*z4 - 2*x2*x4^3*z2*z4 - 2*x2^3*x4*z2*z4 - 2*x3*x4*z3*z4^3 - 2*x3*x4*z3^3*z4 - 2*x3*x4^3*z3*z4 - 2*x3^3*x4*z3*z4 - 2*y1*y2*z1*z2^3 - 2*y1*y2*z1^3*z2 - 2*y1*y2^3*z1*z2 - 2*y1^3*y2*z1*z2 - 2*y1*y3*z1*z3^3 - 2*y1*y3*z1^3*z3 - 2*y1*y3^3*z1*z3 - 2*y1^3*y3*z1*z3 - 2*y1*y4*z1*z4^3 - 2*y1*y4*z1^3*z4 - 2*y1*y4^3*z1*z4 - 2*y2*y3*z2*z3^3 - 2*y2*y3*z2^3*z3 - 2*y2*y3^3*z2*z3 - 2*y1^3*y4*z1*z4 - 2*y2^3*y3*z2*z3 - 2*y2*y4*z2*z4^3 - 2*y2*y4*z2^3*z4 - 2*y2*y4^3*z2*z4 - 2*y2^3*y4*z2*z4 - 2*y3*y4*z3*z4^3 - 2*y3*y4*z3^3*z4 - 2*y3*y4^3*z3*z4 - 2*y3^3*y4*z3*z4 - 2*x1*x2*x3^2*y1*y2 - 2*x1*x2*x4^2*y1*y2 - 2*x1*x2^2*x3*y1*y3 - 2*x1^2*x2*x3*y2*y3 - 2*x1*x3*x4^2*y1*y3 - 2*x1*x2^2*x4*y1*y4 - 2*x1*x3^2*x4*y1*y4 - 2*x1^2*x2*x4*y2*y4 - 2*x2*x3*x4^2*y2*y3 - 2*x2*x3^2*x4*y2*y4 - 2*x1^2*x3*x4*y3*y4 - 2*x2^2*x3*x4*y3*y4 - 2*x1*x2*y1*y2*y3^2 - 2*x1*x2*y1*y2*y4^2 - 2*x1*x3*y1*y2^2*y3 - 2*x2*x3*y1^2*y2*y3 - 2*x1*x3*y1*y3*y4^2 - 2*x1*x4*y1*y2^2*y4 - 2*x1*x4*y1*y3^2*y4 - 2*x2*x4*y1^2*y2*y4 - 2*x2*x3*y2*y3*y4^2 - 2*x2*x4*y2*y3^2*y4 - 2*x3*x4*y1^2*y3*y4 - 2*x3*x4*y2^2*y3*y4 - 2*x1*x2*y1*y2*z1^2 - 2*x1*x2*y1*y2*z2^2 - 2*x1*x2*x3^2*z1*z2 - 2*x1*x3*y1*y3*z1^2 - 2*x1*x2*x4^2*z1*z2 - 2*x1*x2^2*x3*z1*z3 - 2*x1*x3*y1*y3*z3^2 - 2*x1*x4*y1*y4*z1^2 - 2*x1^2*x2*x3*z2*z3 - 2*x1*x3*x4^2*z1*z3 - 2*x1*x2^2*x4*z1*z4 - 2*x2*x3*y2*y3*z2^2 - 2*x1*x3^2*x4*z1*z4 - 2*x2*x3*y2*y3*z3^2 - 2*x1^2*x2*x4*z2*z4 - 2*x1*x4*y1*y4*z4^2 - 2*x2*x3*x4^2*z2*z3 - 2*x2*x4*y2*y4*z2^2 - 2*x2*x3^2*x4*z2*z4 - 2*x1^2*x3*x4*z3*z4 - 2*x2*x4*y2*y4*z4^2 - 2*x2^2*x3*x4*z3*z4 - 2*x3*x4*y3*y4*z3^2 - 2*x3*x4*y3*y4*z4^2 - 2*x1*x2*y1^2*z1*z2 - 2*x1*x2*y2^2*z1*z2 - 2*x1*x3*y1^2*z1*z3 - 2*x1*x3*y3^2*z1*z3 - 2*x1*x4*y1^2*z1*z4 - 2*x2*x3*y2^2*z2*z3 - 2*x2*x3*y3^2*z2*z3 - 2*x1*x4*y4^2*z1*z4 - 2*x2*x4*y2^2*z2*z4 - 2*x2*x4*y4^2*z2*z4 - 2*x3*x4*y3^2*z3*z4 - 2*x3*x4*y4^2*z3*z4 - 2*x1^2*y1*y2*z1*z2 - 2*x2^2*y1*y2*z1*z2 - 2*x1*x2*z1*z2*z3^2 - 2*x1^2*y1*y3*z1*z3 - 2*x1*x2*z1*z2*z4^2 - 2*x1*x3*z1*z2^2*z3 - 2*x2*x3*z1^2*z2*z3 - 2*x1^2*y1*y4*z1*z4 - 2*x3^2*y1*y3*z1*z3 - 2*x1*x3*z1*z3*z4^2 - 2*x1*x4*z1*z2^2*z4 - 2*x2^2*y2*y3*z2*z3 - 2*x1*x4*z1*z3^2*z4 - 2*x2*x4*z1^2*z2*z4 - 2*x3^2*y2*y3*z2*z3 - 2*x2*x3*z2*z3*z4^2 - 2*x2^2*y2*y4*z2*z4 - 2*x4^2*y1*y4*z1*z4 - 2*x2*x4*z2*z3^2*z4 - 2*x3*x4*z1^2*z3*z4 - 2*x3*x4*z2^2*z3*z4 - 2*x4^2*y2*y4*z2*z4 - 2*x3^2*y3*y4*z3*z4 - 2*x4^2*y3*y4*z3*z4 - 2*y1*y2*y3^2*z1*z2 - 2*y1*y2*y4^2*z1*z2 - 2*y1*y2^2*y3*z1*z3 - 2*y1^2*y2*y3*z2*z3 - 2*y1*y3*y4^2*z1*z3 - 2*y1*y2^2*y4*z1*z4 - 2*y1*y3^2*y4*z1*z4 - 2*y1^2*y2*y4*z2*z4 - 2*y2*y3*y4^2*z2*z3 - 2*y2*y3^2*y4*z2*z4 - 2*y1^2*y3*y4*z3*z4 - 2*y2^2*y3*y4*z3*z4 - 2*y1*y2*z1*z2*z3^2 - 2*y1*y2*z1*z2*z4^2 - 2*y1*y3*z1*z2^2*z3 - 2*y2*y3*z1^2*z2*z3 - 2*y1*y3*z1*z3*z4^2 - 2*y1*y4*z1*z2^2*z4 - 2*y1*y4*z1*z3^2*z4 - 2*y2*y4*z1^2*z2*z4 - 2*y2*y3*z2*z3*z4^2 - 2*y2*y4*z2*z3^2*z4 - 2*y3*y4*z1^2*z3*z4 - 2*y3*y4*z2^2*z3*z4 - 2*x1*x2*y1*y3*z2*z3 - 2*x1*x2*y2*y3*z1*z3 - 2*x1*x3*y1*y2*z2*z3 - 2*x1*x3*y2*y3*z1*z2 - 2*x2*x3*y1*y2*z1*z3 - 2*x2*x3*y1*y3*z1*z2 - 2*x1*x2*y1*y4*z2*z4 - 2*x1*x2*y2*y4*z1*z4 - 2*x1*x4*y1*y2*z2*z4 - 2*x1*x4*y2*y4*z1*z2 - 2*x2*x4*y1*y2*z1*z4 - 2*x2*x4*y1*y4*z1*z2 - 2*x1*x3*y1*y4*z3*z4 - 2*x1*x3*y3*y4*z1*z4 - 2*x1*x4*y1*y3*z3*z4 - 2*x1*x4*y3*y4*z1*z3 - 2*x3*x4*y1*y3*z1*z4 - 2*x3*x4*y1*y4*z1*z3 - 2*x2*x3*y2*y4*z3*z4 - 2*x2*x3*y3*y4*z2*z4 - 2*x2*x4*y2*y3*z3*z4 - 2*x2*x4*y3*y4*z2*z3 - 2*x3*x4*y2*y3*z2*z4 - 2*x3*x4*y2*y4*z2*z3 + 64),...
        (4*(4*y1*z1 + 4*y2*z2 + 4*y3*z3 + 4*y4*z4 + y1*z1^3 + y1^3*z1 + y2*z2^3 + y2^3*z2 + y3*z3^3 + y3^3*z3 + y4*z4^3 + y4^3*z4 + x1^2*y1*z1 + x2^2*y2*z2 + x3^2*y3*z3 + x4^2*y4*z4 + y1*y2^2*z1 + y1*y3^2*z1 + y1^2*y2*z2 + y1*y4^2*z1 + y2*y3^2*z2 + y1^2*y3*z3 + y2*y4^2*z2 + y2^2*y3*z3 + y1^2*y4*z4 + y3*y4^2*z3 + y2^2*y4*z4 + y3^2*y4*z4 + y1*z1*z2^2 + y1*z1*z3^2 + y2*z1^2*z2 + y1*z1*z4^2 + y2*z2*z3^2 + y3*z1^2*z3 + y2*z2*z4^2 + y3*z2^2*z3 + y4*z1^2*z4 + y3*z3*z4^2 + y4*z2^2*z4 + y4*z3^2*z4 + x1*x2*y1*z2 + x1*x2*y2*z1 + x1*x3*y1*z3 + x1*x3*y3*z1 + x1*x4*y1*z4 + x1*x4*y4*z1 + x2*x3*y2*z3 + x2*x3*y3*z2 + x2*x4*y2*z4 + x2*x4*y4*z2 + x3*x4*y3*z4 + x3*x4*y4*z3))/(8*x1^2*x2^2 + 8*x1^2*x3^2 + 8*x1^2*x4^2 + 8*x2^2*x3^2 + 8*x2^2*x4^2 + 8*x3^2*x4^2 + 8*x1^2*y1^2 + 12*x1^2*y2^2 + 12*x2^2*y1^2 + 12*x1^2*y3^2 + 8*x2^2*y2^2 + 12*x3^2*y1^2 + x1^2*y2^4 + 12*x1^2*y4^2 + x2^2*y1^4 + 12*x2^2*y3^2 + x1^4*y2^2 + 12*x3^2*y2^2 + x2^4*y1^2 + 12*x4^2*y1^2 + x1^2*y3^4 + 12*x2^2*y4^2 + x1^4*y3^2 + x3^2*y1^4 + 8*x3^2*y3^2 + 12*x4^2*y2^2 + x3^4*y1^2 + x1^2*y4^4 + x2^2*y3^4 + x1^4*y4^2 + x3^2*y2^4 + 12*x3^2*y4^2 + x2^4*y3^2 + x4^2*y1^4 + 12*x4^2*y3^2 + x3^4*y2^2 + x4^4*y1^2 + x2^2*y4^4 + x2^4*y4^2 + x4^2*y2^4 + 8*x4^2*y4^2 + x4^4*y2^2 + x3^2*y4^4 + x4^2*y3^4 + x3^4*y4^2 + x4^4*y3^2 + 8*x1^2*z1^2 + 12*x1^2*z2^2 + 12*x2^2*z1^2 + 8*y1^2*y2^2 + 12*x1^2*z3^2 + 8*x2^2*z2^2 + 12*x3^2*z1^2 + 8*y1^2*y3^2 + x1^2*z2^4 + 12*x1^2*z4^2 + x2^2*z1^4 + 12*x2^2*z3^2 + x1^4*z2^2 + 12*x3^2*z2^2 + x2^4*z1^2 + 12*x4^2*z1^2 + 8*y1^2*y4^2 + 8*y2^2*y3^2 + x1^2*z3^4 + 12*x2^2*z4^2 + x1^4*z3^2 + x3^2*z1^4 + 8*x3^2*z3^2 + 12*x4^2*z2^2 + x3^4*z1^2 + 8*y2^2*y4^2 + x1^2*z4^4 + x2^2*z3^4 + x1^4*z4^2 + x3^2*z2^4 + 12*x3^2*z4^2 + x2^4*z3^2 + x4^2*z1^4 + 12*x4^2*z3^2 + x3^4*z2^2 + x4^4*z1^2 + 8*y3^2*y4^2 + x2^2*z4^4 + x2^4*z4^2 + x4^2*z2^4 + 8*x4^2*z4^2 + x4^4*z2^2 + x3^2*z4^4 + x4^2*z3^4 + x3^4*z4^2 + x4^4*z3^2 + 8*y1^2*z1^2 + 12*y1^2*z2^2 + 12*y2^2*z1^2 + 12*y1^2*z3^2 + 8*y2^2*z2^2 + 12*y3^2*z1^2 + y1^2*z2^4 + 12*y1^2*z4^2 + y2^2*z1^4 + 12*y2^2*z3^2 + y1^4*z2^2 + 12*y3^2*z2^2 + y2^4*z1^2 + 12*y4^2*z1^2 + y1^2*z3^4 + 12*y2^2*z4^2 + y1^4*z3^2 + y3^2*z1^4 + 8*y3^2*z3^2 + 12*y4^2*z2^2 + y3^4*z1^2 + y1^2*z4^4 + y2^2*z3^4 + y1^4*z4^2 + y3^2*z2^4 + 12*y3^2*z4^2 + y2^4*z3^2 + y4^2*z1^4 + 12*y4^2*z3^2 + y3^4*z2^2 + y4^4*z1^2 + y2^2*z4^4 + y2^4*z4^2 + y4^2*z2^4 + 8*y4^2*z4^2 + y4^4*z2^2 + y3^2*z4^4 + y4^2*z3^4 + y3^4*z4^2 + y4^4*z3^2 + 8*z1^2*z2^2 + 8*z1^2*z3^2 + 8*z1^2*z4^2 + 8*z2^2*z3^2 + 8*z2^2*z4^2 + 8*z3^2*z4^2 + 32*x1^2 + 32*x2^2 + 4*x1^4 + 32*x3^2 + 4*x2^4 + 32*x4^2 + 4*x3^4 + 4*x4^4 + 32*y1^2 + 32*y2^2 + 4*y1^4 + 32*y3^2 + 4*y2^4 + 32*y4^2 + 4*y3^4 + 4*y4^4 + 32*z1^2 + 32*z2^2 + 4*z1^4 + 32*z3^2 + 4*z2^4 + 32*z4^2 + 4*z3^4 + 4*z4^4 + x1^2*x2^2*y1^2 + x1^2*x2^2*y2^2 + x1^2*x3^2*y1^2 + 2*x1^2*x2^2*y3^2 + 2*x1^2*x3^2*y2^2 + x1^2*x4^2*y1^2 + 2*x2^2*x3^2*y1^2 + 2*x1^2*x2^2*y4^2 + x1^2*x3^2*y3^2 + 2*x1^2*x4^2*y2^2 + x2^2*x3^2*y2^2 + 2*x2^2*x4^2*y1^2 + 2*x1^2*x3^2*y4^2 + 2*x1^2*x4^2*y3^2 + x2^2*x3^2*y3^2 + x2^2*x4^2*y2^2 + 2*x3^2*x4^2*y1^2 + x1^2*x4^2*y4^2 + 2*x2^2*x3^2*y4^2 + 2*x2^2*x4^2*y3^2 + 2*x3^2*x4^2*y2^2 + x2^2*x4^2*y4^2 + x3^2*x4^2*y3^2 + x3^2*x4^2*y4^2 + x1^2*x2^2*z1^2 + x1^2*y1^2*y2^2 + x1^2*x2^2*z2^2 + x1^2*x3^2*z1^2 + x1^2*y1^2*y3^2 + x2^2*y1^2*y2^2 + 2*x1^2*x2^2*z3^2 + 2*x1^2*x3^2*z2^2 + x1^2*x4^2*z1^2 + x1^2*y1^2*y4^2 + 2*x1^2*y2^2*y3^2 + 2*x2^2*x3^2*z1^2 + 2*x2^2*y1^2*y3^2 + 2*x3^2*y1^2*y2^2 + 2*x1^2*x2^2*z4^2 + x1^2*x3^2*z3^2 + 2*x1^2*x4^2*z2^2 + 2*x1^2*y2^2*y4^2 + x2^2*x3^2*z2^2 + 2*x2^2*x4^2*z1^2 + 2*x2^2*y1^2*y4^2 + x2^2*y2^2*y3^2 + x3^2*y1^2*y3^2 + 2*x4^2*y1^2*y2^2 + 2*x1^2*x3^2*z4^2 + 2*x1^2*x4^2*z3^2 + 2*x1^2*y3^2*y4^2 + x2^2*x3^2*z3^2 + x2^2*x4^2*z2^2 + x2^2*y2^2*y4^2 + 2*x3^2*x4^2*z1^2 + 2*x3^2*y1^2*y4^2 + x3^2*y2^2*y3^2 + 2*x4^2*y1^2*y3^2 + x1^2*x4^2*z4^2 + 2*x2^2*x3^2*z4^2 + 2*x2^2*x4^2*z3^2 + 2*x2^2*y3^2*y4^2 + 2*x3^2*x4^2*z2^2 + 2*x3^2*y2^2*y4^2 + x4^2*y1^2*y4^2 + 2*x4^2*y2^2*y3^2 + x2^2*x4^2*z4^2 + x3^2*x4^2*z3^2 + x3^2*y3^2*y4^2 + x4^2*y2^2*y4^2 + x3^2*x4^2*z4^2 + x4^2*y3^2*y4^2 + 2*x1^2*y1^2*z2^2 + 2*x1^2*y2^2*z1^2 + 2*x2^2*y1^2*z1^2 + 2*x1^2*y1^2*z3^2 + 2*x1^2*y2^2*z2^2 + 2*x1^2*y3^2*z1^2 + 2*x2^2*y1^2*z2^2 + 2*x2^2*y2^2*z1^2 + 2*x3^2*y1^2*z1^2 + 2*x1^2*y1^2*z4^2 + 2*x1^2*y2^2*z3^2 + 2*x1^2*y3^2*z2^2 + 2*x1^2*y4^2*z1^2 + 2*x2^2*y1^2*z3^2 + 2*x2^2*y3^2*z1^2 + 2*x3^2*y1^2*z2^2 + 2*x3^2*y2^2*z1^2 + 2*x4^2*y1^2*z1^2 + 2*x1^2*y2^2*z4^2 + 2*x1^2*y3^2*z3^2 + 2*x1^2*y4^2*z2^2 + 2*x2^2*y1^2*z4^2 + 2*x2^2*y2^2*z3^2 + 2*x2^2*y3^2*z2^2 + 2*x2^2*y4^2*z1^2 + 2*x3^2*y1^2*z3^2 + 2*x3^2*y2^2*z2^2 + 2*x3^2*y3^2*z1^2 + 2*x4^2*y1^2*z2^2 + 2*x4^2*y2^2*z1^2 + 2*x1^2*y3^2*z4^2 + 2*x1^2*y4^2*z3^2 + 2*x2^2*y2^2*z4^2 + 2*x2^2*y3^2*z3^2 + 2*x2^2*y4^2*z2^2 + 2*x3^2*y1^2*z4^2 + 2*x3^2*y2^2*z3^2 + 2*x3^2*y3^2*z2^2 + 2*x3^2*y4^2*z1^2 + 2*x4^2*y1^2*z3^2 + 2*x4^2*y2^2*z2^2 + 2*x4^2*y3^2*z1^2 + 2*x1^2*y4^2*z4^2 + 2*x2^2*y3^2*z4^2 + 2*x2^2*y4^2*z3^2 + 2*x3^2*y2^2*z4^2 + 2*x3^2*y4^2*z2^2 + 2*x4^2*y1^2*z4^2 + 2*x4^2*y2^2*z3^2 + 2*x4^2*y3^2*z2^2 + 2*x4^2*y4^2*z1^2 + 2*x2^2*y4^2*z4^2 + 2*x3^2*y3^2*z4^2 + 2*x3^2*y4^2*z3^2 + 2*x4^2*y2^2*z4^2 + 2*x4^2*y3^2*z3^2 + 2*x4^2*y4^2*z2^2 + 2*x3^2*y4^2*z4^2 + 2*x4^2*y3^2*z4^2 + 2*x4^2*y4^2*z3^2 + x1^2*z1^2*z2^2 + y1^2*y2^2*z1^2 + x1^2*z1^2*z3^2 + x2^2*z1^2*z2^2 + y1^2*y2^2*z2^2 + y1^2*y3^2*z1^2 + x1^2*z1^2*z4^2 + 2*x1^2*z2^2*z3^2 + 2*x2^2*z1^2*z3^2 + 2*x3^2*z1^2*z2^2 + 2*y1^2*y2^2*z3^2 + 2*y1^2*y3^2*z2^2 + y1^2*y4^2*z1^2 + 2*y2^2*y3^2*z1^2 + 2*x1^2*z2^2*z4^2 + 2*x2^2*z1^2*z4^2 + x2^2*z2^2*z3^2 + x3^2*z1^2*z3^2 + 2*x4^2*z1^2*z2^2 + 2*y1^2*y2^2*z4^2 + y1^2*y3^2*z3^2 + 2*y1^2*y4^2*z2^2 + y2^2*y3^2*z2^2 + 2*y2^2*y4^2*z1^2 + 2*x1^2*z3^2*z4^2 + x2^2*z2^2*z4^2 + 2*x3^2*z1^2*z4^2 + x3^2*z2^2*z3^2 + 2*x4^2*z1^2*z3^2 + 2*y1^2*y3^2*z4^2 + 2*y1^2*y4^2*z3^2 + y2^2*y3^2*z3^2 + y2^2*y4^2*z2^2 + 2*y3^2*y4^2*z1^2 + 2*x2^2*z3^2*z4^2 + 2*x3^2*z2^2*z4^2 + x4^2*z1^2*z4^2 + 2*x4^2*z2^2*z3^2 + y1^2*y4^2*z4^2 + 2*y2^2*y3^2*z4^2 + 2*y2^2*y4^2*z3^2 + 2*y3^2*y4^2*z2^2 + x3^2*z3^2*z4^2 + x4^2*z2^2*z4^2 + y2^2*y4^2*z4^2 + y3^2*y4^2*z3^2 + x4^2*z3^2*z4^2 + y3^2*y4^2*z4^2 + y1^2*z1^2*z2^2 + y1^2*z1^2*z3^2 + y2^2*z1^2*z2^2 + y1^2*z1^2*z4^2 + 2*y1^2*z2^2*z3^2 + 2*y2^2*z1^2*z3^2 + 2*y3^2*z1^2*z2^2 + 2*y1^2*z2^2*z4^2 + 2*y2^2*z1^2*z4^2 + y2^2*z2^2*z3^2 + y3^2*z1^2*z3^2 + 2*y4^2*z1^2*z2^2 + 2*y1^2*z3^2*z4^2 + y2^2*z2^2*z4^2 + 2*y3^2*z1^2*z4^2 + y3^2*z2^2*z3^2 + 2*y4^2*z1^2*z3^2 + 2*y2^2*z3^2*z4^2 + 2*y3^2*z2^2*z4^2 + y4^2*z1^2*z4^2 + 2*y4^2*z2^2*z3^2 + y3^2*z3^2*z4^2 + y4^2*z2^2*z4^2 + y4^2*z3^2*z4^2 - 8*x1*x2*y1*y2 - 8*x1*x3*y1*y3 - 8*x1*x4*y1*y4 - 8*x2*x3*y2*y3 - 8*x2*x4*y2*y4 - 8*x3*x4*y3*y4 - 8*x1*x2*z1*z2 - 8*x1*x3*z1*z3 - 8*x1*x4*z1*z4 - 8*x2*x3*z2*z3 - 8*x2*x4*z2*z4 - 8*x3*x4*z3*z4 - 8*y1*y2*z1*z2 - 8*y1*y3*z1*z3 - 8*y1*y4*z1*z4 - 8*y2*y3*z2*z3 - 8*y2*y4*z2*z4 - 8*y3*y4*z3*z4 - 2*x1*x2*y1*y2^3 - 2*x1*x2*y1^3*y2 - 2*x1*x2^3*y1*y2 - 2*x1^3*x2*y1*y2 - 2*x1*x3*y1*y3^3 - 2*x1*x3*y1^3*y3 - 2*x1*x3^3*y1*y3 - 2*x1^3*x3*y1*y3 - 2*x1*x4*y1*y4^3 - 2*x1*x4*y1^3*y4 - 2*x1*x4^3*y1*y4 - 2*x2*x3*y2*y3^3 - 2*x2*x3*y2^3*y3 - 2*x2*x3^3*y2*y3 - 2*x1^3*x4*y1*y4 - 2*x2^3*x3*y2*y3 - 2*x2*x4*y2*y4^3 - 2*x2*x4*y2^3*y4 - 2*x2*x4^3*y2*y4 - 2*x2^3*x4*y2*y4 - 2*x3*x4*y3*y4^3 - 2*x3*x4*y3^3*y4 - 2*x3*x4^3*y3*y4 - 2*x3^3*x4*y3*y4 - 2*x1*x2*z1*z2^3 - 2*x1*x2*z1^3*z2 - 2*x1*x2^3*z1*z2 - 2*x1^3*x2*z1*z2 - 2*x1*x3*z1*z3^3 - 2*x1*x3*z1^3*z3 - 2*x1*x3^3*z1*z3 - 2*x1^3*x3*z1*z3 - 2*x1*x4*z1*z4^3 - 2*x1*x4*z1^3*z4 - 2*x1*x4^3*z1*z4 - 2*x2*x3*z2*z3^3 - 2*x2*x3*z2^3*z3 - 2*x2*x3^3*z2*z3 - 2*x1^3*x4*z1*z4 - 2*x2^3*x3*z2*z3 - 2*x2*x4*z2*z4^3 - 2*x2*x4*z2^3*z4 - 2*x2*x4^3*z2*z4 - 2*x2^3*x4*z2*z4 - 2*x3*x4*z3*z4^3 - 2*x3*x4*z3^3*z4 - 2*x3*x4^3*z3*z4 - 2*x3^3*x4*z3*z4 - 2*y1*y2*z1*z2^3 - 2*y1*y2*z1^3*z2 - 2*y1*y2^3*z1*z2 - 2*y1^3*y2*z1*z2 - 2*y1*y3*z1*z3^3 - 2*y1*y3*z1^3*z3 - 2*y1*y3^3*z1*z3 - 2*y1^3*y3*z1*z3 - 2*y1*y4*z1*z4^3 - 2*y1*y4*z1^3*z4 - 2*y1*y4^3*z1*z4 - 2*y2*y3*z2*z3^3 - 2*y2*y3*z2^3*z3 - 2*y2*y3^3*z2*z3 - 2*y1^3*y4*z1*z4 - 2*y2^3*y3*z2*z3 - 2*y2*y4*z2*z4^3 - 2*y2*y4*z2^3*z4 - 2*y2*y4^3*z2*z4 - 2*y2^3*y4*z2*z4 - 2*y3*y4*z3*z4^3 - 2*y3*y4*z3^3*z4 - 2*y3*y4^3*z3*z4 - 2*y3^3*y4*z3*z4 - 2*x1*x2*x3^2*y1*y2 - 2*x1*x2*x4^2*y1*y2 - 2*x1*x2^2*x3*y1*y3 - 2*x1^2*x2*x3*y2*y3 - 2*x1*x3*x4^2*y1*y3 - 2*x1*x2^2*x4*y1*y4 - 2*x1*x3^2*x4*y1*y4 - 2*x1^2*x2*x4*y2*y4 - 2*x2*x3*x4^2*y2*y3 - 2*x2*x3^2*x4*y2*y4 - 2*x1^2*x3*x4*y3*y4 - 2*x2^2*x3*x4*y3*y4 - 2*x1*x2*y1*y2*y3^2 - 2*x1*x2*y1*y2*y4^2 - 2*x1*x3*y1*y2^2*y3 - 2*x2*x3*y1^2*y2*y3 - 2*x1*x3*y1*y3*y4^2 - 2*x1*x4*y1*y2^2*y4 - 2*x1*x4*y1*y3^2*y4 - 2*x2*x4*y1^2*y2*y4 - 2*x2*x3*y2*y3*y4^2 - 2*x2*x4*y2*y3^2*y4 - 2*x3*x4*y1^2*y3*y4 - 2*x3*x4*y2^2*y3*y4 - 2*x1*x2*y1*y2*z1^2 - 2*x1*x2*y1*y2*z2^2 - 2*x1*x2*x3^2*z1*z2 - 2*x1*x3*y1*y3*z1^2 - 2*x1*x2*x4^2*z1*z2 - 2*x1*x2^2*x3*z1*z3 - 2*x1*x3*y1*y3*z3^2 - 2*x1*x4*y1*y4*z1^2 - 2*x1^2*x2*x3*z2*z3 - 2*x1*x3*x4^2*z1*z3 - 2*x1*x2^2*x4*z1*z4 - 2*x2*x3*y2*y3*z2^2 - 2*x1*x3^2*x4*z1*z4 - 2*x2*x3*y2*y3*z3^2 - 2*x1^2*x2*x4*z2*z4 - 2*x1*x4*y1*y4*z4^2 - 2*x2*x3*x4^2*z2*z3 - 2*x2*x4*y2*y4*z2^2 - 2*x2*x3^2*x4*z2*z4 - 2*x1^2*x3*x4*z3*z4 - 2*x2*x4*y2*y4*z4^2 - 2*x2^2*x3*x4*z3*z4 - 2*x3*x4*y3*y4*z3^2 - 2*x3*x4*y3*y4*z4^2 - 2*x1*x2*y1^2*z1*z2 - 2*x1*x2*y2^2*z1*z2 - 2*x1*x3*y1^2*z1*z3 - 2*x1*x3*y3^2*z1*z3 - 2*x1*x4*y1^2*z1*z4 - 2*x2*x3*y2^2*z2*z3 - 2*x2*x3*y3^2*z2*z3 - 2*x1*x4*y4^2*z1*z4 - 2*x2*x4*y2^2*z2*z4 - 2*x2*x4*y4^2*z2*z4 - 2*x3*x4*y3^2*z3*z4 - 2*x3*x4*y4^2*z3*z4 - 2*x1^2*y1*y2*z1*z2 - 2*x2^2*y1*y2*z1*z2 - 2*x1*x2*z1*z2*z3^2 - 2*x1^2*y1*y3*z1*z3 - 2*x1*x2*z1*z2*z4^2 - 2*x1*x3*z1*z2^2*z3 - 2*x2*x3*z1^2*z2*z3 - 2*x1^2*y1*y4*z1*z4 - 2*x3^2*y1*y3*z1*z3 - 2*x1*x3*z1*z3*z4^2 - 2*x1*x4*z1*z2^2*z4 - 2*x2^2*y2*y3*z2*z3 - 2*x1*x4*z1*z3^2*z4 - 2*x2*x4*z1^2*z2*z4 - 2*x3^2*y2*y3*z2*z3 - 2*x2*x3*z2*z3*z4^2 - 2*x2^2*y2*y4*z2*z4 - 2*x4^2*y1*y4*z1*z4 - 2*x2*x4*z2*z3^2*z4 - 2*x3*x4*z1^2*z3*z4 - 2*x3*x4*z2^2*z3*z4 - 2*x4^2*y2*y4*z2*z4 - 2*x3^2*y3*y4*z3*z4 - 2*x4^2*y3*y4*z3*z4 - 2*y1*y2*y3^2*z1*z2 - 2*y1*y2*y4^2*z1*z2 - 2*y1*y2^2*y3*z1*z3 - 2*y1^2*y2*y3*z2*z3 - 2*y1*y3*y4^2*z1*z3 - 2*y1*y2^2*y4*z1*z4 - 2*y1*y3^2*y4*z1*z4 - 2*y1^2*y2*y4*z2*z4 - 2*y2*y3*y4^2*z2*z3 - 2*y2*y3^2*y4*z2*z4 - 2*y1^2*y3*y4*z3*z4 - 2*y2^2*y3*y4*z3*z4 - 2*y1*y2*z1*z2*z3^2 - 2*y1*y2*z1*z2*z4^2 - 2*y1*y3*z1*z2^2*z3 - 2*y2*y3*z1^2*z2*z3 - 2*y1*y3*z1*z3*z4^2 - 2*y1*y4*z1*z2^2*z4 - 2*y1*y4*z1*z3^2*z4 - 2*y2*y4*z1^2*z2*z4 - 2*y2*y3*z2*z3*z4^2 - 2*y2*y4*z2*z3^2*z4 - 2*y3*y4*z1^2*z3*z4 - 2*y3*y4*z2^2*z3*z4 - 2*x1*x2*y1*y3*z2*z3 - 2*x1*x2*y2*y3*z1*z3 - 2*x1*x3*y1*y2*z2*z3 - 2*x1*x3*y2*y3*z1*z2 - 2*x2*x3*y1*y2*z1*z3 - 2*x2*x3*y1*y3*z1*z2 - 2*x1*x2*y1*y4*z2*z4 - 2*x1*x2*y2*y4*z1*z4 - 2*x1*x4*y1*y2*z2*z4 - 2*x1*x4*y2*y4*z1*z2 - 2*x2*x4*y1*y2*z1*z4 - 2*x2*x4*y1*y4*z1*z2 - 2*x1*x3*y1*y4*z3*z4 - 2*x1*x3*y3*y4*z1*z4 - 2*x1*x4*y1*y3*z3*z4 - 2*x1*x4*y3*y4*z1*z3 - 2*x3*x4*y1*y3*z1*z4 - 2*x3*x4*y1*y4*z1*z3 - 2*x2*x3*y2*y4*z3*z4 - 2*x2*x3*y3*y4*z2*z4 - 2*x2*x4*y2*y3*z3*z4 - 2*x2*x4*y3*y4*z2*z3 - 2*x3*x4*y2*y3*z2*z4 - 2*x3*x4*y2*y4*z2*z3 + 64),...
        (4*(x1^2*y2^2 + x2^2*y1^2 + x1^2*y3^2 + x3^2*y1^2 + x1^2*y4^2 + x2^2*y3^2 + x3^2*y2^2 + x4^2*y1^2 + x2^2*y4^2 + x4^2*y2^2 + x3^2*y4^2 + x4^2*y3^2 + x1^2*z1^2 + x1^2*z2^2 + x2^2*z1^2 + x1^2*z3^2 + x2^2*z2^2 + x3^2*z1^2 + x1^2*z4^2 + x2^2*z3^2 + x3^2*z2^2 + x4^2*z1^2 + x2^2*z4^2 + x3^2*z3^2 + x4^2*z2^2 + x3^2*z4^2 + x4^2*z3^2 + x4^2*z4^2 + y1^2*z1^2 + y1^2*z2^2 + y2^2*z1^2 + y1^2*z3^2 + y2^2*z2^2 + y3^2*z1^2 + y1^2*z4^2 + y2^2*z3^2 + y3^2*z2^2 + y4^2*z1^2 + y2^2*z4^2 + y3^2*z3^2 + y4^2*z2^2 + y3^2*z4^2 + y4^2*z3^2 + y4^2*z4^2 + 2*z1^2*z2^2 + 2*z1^2*z3^2 + 2*z1^2*z4^2 + 2*z2^2*z3^2 + 2*z2^2*z4^2 + 2*z3^2*z4^2 + 4*x1^2 + 4*x2^2 + 4*x3^2 + 4*x4^2 + 4*y1^2 + 4*y2^2 + 4*y3^2 + 4*y4^2 + 8*z1^2 + 8*z2^2 + z1^4 + 8*z3^2 + z2^4 + 8*z4^2 + z3^4 + z4^4 - 2*x1*x2*y1*y2 - 2*x1*x3*y1*y3 - 2*x1*x4*y1*y4 - 2*x2*x3*y2*y3 - 2*x2*x4*y2*y4 - 2*x3*x4*y3*y4 + 16))/(8*x1^2*x2^2 + 8*x1^2*x3^2 + 8*x1^2*x4^2 + 8*x2^2*x3^2 + 8*x2^2*x4^2 + 8*x3^2*x4^2 + 8*x1^2*y1^2 + 12*x1^2*y2^2 + 12*x2^2*y1^2 + 12*x1^2*y3^2 + 8*x2^2*y2^2 + 12*x3^2*y1^2 + x1^2*y2^4 + 12*x1^2*y4^2 + x2^2*y1^4 + 12*x2^2*y3^2 + x1^4*y2^2 + 12*x3^2*y2^2 + x2^4*y1^2 + 12*x4^2*y1^2 + x1^2*y3^4 + 12*x2^2*y4^2 + x1^4*y3^2 + x3^2*y1^4 + 8*x3^2*y3^2 + 12*x4^2*y2^2 + x3^4*y1^2 + x1^2*y4^4 + x2^2*y3^4 + x1^4*y4^2 + x3^2*y2^4 + 12*x3^2*y4^2 + x2^4*y3^2 + x4^2*y1^4 + 12*x4^2*y3^2 + x3^4*y2^2 + x4^4*y1^2 + x2^2*y4^4 + x2^4*y4^2 + x4^2*y2^4 + 8*x4^2*y4^2 + x4^4*y2^2 + x3^2*y4^4 + x4^2*y3^4 + x3^4*y4^2 + x4^4*y3^2 + 8*x1^2*z1^2 + 12*x1^2*z2^2 + 12*x2^2*z1^2 + 8*y1^2*y2^2 + 12*x1^2*z3^2 + 8*x2^2*z2^2 + 12*x3^2*z1^2 + 8*y1^2*y3^2 + x1^2*z2^4 + 12*x1^2*z4^2 + x2^2*z1^4 + 12*x2^2*z3^2 + x1^4*z2^2 + 12*x3^2*z2^2 + x2^4*z1^2 + 12*x4^2*z1^2 + 8*y1^2*y4^2 + 8*y2^2*y3^2 + x1^2*z3^4 + 12*x2^2*z4^2 + x1^4*z3^2 + x3^2*z1^4 + 8*x3^2*z3^2 + 12*x4^2*z2^2 + x3^4*z1^2 + 8*y2^2*y4^2 + x1^2*z4^4 + x2^2*z3^4 + x1^4*z4^2 + x3^2*z2^4 + 12*x3^2*z4^2 + x2^4*z3^2 + x4^2*z1^4 + 12*x4^2*z3^2 + x3^4*z2^2 + x4^4*z1^2 + 8*y3^2*y4^2 + x2^2*z4^4 + x2^4*z4^2 + x4^2*z2^4 + 8*x4^2*z4^2 + x4^4*z2^2 + x3^2*z4^4 + x4^2*z3^4 + x3^4*z4^2 + x4^4*z3^2 + 8*y1^2*z1^2 + 12*y1^2*z2^2 + 12*y2^2*z1^2 + 12*y1^2*z3^2 + 8*y2^2*z2^2 + 12*y3^2*z1^2 + y1^2*z2^4 + 12*y1^2*z4^2 + y2^2*z1^4 + 12*y2^2*z3^2 + y1^4*z2^2 + 12*y3^2*z2^2 + y2^4*z1^2 + 12*y4^2*z1^2 + y1^2*z3^4 + 12*y2^2*z4^2 + y1^4*z3^2 + y3^2*z1^4 + 8*y3^2*z3^2 + 12*y4^2*z2^2 + y3^4*z1^2 + y1^2*z4^4 + y2^2*z3^4 + y1^4*z4^2 + y3^2*z2^4 + 12*y3^2*z4^2 + y2^4*z3^2 + y4^2*z1^4 + 12*y4^2*z3^2 + y3^4*z2^2 + y4^4*z1^2 + y2^2*z4^4 + y2^4*z4^2 + y4^2*z2^4 + 8*y4^2*z4^2 + y4^4*z2^2 + y3^2*z4^4 + y4^2*z3^4 + y3^4*z4^2 + y4^4*z3^2 + 8*z1^2*z2^2 + 8*z1^2*z3^2 + 8*z1^2*z4^2 + 8*z2^2*z3^2 + 8*z2^2*z4^2 + 8*z3^2*z4^2 + 32*x1^2 + 32*x2^2 + 4*x1^4 + 32*x3^2 + 4*x2^4 + 32*x4^2 + 4*x3^4 + 4*x4^4 + 32*y1^2 + 32*y2^2 + 4*y1^4 + 32*y3^2 + 4*y2^4 + 32*y4^2 + 4*y3^4 + 4*y4^4 + 32*z1^2 + 32*z2^2 + 4*z1^4 + 32*z3^2 + 4*z2^4 + 32*z4^2 + 4*z3^4 + 4*z4^4 + x1^2*x2^2*y1^2 + x1^2*x2^2*y2^2 + x1^2*x3^2*y1^2 + 2*x1^2*x2^2*y3^2 + 2*x1^2*x3^2*y2^2 + x1^2*x4^2*y1^2 + 2*x2^2*x3^2*y1^2 + 2*x1^2*x2^2*y4^2 + x1^2*x3^2*y3^2 + 2*x1^2*x4^2*y2^2 + x2^2*x3^2*y2^2 + 2*x2^2*x4^2*y1^2 + 2*x1^2*x3^2*y4^2 + 2*x1^2*x4^2*y3^2 + x2^2*x3^2*y3^2 + x2^2*x4^2*y2^2 + 2*x3^2*x4^2*y1^2 + x1^2*x4^2*y4^2 + 2*x2^2*x3^2*y4^2 + 2*x2^2*x4^2*y3^2 + 2*x3^2*x4^2*y2^2 + x2^2*x4^2*y4^2 + x3^2*x4^2*y3^2 + x3^2*x4^2*y4^2 + x1^2*x2^2*z1^2 + x1^2*y1^2*y2^2 + x1^2*x2^2*z2^2 + x1^2*x3^2*z1^2 + x1^2*y1^2*y3^2 + x2^2*y1^2*y2^2 + 2*x1^2*x2^2*z3^2 + 2*x1^2*x3^2*z2^2 + x1^2*x4^2*z1^2 + x1^2*y1^2*y4^2 + 2*x1^2*y2^2*y3^2 + 2*x2^2*x3^2*z1^2 + 2*x2^2*y1^2*y3^2 + 2*x3^2*y1^2*y2^2 + 2*x1^2*x2^2*z4^2 + x1^2*x3^2*z3^2 + 2*x1^2*x4^2*z2^2 + 2*x1^2*y2^2*y4^2 + x2^2*x3^2*z2^2 + 2*x2^2*x4^2*z1^2 + 2*x2^2*y1^2*y4^2 + x2^2*y2^2*y3^2 + x3^2*y1^2*y3^2 + 2*x4^2*y1^2*y2^2 + 2*x1^2*x3^2*z4^2 + 2*x1^2*x4^2*z3^2 + 2*x1^2*y3^2*y4^2 + x2^2*x3^2*z3^2 + x2^2*x4^2*z2^2 + x2^2*y2^2*y4^2 + 2*x3^2*x4^2*z1^2 + 2*x3^2*y1^2*y4^2 + x3^2*y2^2*y3^2 + 2*x4^2*y1^2*y3^2 + x1^2*x4^2*z4^2 + 2*x2^2*x3^2*z4^2 + 2*x2^2*x4^2*z3^2 + 2*x2^2*y3^2*y4^2 + 2*x3^2*x4^2*z2^2 + 2*x3^2*y2^2*y4^2 + x4^2*y1^2*y4^2 + 2*x4^2*y2^2*y3^2 + x2^2*x4^2*z4^2 + x3^2*x4^2*z3^2 + x3^2*y3^2*y4^2 + x4^2*y2^2*y4^2 + x3^2*x4^2*z4^2 + x4^2*y3^2*y4^2 + 2*x1^2*y1^2*z2^2 + 2*x1^2*y2^2*z1^2 + 2*x2^2*y1^2*z1^2 + 2*x1^2*y1^2*z3^2 + 2*x1^2*y2^2*z2^2 + 2*x1^2*y3^2*z1^2 + 2*x2^2*y1^2*z2^2 + 2*x2^2*y2^2*z1^2 + 2*x3^2*y1^2*z1^2 + 2*x1^2*y1^2*z4^2 + 2*x1^2*y2^2*z3^2 + 2*x1^2*y3^2*z2^2 + 2*x1^2*y4^2*z1^2 + 2*x2^2*y1^2*z3^2 + 2*x2^2*y3^2*z1^2 + 2*x3^2*y1^2*z2^2 + 2*x3^2*y2^2*z1^2 + 2*x4^2*y1^2*z1^2 + 2*x1^2*y2^2*z4^2 + 2*x1^2*y3^2*z3^2 + 2*x1^2*y4^2*z2^2 + 2*x2^2*y1^2*z4^2 + 2*x2^2*y2^2*z3^2 + 2*x2^2*y3^2*z2^2 + 2*x2^2*y4^2*z1^2 + 2*x3^2*y1^2*z3^2 + 2*x3^2*y2^2*z2^2 + 2*x3^2*y3^2*z1^2 + 2*x4^2*y1^2*z2^2 + 2*x4^2*y2^2*z1^2 + 2*x1^2*y3^2*z4^2 + 2*x1^2*y4^2*z3^2 + 2*x2^2*y2^2*z4^2 + 2*x2^2*y3^2*z3^2 + 2*x2^2*y4^2*z2^2 + 2*x3^2*y1^2*z4^2 + 2*x3^2*y2^2*z3^2 + 2*x3^2*y3^2*z2^2 + 2*x3^2*y4^2*z1^2 + 2*x4^2*y1^2*z3^2 + 2*x4^2*y2^2*z2^2 + 2*x4^2*y3^2*z1^2 + 2*x1^2*y4^2*z4^2 + 2*x2^2*y3^2*z4^2 + 2*x2^2*y4^2*z3^2 + 2*x3^2*y2^2*z4^2 + 2*x3^2*y4^2*z2^2 + 2*x4^2*y1^2*z4^2 + 2*x4^2*y2^2*z3^2 + 2*x4^2*y3^2*z2^2 + 2*x4^2*y4^2*z1^2 + 2*x2^2*y4^2*z4^2 + 2*x3^2*y3^2*z4^2 + 2*x3^2*y4^2*z3^2 + 2*x4^2*y2^2*z4^2 + 2*x4^2*y3^2*z3^2 + 2*x4^2*y4^2*z2^2 + 2*x3^2*y4^2*z4^2 + 2*x4^2*y3^2*z4^2 + 2*x4^2*y4^2*z3^2 + x1^2*z1^2*z2^2 + y1^2*y2^2*z1^2 + x1^2*z1^2*z3^2 + x2^2*z1^2*z2^2 + y1^2*y2^2*z2^2 + y1^2*y3^2*z1^2 + x1^2*z1^2*z4^2 + 2*x1^2*z2^2*z3^2 + 2*x2^2*z1^2*z3^2 + 2*x3^2*z1^2*z2^2 + 2*y1^2*y2^2*z3^2 + 2*y1^2*y3^2*z2^2 + y1^2*y4^2*z1^2 + 2*y2^2*y3^2*z1^2 + 2*x1^2*z2^2*z4^2 + 2*x2^2*z1^2*z4^2 + x2^2*z2^2*z3^2 + x3^2*z1^2*z3^2 + 2*x4^2*z1^2*z2^2 + 2*y1^2*y2^2*z4^2 + y1^2*y3^2*z3^2 + 2*y1^2*y4^2*z2^2 + y2^2*y3^2*z2^2 + 2*y2^2*y4^2*z1^2 + 2*x1^2*z3^2*z4^2 + x2^2*z2^2*z4^2 + 2*x3^2*z1^2*z4^2 + x3^2*z2^2*z3^2 + 2*x4^2*z1^2*z3^2 + 2*y1^2*y3^2*z4^2 + 2*y1^2*y4^2*z3^2 + y2^2*y3^2*z3^2 + y2^2*y4^2*z2^2 + 2*y3^2*y4^2*z1^2 + 2*x2^2*z3^2*z4^2 + 2*x3^2*z2^2*z4^2 + x4^2*z1^2*z4^2 + 2*x4^2*z2^2*z3^2 + y1^2*y4^2*z4^2 + 2*y2^2*y3^2*z4^2 + 2*y2^2*y4^2*z3^2 + 2*y3^2*y4^2*z2^2 + x3^2*z3^2*z4^2 + x4^2*z2^2*z4^2 + y2^2*y4^2*z4^2 + y3^2*y4^2*z3^2 + x4^2*z3^2*z4^2 + y3^2*y4^2*z4^2 + y1^2*z1^2*z2^2 + y1^2*z1^2*z3^2 + y2^2*z1^2*z2^2 + y1^2*z1^2*z4^2 + 2*y1^2*z2^2*z3^2 + 2*y2^2*z1^2*z3^2 + 2*y3^2*z1^2*z2^2 + 2*y1^2*z2^2*z4^2 + 2*y2^2*z1^2*z4^2 + y2^2*z2^2*z3^2 + y3^2*z1^2*z3^2 + 2*y4^2*z1^2*z2^2 + 2*y1^2*z3^2*z4^2 + y2^2*z2^2*z4^2 + 2*y3^2*z1^2*z4^2 + y3^2*z2^2*z3^2 + 2*y4^2*z1^2*z3^2 + 2*y2^2*z3^2*z4^2 + 2*y3^2*z2^2*z4^2 + y4^2*z1^2*z4^2 + 2*y4^2*z2^2*z3^2 + y3^2*z3^2*z4^2 + y4^2*z2^2*z4^2 + y4^2*z3^2*z4^2 - 8*x1*x2*y1*y2 - 8*x1*x3*y1*y3 - 8*x1*x4*y1*y4 - 8*x2*x3*y2*y3 - 8*x2*x4*y2*y4 - 8*x3*x4*y3*y4 - 8*x1*x2*z1*z2 - 8*x1*x3*z1*z3 - 8*x1*x4*z1*z4 - 8*x2*x3*z2*z3 - 8*x2*x4*z2*z4 - 8*x3*x4*z3*z4 - 8*y1*y2*z1*z2 - 8*y1*y3*z1*z3 - 8*y1*y4*z1*z4 - 8*y2*y3*z2*z3 - 8*y2*y4*z2*z4 - 8*y3*y4*z3*z4 - 2*x1*x2*y1*y2^3 - 2*x1*x2*y1^3*y2 - 2*x1*x2^3*y1*y2 - 2*x1^3*x2*y1*y2 - 2*x1*x3*y1*y3^3 - 2*x1*x3*y1^3*y3 - 2*x1*x3^3*y1*y3 - 2*x1^3*x3*y1*y3 - 2*x1*x4*y1*y4^3 - 2*x1*x4*y1^3*y4 - 2*x1*x4^3*y1*y4 - 2*x2*x3*y2*y3^3 - 2*x2*x3*y2^3*y3 - 2*x2*x3^3*y2*y3 - 2*x1^3*x4*y1*y4 - 2*x2^3*x3*y2*y3 - 2*x2*x4*y2*y4^3 - 2*x2*x4*y2^3*y4 - 2*x2*x4^3*y2*y4 - 2*x2^3*x4*y2*y4 - 2*x3*x4*y3*y4^3 - 2*x3*x4*y3^3*y4 - 2*x3*x4^3*y3*y4 - 2*x3^3*x4*y3*y4 - 2*x1*x2*z1*z2^3 - 2*x1*x2*z1^3*z2 - 2*x1*x2^3*z1*z2 - 2*x1^3*x2*z1*z2 - 2*x1*x3*z1*z3^3 - 2*x1*x3*z1^3*z3 - 2*x1*x3^3*z1*z3 - 2*x1^3*x3*z1*z3 - 2*x1*x4*z1*z4^3 - 2*x1*x4*z1^3*z4 - 2*x1*x4^3*z1*z4 - 2*x2*x3*z2*z3^3 - 2*x2*x3*z2^3*z3 - 2*x2*x3^3*z2*z3 - 2*x1^3*x4*z1*z4 - 2*x2^3*x3*z2*z3 - 2*x2*x4*z2*z4^3 - 2*x2*x4*z2^3*z4 - 2*x2*x4^3*z2*z4 - 2*x2^3*x4*z2*z4 - 2*x3*x4*z3*z4^3 - 2*x3*x4*z3^3*z4 - 2*x3*x4^3*z3*z4 - 2*x3^3*x4*z3*z4 - 2*y1*y2*z1*z2^3 - 2*y1*y2*z1^3*z2 - 2*y1*y2^3*z1*z2 - 2*y1^3*y2*z1*z2 - 2*y1*y3*z1*z3^3 - 2*y1*y3*z1^3*z3 - 2*y1*y3^3*z1*z3 - 2*y1^3*y3*z1*z3 - 2*y1*y4*z1*z4^3 - 2*y1*y4*z1^3*z4 - 2*y1*y4^3*z1*z4 - 2*y2*y3*z2*z3^3 - 2*y2*y3*z2^3*z3 - 2*y2*y3^3*z2*z3 - 2*y1^3*y4*z1*z4 - 2*y2^3*y3*z2*z3 - 2*y2*y4*z2*z4^3 - 2*y2*y4*z2^3*z4 - 2*y2*y4^3*z2*z4 - 2*y2^3*y4*z2*z4 - 2*y3*y4*z3*z4^3 - 2*y3*y4*z3^3*z4 - 2*y3*y4^3*z3*z4 - 2*y3^3*y4*z3*z4 - 2*x1*x2*x3^2*y1*y2 - 2*x1*x2*x4^2*y1*y2 - 2*x1*x2^2*x3*y1*y3 - 2*x1^2*x2*x3*y2*y3 - 2*x1*x3*x4^2*y1*y3 - 2*x1*x2^2*x4*y1*y4 - 2*x1*x3^2*x4*y1*y4 - 2*x1^2*x2*x4*y2*y4 - 2*x2*x3*x4^2*y2*y3 - 2*x2*x3^2*x4*y2*y4 - 2*x1^2*x3*x4*y3*y4 - 2*x2^2*x3*x4*y3*y4 - 2*x1*x2*y1*y2*y3^2 - 2*x1*x2*y1*y2*y4^2 - 2*x1*x3*y1*y2^2*y3 - 2*x2*x3*y1^2*y2*y3 - 2*x1*x3*y1*y3*y4^2 - 2*x1*x4*y1*y2^2*y4 - 2*x1*x4*y1*y3^2*y4 - 2*x2*x4*y1^2*y2*y4 - 2*x2*x3*y2*y3*y4^2 - 2*x2*x4*y2*y3^2*y4 - 2*x3*x4*y1^2*y3*y4 - 2*x3*x4*y2^2*y3*y4 - 2*x1*x2*y1*y2*z1^2 - 2*x1*x2*y1*y2*z2^2 - 2*x1*x2*x3^2*z1*z2 - 2*x1*x3*y1*y3*z1^2 - 2*x1*x2*x4^2*z1*z2 - 2*x1*x2^2*x3*z1*z3 - 2*x1*x3*y1*y3*z3^2 - 2*x1*x4*y1*y4*z1^2 - 2*x1^2*x2*x3*z2*z3 - 2*x1*x3*x4^2*z1*z3 - 2*x1*x2^2*x4*z1*z4 - 2*x2*x3*y2*y3*z2^2 - 2*x1*x3^2*x4*z1*z4 - 2*x2*x3*y2*y3*z3^2 - 2*x1^2*x2*x4*z2*z4 - 2*x1*x4*y1*y4*z4^2 - 2*x2*x3*x4^2*z2*z3 - 2*x2*x4*y2*y4*z2^2 - 2*x2*x3^2*x4*z2*z4 - 2*x1^2*x3*x4*z3*z4 - 2*x2*x4*y2*y4*z4^2 - 2*x2^2*x3*x4*z3*z4 - 2*x3*x4*y3*y4*z3^2 - 2*x3*x4*y3*y4*z4^2 - 2*x1*x2*y1^2*z1*z2 - 2*x1*x2*y2^2*z1*z2 - 2*x1*x3*y1^2*z1*z3 - 2*x1*x3*y3^2*z1*z3 - 2*x1*x4*y1^2*z1*z4 - 2*x2*x3*y2^2*z2*z3 - 2*x2*x3*y3^2*z2*z3 - 2*x1*x4*y4^2*z1*z4 - 2*x2*x4*y2^2*z2*z4 - 2*x2*x4*y4^2*z2*z4 - 2*x3*x4*y3^2*z3*z4 - 2*x3*x4*y4^2*z3*z4 - 2*x1^2*y1*y2*z1*z2 - 2*x2^2*y1*y2*z1*z2 - 2*x1*x2*z1*z2*z3^2 - 2*x1^2*y1*y3*z1*z3 - 2*x1*x2*z1*z2*z4^2 - 2*x1*x3*z1*z2^2*z3 - 2*x2*x3*z1^2*z2*z3 - 2*x1^2*y1*y4*z1*z4 - 2*x3^2*y1*y3*z1*z3 - 2*x1*x3*z1*z3*z4^2 - 2*x1*x4*z1*z2^2*z4 - 2*x2^2*y2*y3*z2*z3 - 2*x1*x4*z1*z3^2*z4 - 2*x2*x4*z1^2*z2*z4 - 2*x3^2*y2*y3*z2*z3 - 2*x2*x3*z2*z3*z4^2 - 2*x2^2*y2*y4*z2*z4 - 2*x4^2*y1*y4*z1*z4 - 2*x2*x4*z2*z3^2*z4 - 2*x3*x4*z1^2*z3*z4 - 2*x3*x4*z2^2*z3*z4 - 2*x4^2*y2*y4*z2*z4 - 2*x3^2*y3*y4*z3*z4 - 2*x4^2*y3*y4*z3*z4 - 2*y1*y2*y3^2*z1*z2 - 2*y1*y2*y4^2*z1*z2 - 2*y1*y2^2*y3*z1*z3 - 2*y1^2*y2*y3*z2*z3 - 2*y1*y3*y4^2*z1*z3 - 2*y1*y2^2*y4*z1*z4 - 2*y1*y3^2*y4*z1*z4 - 2*y1^2*y2*y4*z2*z4 - 2*y2*y3*y4^2*z2*z3 - 2*y2*y3^2*y4*z2*z4 - 2*y1^2*y3*y4*z3*z4 - 2*y2^2*y3*y4*z3*z4 - 2*y1*y2*z1*z2*z3^2 - 2*y1*y2*z1*z2*z4^2 - 2*y1*y3*z1*z2^2*z3 - 2*y2*y3*z1^2*z2*z3 - 2*y1*y3*z1*z3*z4^2 - 2*y1*y4*z1*z2^2*z4 - 2*y1*y4*z1*z3^2*z4 - 2*y2*y4*z1^2*z2*z4 - 2*y2*y3*z2*z3*z4^2 - 2*y2*y4*z2*z3^2*z4 - 2*y3*y4*z1^2*z3*z4 - 2*y3*y4*z2^2*z3*z4 - 2*x1*x2*y1*y3*z2*z3 - 2*x1*x2*y2*y3*z1*z3 - 2*x1*x3*y1*y2*z2*z3 - 2*x1*x3*y2*y3*z1*z2 - 2*x2*x3*y1*y2*z1*z3 - 2*x2*x3*y1*y3*z1*z2 - 2*x1*x2*y1*y4*z2*z4 - 2*x1*x2*y2*y4*z1*z4 - 2*x1*x4*y1*y2*z2*z4 - 2*x1*x4*y2*y4*z1*z2 - 2*x2*x4*y1*y2*z1*z4 - 2*x2*x4*y1*y4*z1*z2 - 2*x1*x3*y1*y4*z3*z4 - 2*x1*x3*y3*y4*z1*z4 - 2*x1*x4*y1*y3*z3*z4 - 2*x1*x4*y3*y4*z1*z3 - 2*x3*x4*y1*y3*z1*z4 - 2*x3*x4*y1*y4*z1*z3 - 2*x2*x3*y2*y4*z3*z4 - 2*x2*x3*y3*y4*z2*z4 - 2*x2*x4*y2*y3*z3*z4 - 2*x2*x4*y3*y4*z2*z3 - 2*x3*x4*y2*y3*z2*z4 - 2*x3*x4*y2*y4*z2*z3 + 64)];




Ginv = 0.25*[eye(3) J4inv*skew_sm(quatrot(x(4:7),r(1:3)))';
             zeros(3) J4inv;
             eye(3) J4inv*skew_sm(quatrot(x(4:7),r(4:6)))';
             zeros(3) J4inv;
             eye(3) J4inv*skew_sm(quatrot(x(4:7),r(7:9)))';
             zeros(3) J4inv;
             eye(3) J4inv*skew_sm(quatrot(x(4:7),r(10:12)))';
             zeros(3) J4inv];
